simulink model "lagrange_model"  (R2022a)
settings: Solver=ode4  StartTime=0.0  StopTime=10.0  FixedStep=0.01  RelTol=1e-3
undefined symbols (not defined in the file or in its folder): DiscIntNeverNeededParam
(part 3 of 5)

== matlab function lagrange_model/MATLAB Function ==
  data: u1 input; th1dd output; u2 input double; u3 input; u4 input; u5 input; th1d input; th2d input; th3d input; th4d input; th5d input; th2dd output; th3dd output; th4dd output; th5dd output; th1 input; th2 input; th3 input; th4 input; th5 input; th1dd input; th2dd input; th3dd input; th4dd input; th5dd input
function [th1dd, th2dd, th3dd, th4dd, th5dd]= fcn(u1, u2, u3, u4, u5, th1d, th2d, th3d, th4d, th5d, th1, th2, th3, th4, th5, th1dd, th2dd, th3dd, th4dd, th5dd)

l1 = 0.135; 
l2 = 0.38;
l3 = 0.38;
l4 = 0.38;
l5 = 0.04;

m1 = 2.24036308689963;
m2 = 1.38058358126134;
m3 = 0.492773406896242;
m4 = 1.38058358126134;
m5 = 0.130378439395373;
delta = 0.0873;
l1_Izz = 0.0098329939500295;
l2_Izz = 0.0425687229272136;
l3_Izz = 0.00857639886635598;
l4_Izz = 0.0422407814003671;
l5_Izz = 0.0001866513337855;

g = 9.81;
beta1 = 0.3;
beta2 = 0.1;
beta3 = 0.1;
beta4 = 0.1;
beta5 = 0.1;

eq1 = l1_Izz*diff(th1(t), t, t) + l2_Izz*diff(th1(t), t, t) + l3_Izz*diff(th1(t), t, t) + l4_Izz*diff(th1(t), t, t) + l5_Izz*diff(th1(t), t, t) + beta1*diff(th1(t), t) + (l2^2*m2*cos(th1(t))^2*cos(th2(t))^2*diff(th1(t), t, t))/4 + l2^2*m3*cos(th1(t))^2*cos(th2(t))^2*diff(th1(t), t, t) + l2^2*m4*cos(th1(t))^2*cos(th2(t))^2*diff(th1(t), t, t) + l2^2*m5*cos(th1(t))^2*cos(th2(t))^2*diff(th1(t), t, t) + (l2^2*m2*cos(th2(t))^2*sin(th1(t))^2*diff(th1(t), t, t))/4 + l2^2*m3*cos(th2(t))^2*sin(th1(t))^2*diff(th1(t), t, t) + l2^2*m4*cos(th2(t))^2*sin(th1(t))^2*diff(th1(t), t, t) + l2^2*m5*cos(th2(t))^2*sin(th1(t))^2*diff(th1(t), t, t) + (l3^2*m3*cos(th1(t))^2*cos(th2(t))^2*sin(th3(t))^2*diff(th1(t), t, t))/4 + l3^2*m4*cos(th1(t))^2*cos(th2(t))^2*sin(th3(t))^2*diff(th1(t), t, t) + l3^2*m5*cos(th1(t))^2*cos(th2(t))^2*sin(th3(t))^2*diff(th1(t), t, t) + (l3^2*m3*cos(th2(t))^2*sin(th1(t))^2*sin(th3(t))^2*diff(th1(t), t, t))/4 + l3^2*m4*cos(th2(t))^2*sin(th1(t))^2*sin(th3(t))^2*diff(th1(t), t, t) + l3^2*m5*cos(th2(t))^2*sin(th1(t))^2*sin(th3(t))^2*diff(th1(t), t, t) - (l2^2*m2*cos(th1(t))^2*cos(th2(t))*sin(th2(t))*diff(th1(t), t)*diff(th2(t), t))/2 - 2*l2^2*m3*cos(th1(t))^2*cos(th2(t))*sin(th2(t))*diff(th1(t), t)*diff(th2(t), t) - 2*l2^2*m4*cos(th1(t))^2*cos(th2(t))*sin(th2(t))*diff(th1(t), t)*diff(th2(t), t) - 2*l2^2*m5*cos(th1(t))^2*cos(th2(t))*sin(th2(t))*diff(th1(t), t)*diff(th2(t), t) - (l2^2*m2*cos(th2(t))*sin(th1(t))^2*sin(th2(t))*diff(th1(t), t)*diff(th2(t), t))/2 - 2*l2^2*m3*cos(th2(t))*sin(th1(t))^2*sin(th2(t))*diff(th1(t), t)*diff(th2(t), t) - 2*l2^2*m4*cos(th2(t))*sin(th1(t))^2*sin(th2(t))*diff(th1(t), t)*diff(th2(t), t) - 2*l2^2*m5*cos(th2(t))*sin(th1(t))^2*sin(th2(t))*diff(th1(t), t)*diff(th2(t), t) + l2*l3*m3*cos(th1(t))^2*cos(th2(t))^2*sin(th3(t))*diff(th1(t), t, t) + 2*l2*l3*m4*cos(th1(t))^2*cos(th2(t))^2*sin(th3(t))*diff(th1(t), t, t) + 2*l2*l3*m5*cos(th1(t))^2*cos(th2(t))^2*sin(th3(t))*diff(th1(t), t, t) - (l4^2*m5*cos(th1(t))^2*cos(th2(t))^2*sin(th3(t))^2*cos(delta - th4(t))^2*diff(th1(t), t)^2)/4 - (l4^2*m5*cos(th1(t))^2*cos(th2(t))^2*sin(th3(t))^2*cos(delta - th4(t))^2*diff(th2(t), t)^2)/4 - (l4^2*m5*cos(th1(t))^2*cos(th2(t))^2*sin(th3(t))^2*cos(delta - th4(t))^2*diff(th3(t), t)^2)/4 - (l4^2*m5*cos(th1(t))^2*cos(th2(t))^2*sin(th3(t))^2*cos(delta - th4(t))^2*diff(th4(t), t)^2)/4 + l2*l3*m3*cos(th2(t))^2*sin(th1(t))^2*sin(th3(t))*diff(th1(t), t, t) + 2*l2*l3*m4*cos(th2(t))^2*sin(th1(t))^2*sin(th3(t))*diff(th1(t), t, t) + 2*l2*l3*m5*cos(th2(t))^2*sin(th1(t))^2*sin(th3(t))*diff(th1(t), t, t) + (l4^2*m5*cos(th2(t))^2*sin(th1(t))^2*sin(th3(t))^2*cos(delta - th4(t))^2*diff(th1(t), t)^2)/4 + (l4^2*m5*cos(th2(t))^2*sin(th1(t))^2*sin(th3(t))^2*cos(delta - th4(t))^2*diff(th2(t), t)^2)/4 + (l4^2*m5*cos(th2(t))^2*sin(th1(t))^2*sin(th3(t))^2*cos(delta - th4(t))^2*diff(th3(t), t)^2)/4 + (l4^2*m5*cos(th2(t))^2*sin(th1(t))^2*sin(th3(t))^2*cos(delta - th4(t))^2*diff(th4(t), t)^2)/4 + (l4^2*m5*cos(th1(t))^2*cos(th2(t))^2*sin(th3(t))^2*cos(delta - th4(t))^2*diff(th1(t), t, t))/4 + (l4^2*m4*cos(th2(t))^2*sin(th1(t))^2*sin(th3(t))^2*cos(delta - th4(t))^2*diff(th1(t), t, t))/2 + (5*l4^2*m5*cos(th2(t))^2*sin(th1(t))^2*sin(th3(t))^2*cos(delta - th4(t))^2*diff(th1(t), t, t))/4 - l2*l4*m4*cos(th2(t))^2*sin(th1(t))^2*sin(th3(t))*cos(delta - th4(t))*diff(th1(t), t, t) - 2*l2*l4*m5*cos(th2(t))^2*sin(th1(t))^2*sin(th3(t))*cos(delta - th4(t))*diff(th1(t), t, t) + (l2*l4*m4*cos(th1(t))^2*cos(th2(t))^2*sin(th3(t))*sin(delta - th4(t))*diff(th4(t), t, t))/2 + (l2*l4*m5*cos(th1(t))^2*cos(th2(t))^2*sin(th3(t))*sin(delta - th4(t))*diff(th4(t), t, t))/2 + (l3^2*m3*cos(th1(t))^2*cos(th2(t))^2*cos(th3(t))*sin(th3(t))*diff(th1(t), t)*diff(th3(t), t))/2 + 2*l3^2*m4*cos(th1(t))^2*cos(th2(t))^2*cos(th3(t))*sin(th3(t))*diff(th1(t), t)*diff(th3(t), t) + 2*l3^2*m5*cos(th1(t))^2*cos(th2(t))^2*cos(th3(t))*sin(th3(t))*diff(th1(t), t)*diff(th3(t), t) - (l3^2*m3*cos(th1(t))^2*cos(th2(t))*sin(th2(t))*sin(th3(t))^2*diff(th1(t), t)*diff(th2(t), t))/2 - 2*l3^2*m4*cos(th1(t))^2*cos(th2(t))*sin(th2(t))*sin(th3(t))^2*diff(th1(t), t)*diff(th2(t), t) + (l3^2*m3*cos(th2(t))^2*cos(th3(t))*sin(th1(t))^2*sin(th3(t))*diff(th1(t), t)*diff(th3(t), t))/2 - 2*l3^2*m5*cos(th1(t))^2*cos(th2(t))*sin(th2(t))*sin(th3(t))^2*diff(th1(t), t)*diff(th2(t), t) + 2*l3^2*m4*cos(th2(t))^2*cos(th3(t))*sin(th1(t))^2*sin(th3(t))*diff(th1(t), t)*diff(th3(t), t) + 2*l3^2*m5*cos(th2(t))^2*cos(th3(t))*sin(th1(t))^2*sin(th3(t))*diff(th1(t), t)*diff(th3(t), t) - (l3^2*m3*cos(th2(t))*sin(th1(t))^2*sin(th2(t))*sin(th3(t))^2*diff(th1(t), t)*diff(th2(t), t))/2 - 2*l3^2*m4*cos(th2(t))*sin(th1(t))^2*sin(th2(t))*sin(th3(t))^2*diff(th1(t), t)*diff(th2(t), t) - 2*l3^2*m5*cos(th2(t))*sin(th1(t))^2*sin(th2(t))*sin(th3(t))^2*diff(th1(t), t)*diff(th2(t), t) - (l3*l4*m4*cos(th1(t))^2*cos(th2(t))^2*sin(th3(t))^2*cos(delta - th4(t))*diff(th1(t), t)^2)/2 - (l3*l4*m4*cos(th1(t))^2*cos(th2(t))^2*sin(th3(t))^2*cos(delta - th4(t))*diff(th2(t), t)^2)/2 - (l3*l4*m5*cos(th1(t))^2*cos(th2(t))^2*sin(th3(t))^2*cos(delta - th4(t))*diff(th1(t), t)^2)/2 - (l3*l4*m4*cos(th1(t))^2*cos(th2(t))^2*sin(th3(t))^2*cos(delta - th4(t))*diff(th3(t), t)^2)/2 - (l3*l4*m5*cos(th1(t))^2*cos(th2(t))^2*sin(th3(t))^2*cos(delta - th4(t))*diff(th2(t), t)^2)/2 - (l3*l4*m4*cos(th1(t))^2*cos(th2(t))^2*sin(th3(t))^2*cos(delta - th4(t))*diff(th4(t), t)^2)/2 - (l3*l4*m5*cos(th1(t))^2*cos(th2(t))^2*sin(th3(t))^2*cos(delta - th4(t))*diff(th3(t), t)^2)/2 - (l3*l4*m5*cos(th1(t))^2*cos(th2(t))^2*sin(th3(t))^2*cos(delta - th4(t))*diff(th4(t), t)^2)/2 + (l3*l4*m4*cos(th2(t))^2*sin(th1(t))^2*sin(th3(t))^2*cos(delta - th4(t))*diff(th1(t), t)^2)/2 + (l3*l4*m4*cos(th2(t))^2*sin(th1(t))^2*sin(th3(t))^2*cos(delta - th4(t))*diff(th2(t), t)^2)/2 + (l3*l4*m5*cos(th2(t))^2*sin(th1(t))^2*sin(th3(t))^2*cos(delta - th4(t))*diff(th1(t), t)^2)/2 + (l3*l4*m4*cos(th2(t))^2*sin(th1(t))^2*sin(th3(t))^2*cos(delta - th4(t))*diff(th3(t), t)^2)/2 + (l3*l4*m5*cos(th2(t))^2*sin(th1(t))^2*sin(th3(t))^2*cos(delta - th4(t))*diff(th2(t), t)^2)/2 + (l3*l4*m5*cos(th2(t))^2*sin(th1(t))^2*sin(th3(t))^2*cos(delta - th4(t))*diff(th3(t), t)^2)/2 + (l5^2*m5*cos(th1(t))^2*cos(th2(t))^2*cos(th5(t))^2*sin(th3(t))^2*cos(delta - th4(t))^2*diff(th1(t), t, t))/4 + l3*l4*m5*cos(th1(t))^2*cos(th2(t))^2*sin(th3(t))^2*cos(delta - th4(t))*diff(th1(t), t, t) + (l5^2*m5*cos(th2(t))^2*cos(th5(t))^2*sin(th1(t))^2*sin(th3(t))^2*cos(delta - th4(t))^2*diff(th1(t), t, t))/4 - l3*l4*m4*cos(th2(t))^2*sin(th1(t))^2*sin(th3(t))^2*cos(delta - th4(t))*diff(th1(t), t, t) - 2*l3*l4*m5*cos(th2(t))^2*sin(th1(t))^2*sin(th3(t))^2*cos(delta - th4(t))*diff(th1(t), t, t) + (l3*l4*m4*cos(th1(t))^2*cos(th2(t))^2*sin(th3(t))^2*sin(delta - th4(t))*diff(th4(t), t, t))/2 + (l3*l4*m5*cos(th1(t))^2*cos(th2(t))^2*sin(th3(t))^2*sin(delta - th4(t))*diff(th4(t), t, t))/2 + (l4^2*m4*cos(th1(t))*cos(th2(t))^2*sin(th1(t))*sin(th3(t))^2*cos(delta - th4(t))^2*diff(th1(t), t)^2)/2 + (l4^2*m4*cos(th1(t))*cos(th2(t))^2*sin(th1(t))*sin(th3(t))^2*cos(delta - th4(t))^2*diff(th2(t), t)^2)/2 + l4^2*m5*cos(th1(t))*cos(th2(t))^2*sin(th1(t))*sin(th3(t))^2*cos(delta - th4(t))^2*diff(th1(t), t)^2 + (l4^2*m4*cos(th1(t))*cos(th2(t))^2*sin(th1(t))*sin(th3(t))^2*cos(delta - th4(t))^2*diff(th3(t), t)^2)/2 + l4^2*m5*cos(th1(t))*cos(th2(t))^2*sin(th1(t))*sin(th3(t))^2*cos(delta - th4(t))^2*diff(th2(t), t)^2 + (l4^2*m4*cos(th1(t))*cos(th2(t))^2*sin(th1(t))*sin(th3(t))^2*cos(delta - th4(t))^2*diff(th4(t), t)^2)/2 + l4^2*m5*cos(th1(t))*cos(th2(t))^2*sin(th1(t))*sin(th3(t))^2*cos(delta - th4(t))^2*diff(th3(t), t)^2 + l4^2*m5*cos(th1(t))*cos(th2(t))^2*sin(th1(t))*sin(th3(t))^2*cos(delta - th4(t))^2*diff(th4(t), t)^2 + (l4^2*m5*cos(th1(t))^2*cos(th2(t))^2*cos(th3(t))*sin(th3(t))*cos(delta - th4(t))^2*diff(th3(t), t, t))/4 - (l4^2*m5*cos(th1(t))*cos(th2(t))^2*sin(th1(t))*sin(th3(t))^2*cos(delta - th4(t))^2*diff(th1(t), t, t))/2 - (l4^2*m5*cos(th1(t))^2*cos(th2(t))*sin(th2(t))*sin(th3(t))^2*cos(delta - th4(t))^2*diff(th2(t), t, t))/4 - (l4^2*m5*cos(th2(t))^2*cos(th3(t))*sin(th1(t))^2*sin(th3(t))*cos(delta - th4(t))^2*diff(th3(t), t, t))/4 + (l4^2*m5*cos(th2(t))*sin(th1(t))^2*sin(th2(t))*sin(th3(t))^2*cos(delta - th4(t))^2*diff(th2(t), t, t))/4 + l2*l3*m3*cos(th1(t))^2*cos(th2(t))^2*cos(th3(t))*diff(th1(t), t)*diff(th3(t), t) + 2*l2*l3*m4*cos(th1(t))^2*cos(th2(t))^2*cos(th3(t))*diff(th1(t), t)*diff(th3(t), t) + 2*l2*l3*m5*cos(th1(t))^2*cos(th2(t))^2*cos(th3(t))*diff(th1(t), t)*diff(th3(t), t) + (l4^2*m5*cos(th1(t))^2*cos(th2(t))^2*sin(th3(t))^2*cos(delta - th4(t))*sin(delta - th4(t))*diff(th4(t), t, t))/4 + l2*l3*m3*cos(th2(t))^2*cos(th3(t))*sin(th1(t))^2*diff(th1(t), t)*diff(th3(t), t) + 2*l2*l3*m4*cos(th2(t))^2*cos(th3(t))*sin(th1(t))^2*diff(th1(t), t)*diff(th3(t), t) + 2*l2*l3*m5*cos(th2(t))^2*cos(th3(t))*sin(th1(t))^2*diff(th1(t), t)*diff(th3(t), t) - (l4^2*m5*cos(th2(t))^2*sin(th1(t))^2*sin(th3(t))^2*cos(delta - th4(t))*sin(delta - th4(t))*diff(th4(t), t, t))/4 - (l2*l4*m4*cos(th1(t))^2*cos(th2(t))^2*sin(th3(t))*cos(delta - th4(t))*diff(th1(t), t)^2)/2 - (l2*l4*m4*cos(th1(t))^2*cos(th2(t))^2*sin(th3(t))*cos(delta - th4(t))*diff(th2(t), t)^2)/2 - (l2*l4*m5*cos(th1(t))^2*cos(th2(t))^2*sin(th3(t))*cos(delta - th4(t))*diff(th1(t), t)^2)/2 - (l2*l4*m4*cos(th1(t))^2*cos(th2(t))^2*sin(th3(t))*cos(delta - th4(t))*diff(th3(t), t)^2)/2 - (l2*l4*m5*cos(th1(t))^2*cos(th2(t))^2*sin(th3(t))*cos(delta - th4(t))*diff(th2(t), t)^2)/2 - (l2*l4*m4*cos(th1(t))^2*cos(th2(t))^2*sin(th3(t))*cos(delta - th4(t))*diff(th4(t), t)^2)/2 - (l2*l4*m5*cos(th1(t))^2*cos(th2(t))^2*sin(th3(t))*cos(delta - th4(t))*diff(th3(t), t)^2)/2 - (l2*l4*m5*cos(th1(t))^2*cos(th2(t))^2*sin(th3(t))*cos(delta - th4(t))*diff(th4(t), t)^2)/2 + (l2*l4*m4*cos(th1(t))^2*cos(th2(t))^2*cos(th3(t))*cos(delta - th4(t))*diff(th3(t), t, t))/2 + (l2*l4*m5*cos(th1(t))^2*cos(th2(t))^2*cos(th3(t))*cos(delta - th4(t))*diff(th3(t), t, t))/2 + (l2*l4*m4*cos(th2(t))^2*sin(th1(t))^2*sin(th3(t))*cos(delta - th4(t))*diff(th1(t), t)^2)/2 + (l2*l4*m4*cos(th2(t))^2*sin(th1(t))^2*sin(th3(t))*cos(delta - th4(t))*diff(th2(t), t)^2)/2 + (l2*l4*m5*cos(th2(t))^2*sin(th1(t))^2*sin(th3(t))*cos(delta - th4(t))*diff(th1(t), t)^2)/2 + (l2*l4*m5*cos(th2(t))^2*sin(th1(t))^2*sin(th3(t))*cos(delta - th4(t))*diff(th2(t), t)^2)/2 + l2*l4*m5*cos(th1(t))^2*cos(th2(t))^2*sin(th3(t))*cos(delta - th4(t))*diff(th1(t), t, t) + (l4*l5*m5*cos(th2(t))^2*cos(th5(t))*sin(th1(t))^2*sin(th3(t))^2*cos(delta - th4(t))^2*diff(th1(t), t)^2)/4 + (l4*l5*m5*cos(th2(t))^2*cos(th5(t))*sin(th1(t))^2*sin(th3(t))^2*cos(delta - th4(t))^2*diff(th2(t), t)^2)/4 + (l4*l5*m5*cos(th2(t))^2*cos(th5(t))*sin(th1(t))^2*sin(th3(t))^2*cos(delta - th4(t))^2*diff(th3(t), t)^2)/4 + (l4*l5*m5*cos(th2(t))^2*cos(th5(t))*sin(th1(t))^2*sin(th3(t))^2*cos(delta - th4(t))^2*diff(th4(t), t)^2)/4 + (l4*l5*m5*cos(th2(t))^2*cos(th5(t))*sin(th1(t))^2*sin(th3(t))^2*cos(delta - th4(t))^2*diff(th5(t), t)^2)/4 + (l4*l5*m5*cos(th1(t))^2*cos(th2(t))^2*cos(th5(t))*sin(th3(t))^2*cos(delta - th4(t))^2*diff(th1(t), t, t))/2 - l4^2*m4*cos(th2(t))*sin(th1(t))^2*sin(th2(t))*sin(th3(t))^2*cos(delta - th4(t))^2*diff(th1(t), t)*diff(th2(t), t) - (5*l4^2*m5*cos(th2(t))*sin(th1(t))^2*sin(th2(t))*sin(th3(t))^2*cos(delta - th4(t))^2*diff(th1(t), t)*diff(th2(t), t))/2 + (l2*l4*m4*cos(th2(t))*sin(th1(t))^2*sin(th2(t))*sin(th3(t))*cos(delta - th4(t))*diff(th2(t), t, t))/2 + (l2*l4*m4*cos(th1(t))*cos(th2(t))^2*sin(th1(t))*sin(th3(t))*sin(delta - th4(t))*diff(th4(t), t, t))/2 + (l2*l4*m5*cos(th2(t))*sin(th1(t))^2*sin(th2(t))*sin(th3(t))*cos(delta - th4(t))*diff(th2(t), t, t))/2 + (3*l2*l4*m5*cos(th1(t))*cos(th2(t))^2*sin(th1(t))*sin(th3(t))*sin(delta - th4(t))*diff(th4(t), t, t))/2 + l4*l5*m5*cos(th2(t))^2*cos(th5(t))*sin(th1(t))^2*sin(th3(t))^2*cos(delta - th4(t))^2*diff(th1(t), t, t) + (l4^2*m5*cos(th1(t))^2*cos(th2(t))^2*sin(th3(t))^2*cos(delta - th4(t))*sin(delta - th4(t))*diff(th1(t), t)*diff(th4(t), t))/2 + (l4*l5*m5*cos(th2(t))^2*sin(th1(t))^2*sin(th3(t))^2*sin(th5(t))*cos(delta - th4(t))^2*diff(th5(t), t, t))/4 + l4^2*m4*cos(th2(t))^2*sin(th1(t))^2*sin(th3(t))^2*cos(delta - th4(t))*sin(delta - th4(t))*diff(th1(t), t)*diff(th4(t), t) + (5*l4^2*m5*cos(th2(t))^2*sin(th1(t))^2*sin(th3(t))^2*cos(delta - th4(t))*sin(delta - th4(t))*diff(th1(t), t)*diff(th4(t), t))/2 + l2*l4*m5*cos(th1(t))^2*cos(th2(t))^2*cos(th3(t))*cos(delta - th4(t))*diff(th1(t), t)*diff(th3(t), t) - l3*l4*m4*cos(th1(t))*cos(th2(t))^2*sin(th1(t))*sin(th3(t))^2*cos(delta - th4(t))*diff(th1(t), t)^2 - l3*l4*m4*cos(th1(t))*cos(th2(t))^2*sin(th1(t))*sin(th3(t))^2*cos(delta - th4(t))*diff(th2(t), t)^2 - 3*l3*l4*m5*cos(th1(t))*cos(th2(t))^2*sin(th1(t))*sin(th3(t))^2*cos(delta - th4(t))*diff(th1(t), t)^2 - l3*l4*m4*cos(th1(t))*cos(th2(t))^2*sin(th1(t))*sin(th3(t))^2*cos(delta - th4(t))*diff(th3(t), t)^2 - 3*l3*l4*m5*cos(th1(t))*cos(th2(t))^2*sin(th1(t))*sin(th3(t))^2*cos(delta - th4(t))*diff(th2(t), t)^2 - (l3*l4*m4*cos(th1(t))*cos(th2(t))^2*sin(th1(t))*sin(th3(t))^2*cos(delta - th4(t))*diff(th4(t), t)^2)/2 - 3*l3*l4*m5*cos(th1(t))*cos(th2(t))^2*sin(th1(t))*sin(th3(t))^2*cos(delta - th4(t))*diff(th3(t), t)^2 - (3*l3*l4*m5*cos(th1(t))*cos(th2(t))^2*sin(th1(t))*sin(th3(t))^2*cos(delta - th4(t))*diff(th4(t), t)^2)/2 + (l3*l4*m4*cos(th1(t))^2*cos(th2(t))^2*cos(th3(t))*sin(th3(t))*cos(delta - th4(t))*diff(th3(t), t, t))/2 + l2*l5*m5*cos(th1(t))^2*cos(th2(t))^2*cos(th5(t))*sin(th3(t))*cos(delta - th4(t))*diff(th1(t), t, t) + (l3*l4*m5*cos(th1(t))^2*cos(th2(t))^2*cos(th3(t))*sin(th3(t))*cos(delta - th4(t))*diff(th3(t), t, t))/2 - l2*l4*m4*cos(th2(t))^2*cos(th3(t))*sin(th1(t))^2*cos(delta - th4(t))*diff(th1(t), t)*diff(th3(t), t) - 2*l2*l4*m5*cos(th2(t))^2*cos(th3(t))*sin(th1(t))^2*cos(delta - th4(t))*diff(th1(t), t)*diff(th3(t), t) + l2*l4*m4*cos(th1(t))^2*cos(th2(t))^2*cos(th3(t))*sin(delta - th4(t))*diff(th3(t), t)*diff(th4(t), t) + l2*l4*m5*cos(th1(t))^2*cos(th2(t))^2*cos(th3(t))*sin(delta - th4(t))*diff(th3(t), t)*diff(th4(t), t) - l3*l4*m4*cos(th1(t))*cos(th2(t))^2*sin(th1(t))*sin(th3(t))^2*cos(delta - th4(t))*diff(th1(t), t, t) - l3*l4*m5*cos(th1(t))*cos(th2(t))^2*sin(th1(t))*sin(th3(t))^2*cos(delta - th4(t))*diff(th1(t), t, t) - (l3*l4*m4*cos(th1(t))^2*cos(th2(t))*sin(th2(t))*sin(th3(t))^2*cos(delta - th4(t))*diff(th2(t), t, t))/2 - (l3*l4*m5*cos(th1(t))^2*cos(th2(t))*sin(th2(t))*sin(th3(t))^2*cos(delta - th4(t))*diff(th2(t), t, t))/2 - (l3*l4*m4*cos(th2(t))^2*cos(th3(t))*sin(th1(t))^2*sin(th3(t))*cos(delta - th4(t))*diff(th3(t), t, t))/2 - l2*l5*m5*cos(th2(t))^2*cos(th5(t))*sin(th1(t))^2*sin(th3(t))*cos(delta - th4(t))*diff(th1(t), t, t) - (l3*l4*m5*cos(th2(t))^2*cos(th3(t))*sin(th1(t))^2*sin(th3(t))*cos(delta - th4(t))*diff(th3(t), t, t))/2 + l2*l4*m5*cos(th1(t))^2*cos(th2(t))^2*sin(th3(t))*sin(delta - th4(t))*diff(th1(t), t)*diff(th4(t), t) + (l3*l4*m4*cos(th2(t))*sin(th1(t))^2*sin(th2(t))*sin(th3(t))^2*cos(delta - th4(t))*diff(th2(t), t, t))/2 + (l3*l4*m4*cos(th1(t))*cos(th2(t))^2*sin(th1(t))*sin(th3(t))^2*sin(delta - th4(t))*diff(th4(t), t, t))/2 + (l3*l4*m5*cos(th2(t))*sin(th1(t))^2*sin(th2(t))*sin(th3(t))^2*cos(delta - th4(t))*diff(th2(t), t, t))/2 + (3*l3*l4*m5*cos(th1(t))*cos(th2(t))^2*sin(th1(t))*sin(th3(t))^2*sin(delta - th4(t))*diff(th4(t), t, t))/2 - l2*l4*m4*cos(th2(t))^2*sin(th1(t))^2*sin(th3(t))*sin(delta - th4(t))*diff(th1(t), t)*diff(th4(t), t) - 2*l2*l4*m5*cos(th2(t))^2*sin(th1(t))^2*sin(th3(t))*sin(delta - th4(t))*diff(th1(t), t)*diff(th4(t), t) - (l4^2*m4*cos(th1(t))*cos(th2(t))^2*cos(th3(t))*sin(th1(t))*sin(th3(t))*cos(delta - th4(t))^2*diff(th3(t), t, t))/2 - l4^2*m5*cos(th1(t))*cos(th2(t))^2*cos(th3(t))*sin(th1(t))*sin(th3(t))*cos(delta - th4(t))^2*diff(th3(t), t, t) + (l4^2*m4*cos(th1(t))*cos(th2(t))*sin(th1(t))*sin(th2(t))*sin(th3(t))^2*cos(delta - th4(t))^2*diff(th2(t), t, t))/2 + l4^2*m5*cos(th1(t))*cos(th2(t))*sin(th1(t))*sin(th2(t))*sin(th3(t))^2*cos(delta - th4(t))^2*diff(th2(t), t, t) + l3*l5*m5*cos(th1(t))^2*cos(th2(t))^2*cos(th5(t))*sin(th3(t))^2*cos(delta - th4(t))*diff(th1(t), t, t) - l3*l5*m5*cos(th2(t))^2*cos(th5(t))*sin(th1(t))^2*sin(th3(t))^2*cos(delta - th4(t))*diff(th1(t), t, t) + l3*l4*m5*cos(th1(t))^2*cos(th2(t))^2*sin(th3(t))^2*sin(delta - th4(t))*diff(th1(t), t)*diff(th4(t), t) - l3*l4*m4*cos(th2(t))^2*sin(th1(t))^2*sin(th3(t))^2*sin(delta - th4(t))*diff(th1(t), t)*diff(th4(t), t) - 2*l3*l4*m5*cos(th2(t))^2*sin(th1(t))^2*sin(th3(t))^2*sin(delta - th4(t))*diff(th1(t), t)*diff(th4(t), t) - (l4^2*m4*cos(th1(t))*cos(th2(t))^2*sin(th1(t))*sin(th3(t))^2*cos(delta - th4(t))*sin(delta - th4(t))*diff(th4(t), t, t))/2 - l4^2*m5*cos(th1(t))*cos(th2(t))^2*sin(th1(t))*sin(th3(t))^2*cos(delta - th4(t))*sin(delta - th4(t))*diff(th4(t), t, t) - 2*l2*l3*m3*cos(th1(t))^2*cos(th2(t))*sin(th2(t))*sin(th3(t))*diff(th1(t), t)*diff(th2(t), t) - 4*l2*l3*m4*cos(th1(t))^2*cos(th2(t))*sin(th2(t))*sin(th3(t))*diff(th1(t), t)*diff(th2(t), t) - 4*l2*l3*m5*cos(th1(t))^2*cos(th2(t))*sin(th2(t))*sin(th3(t))*diff(th1(t), t)*diff(th2(t), t) - l2*l4*m4*cos(th1(t))*cos(th2(t))^2*sin(th1(t))*sin(th3(t))*cos(delta - th4(t))*diff(th1(t), t)^2 - l2*l4*m4*cos(th1(t))*cos(th2(t))^2*sin(th1(t))*sin(th3(t))*cos(delta - th4(t))*diff(th2(t), t)^2 - 3*l2*l4*m5*cos(th1(t))*cos(th2(t))^2*sin(th1(t))*sin(th3(t))*cos(delta - th4(t))*diff(th1(t), t)^2 - (l2*l4*m4*cos(th1(t))*cos(th2(t))^2*sin(th1(t))*sin(th3(t))*cos(delta - th4(t))*diff(th3(t), t)^2)/2 - 3*l2*l4*m5*cos(th1(t))*cos(th2(t))^2*sin(th1(t))*sin(th3(t))*cos(delta - th4(t))*diff(th2(t), t)^2 - (l2*l4*m4*cos(th1(t))*cos(th2(t))^2*sin(th1(t))*sin(th3(t))*cos(delta - th4(t))*diff(th4(t), t)^2)/2 - (3*l2*l4*m5*cos(th1(t))*cos(th2(t))^2*sin(th1(t))*sin(th3(t))*cos(delta - th4(t))*diff(th3(t), t)^2)/2 - (3*l2*l4*m5*cos(th1(t))*cos(th2(t))^2*sin(th1(t))*sin(th3(t))*cos(delta - th4(t))*diff(th4(t), t)^2)/2 - 2*l2*l3*m3*cos(th2(t))*sin(th1(t))^2*sin(th2(t))*sin(th3(t))*diff(th1(t), t)*diff(th2(t), t) - 4*l2*l3*m4*cos(th2(t))*sin(th1(t))^2*sin(th2(t))*sin(th3(t))*diff(th1(t), t)*diff(th2(t), t) - 4*l2*l3*m5*cos(th2(t))*sin(th1(t))^2*sin(th2(t))*sin(th3(t))*diff(th1(t), t)*diff(th2(t), t) + (l4^2*m5*cos(th1(t))^2*cos(th2(t))^2*cos(th3(t))*sin(th3(t))*cos(delta - th4(t))^2*diff(th1(t), t)*diff(th3(t), t))/2 + (l2*l4*m4*cos(th1(t))*cos(th2(t))^2*cos(th3(t))*sin(th1(t))*cos(delta - th4(t))*diff(th3(t), t, t))/2 + (3*l2*l4*m5*cos(th1(t))*cos(th2(t))^2*cos(th3(t))*sin(th1(t))*cos(delta - th4(t))*diff(th3(t), t, t))/2 - (l4*l5*m5*cos(th1(t))^2*cos(th2(t))^2*cos(th5(t))*sin(th3(t))^2*cos(delta - th4(t))^2*diff(th1(t), t)^2)/4 - (l4*l5*m5*cos(th1(t))^2*cos(th2(t))^2*cos(th5(t))*sin(th3(t))^2*cos(delta - th4(t))^2*diff(th2(t), t)^2)/4 - (l4*l5*m5*cos(th1(t))^2*cos(th2(t))^2*cos(th5(t))*sin(th3(t))^2*cos(delta - th4(t))^2*diff(th3(t), t)^2)/4 - (l4*l5*m5*cos(th1(t))^2*cos(th2(t))^2*cos(th5(t))*sin(th3(t))^2*cos(delta - th4(t))^2*diff(th4(t), t)^2)/4 - (l4^2*m5*cos(th1(t))^2*cos(th2(t))*sin(th2(t))*sin(th3(t))^2*cos(delta - th4(t))^2*diff(th1(t), t)*diff(th2(t), t))/2 + l4^2*m4*cos(th2(t))^2*cos(th3(t))*sin(th1(t))^2*sin(th3(t))*cos(delta - th4(t))^2*diff(th1(t), t)*diff(th3(t), t) + (5*l4^2*m5*cos(th2(t))^2*cos(th3(t))*sin(th1(t))^2*sin(th3(t))*cos(delta - th4(t))^2*diff(th1(t), t)*diff(th3(t), t))/2 - l2*l4*m4*cos(th1(t))*cos(th2(t))^2*sin(th1(t))*sin(th3(t))*cos(delta - th4(t))*diff(th1(t), t, t) - l2*l4*m5*cos(th1(t))*cos(th2(t))^2*sin(th1(t))*sin(th3(t))*cos(delta - th4(t))*diff(th1(t), t, t) - (l2*l4*m4*cos(th1(t))^2*cos(th2(t))*sin(th2(t))*sin(th3(t))*cos(delta - th4(t))*diff(th2(t), t, t))/2 - (l2*l4*m5*cos(th1(t))^2*cos(th2(t))*sin(th2(t))*sin(th3(t))*cos(delta - th4(t))*diff(th2(t), t, t))/2 - (l4*l5*m5*cos(th1(t))*cos(th2(t))^2*cos(th5(t))*sin(th1(t))*sin(th3(t))^2*cos(delta - th4(t))^2*diff(th1(t), t, t))/2 - (l4*l5*m5*cos(th1(t))^2*cos(th2(t))*cos(th5(t))*sin(th2(t))*sin(th3(t))^2*cos(delta - th4(t))^2*diff(th2(t), t, t))/4 - (l4*l5*m5*cos(th2(t))^2*cos(th3(t))*cos(th5(t))*sin(th1(t))^2*sin(th3(t))*cos(delta - th4(t))^2*diff(th3(t), t, t))/4 + l3*l5*m5*cos(th1(t))^2*cos(th2(t))^2*cos(th5(t))*sin(th3(t))^2*sin(delta - th4(t))*diff(th1(t), t)*diff(th4(t), t) - l3*l5*m5*cos(th1(t))^2*cos(th2(t))^2*sin(th3(t))^2*sin(th5(t))*cos(delta - th4(t))*diff(th1(t), t)*diff(th5(t), t) + (l4^2*m5*cos(th1(t))^2*cos(th2(t))^2*cos(th3(t))*sin(th3(t))*cos(delta - th4(t))*sin(delta - th4(t))*diff(th3(t), t)*diff(th4(t), t))/2 + (l4*l5*m5*cos(th2(t))*cos(th5(t))*sin(th1(t))^2*sin(th2(t))*sin(th3(t))^2*cos(delta - th4(t))^2*diff(th2(t), t, t))/4 + (l4*l5*m5*cos(th1(t))*cos(th2(t))^2*sin(th1(t))*sin(th3(t))^2*sin(th5(t))*cos(delta - th4(t))^2*diff(th5(t), t, t))/4 - l3*l5*m5*cos(th2(t))^2*cos(th5(t))*sin(th1(t))^2*sin(th3(t))^2*sin(delta - th4(t))*diff(th1(t), t)*diff(th4(t), t) + l3*l5*m5*cos(th2(t))^2*sin(th1(t))^2*sin(th3(t))^2*sin(th5(t))*cos(delta - th4(t))*diff(th1(t), t)*diff(th5(t), t) - l4^2*m5*cos(th1(t))*cos(th2(t))^2*sin(th1(t))*sin(th3(t))^2*cos(delta - th4(t))*sin(delta - th4(t))*diff(th1(t), t)*diff(th4(t), t) - (l4^2*m5*cos(th1(t))^2*cos(th2(t))*sin(th2(t))*sin(th3(t))^2*cos(delta - th4(t))*sin(delta - th4(t))*diff(th2(t), t)*diff(th4(t), t))/2 - (l4^2*m5*cos(th2(t))^2*cos(th3(t))*sin(th1(t))^2*sin(th3(t))*cos(delta - th4(t))*sin(delta - th4(t))*diff(th3(t), t)*diff(th4(t), t))/2 + (l4*l5*m5*cos(th1(t))^2*cos(th2(t))^2*cos(th5(t))*sin(th3(t))^2*cos(delta - th4(t))*sin(delta - th4(t))*diff(th4(t), t, t))/4 + (l4^2*m5*cos(th2(t))*sin(th1(t))^2*sin(th2(t))*sin(th3(t))^2*cos(delta - th4(t))*sin(delta - th4(t))*diff(th2(t), t)*diff(th4(t), t))/2 - 2*l2*l5*m5*cos(th1(t))*cos(th2(t))^2*cos(th5(t))*sin(th1(t))*sin(th3(t))*cos(delta - th4(t))*diff(th1(t), t)^2 - 2*l2*l5*m5*cos(th1(t))*cos(th2(t))^2*cos(th5(t))*sin(th1(t))*sin(th3(t))*cos(delta - th4(t))*diff(th2(t), t)^2 - l2*l5*m5*cos(th1(t))*cos(th2(t))^2*cos(th5(t))*sin(th1(t))*sin(th3(t))*cos(delta - th4(t))*diff(th3(t), t)^2 - l2*l5*m5*cos(th1(t))*cos(th2(t))^2*cos(th5(t))*sin(th1(t))*sin(th3(t))*cos(delta - th4(t))*diff(th4(t), t)^2 - l2*l5*m5*cos(th1(t))*cos(th2(t))^2*cos(th5(t))*sin(th1(t))*sin(th3(t))*cos(delta - th4(t))*diff(th5(t), t)^2 + l2*l5*m5*cos(th1(t))*cos(th2(t))^2*cos(th3(t))*cos(th5(t))*sin(th1(t))*cos(delta - th4(t))*diff(th3(t), t, t) - l2*l4*m4*cos(th1(t))*cos(th2(t))^2*cos(th3(t))*sin(th1(t))*cos(delta - th4(t))*diff(th1(t), t)*diff(th3(t), t) - l2*l4*m5*cos(th1(t))*cos(th2(t))^2*cos(th3(t))*sin(th1(t))*cos(delta - th4(t))*diff(th1(t), t)*diff(th3(t), t) - l2*l4*m4*cos(th1(t))^2*cos(th2(t))*cos(th3(t))*sin(th2(t))*cos(delta - th4(t))*diff(th2(t), t)*diff(th3(t), t) - l2*l4*m5*cos(th1(t))^2*cos(th2(t))*cos(th3(t))*sin(th2(t))*cos(delta - th4(t))*diff(th2(t), t)*diff(th3(t), t) - (l4*l5*m5*cos(th2(t))^2*cos(th5(t))*sin(th1(t))^2*sin(th3(t))^2*cos(delta - th4(t))*sin(delta - th4(t))*diff(th4(t), t, t))/4 + l3*l4*m4*cos(th1(t))*cos(th2(t))^2*cos(th3(t))*sin(th1(t))*sin(th3(t))*cos(delta - th4(t))*diff(th3(t), t, t) + 3*l3*l4*m5*cos(th1(t))*cos(th2(t))^2*cos(th3(t))*sin(th1(t))*sin(th3(t))*cos(delta - th4(t))*diff(th3(t), t, t) - 2*l2*l4*m5*cos(th1(t))^2*cos(th2(t))*sin(th2(t))*sin(th3(t))*cos(delta - th4(t))*diff(th1(t), t)*diff(th2(t), t) + l2*l4*m4*cos(th1(t))*cos(th2(t))^2*cos(th3(t))*sin(th1(t))*sin(delta - th4(t))*diff(th3(t), t)*diff(th4(t), t) + 3*l2*l4*m5*cos(th1(t))*cos(th2(t))^2*cos(th3(t))*sin(th1(t))*sin(delta - th4(t))*diff(th3(t), t)*diff(th4(t), t) - l3*l4*m4*cos(th1(t))*cos(th2(t))*sin(th1(t))*sin(th2(t))*sin(th3(t))^2*cos(delta - th4(t))*diff(th2(t), t, t) - 3*l3*l4*m5*cos(th1(t))*cos(th2(t))*sin(th1(t))*sin(th2(t))*sin(th3(t))^2*cos(delta - th4(t))*diff(th2(t), t, t) + l2*l5*m5*cos(th1(t))*cos(th2(t))^2*cos(th5(t))*sin(th1(t))*sin(th3(t))*sin(delta - th4(t))*diff(th4(t), t, t) - l2*l5*m5*cos(th1(t))*cos(th2(t))^2*sin(th1(t))*sin(th3(t))*sin(th5(t))*cos(delta - th4(t))*diff(th5(t), t, t) + 2*l2*l4*m4*cos(th2(t))*sin(th1(t))^2*sin(th2(t))*sin(th3(t))*cos(delta - th4(t))*diff(th1(t), t)*diff(th2(t), t) - l2*l4*m4*cos(th1(t))*cos(th2(t))^2*sin(th1(t))*sin(th3(t))*sin(delta - th4(t))*diff(th1(t), t)*diff(th4(t), t) + 4*l2*l4*m5*cos(th2(t))*sin(th1(t))^2*sin(th2(t))*sin(th3(t))*cos(delta - th4(t))*diff(th1(t), t)*diff(th2(t), t) - l2*l4*m5*cos(th1(t))*cos(th2(t))^2*sin(th1(t))*sin(th3(t))*sin(delta - th4(t))*diff(th1(t), t)*diff(th4(t), t) - l2*l4*m4*cos(th1(t))^2*cos(th2(t))*sin(th2(t))*sin(th3(t))*sin(delta - th4(t))*diff(th2(t), t)*diff(th4(t), t) - l2*l4*m5*cos(th1(t))^2*cos(th2(t))*sin(th2(t))*sin(th3(t))*sin(delta - th4(t))*diff(th2(t), t)*diff(th4(t), t) - (l4*l5*m5*cos(th1(t))^2*cos(th2(t))^2*sin(th3(t))^2*sin(th5(t))*cos(delta - th4(t))^2*diff(th1(t), t)*diff(th5(t), t))/2 - l4*l5*m5*cos(th2(t))^2*sin(th1(t))^2*sin(th3(t))^2*sin(th5(t))*cos(delta - th4(t))^2*diff(th1(t), t)*diff(th5(t), t) + l2*l5*m5*cos(th1(t))^2*cos(th2(t))^2*cos(th3(t))*cos(th5(t))*cos(delta - th4(t))*diff(th1(t), t)*diff(th3(t), t) - 2*l3*l5*m5*cos(th1(t))*cos(th2(t))^2*cos(th5(t))*sin(th1(t))*sin(th3(t))^2*cos(delta - th4(t))*diff(th1(t), t)^2 - 2*l3*l5*m5*cos(th1(t))*cos(th2(t))^2*cos(th5(t))*sin(th1(t))*sin(th3(t))^2*cos(delta - th4(t))*diff(th2(t), t)^2 - 2*l3*l5*m5*cos(th1(t))*cos(th2(t))^2*cos(th5(t))*sin(th1(t))*sin(th3(t))^2*cos(delta - th4(t))*diff(th3(t), t)^2 - l3*l5*m5*cos(th1(t))*cos(th2(t))^2*cos(th5(t))*sin(th1(t))*sin(th3(t))^2*cos(delta - th4(t))*diff(th4(t), t)^2 - l3*l5*m5*cos(th1(t))*cos(th2(t))^2*cos(th5(t))*sin(th1(t))*sin(th3(t))^2*cos(delta - th4(t))*diff(th5(t), t)^2 + (l5^2*m5*cos(th1(t))^2*cos(th2(t))^2*cos(th3(t))*cos(th5(t))^2*sin(th3(t))*cos(delta - th4(t))^2*diff(th1(t), t)*diff(th3(t), t))/2 + 2*l3*l4*m5*cos(th1(t))^2*cos(th2(t))^2*cos(th3(t))*sin(th3(t))*cos(delta - th4(t))*diff(th1(t), t)*diff(th3(t), t) - l2*l5*m5*cos(th2(t))^2*cos(th3(t))*cos(th5(t))*sin(th1(t))^2*cos(delta - th4(t))*diff(th1(t), t)*diff(th3(t), t) - (l5^2*m5*cos(th1(t))^2*cos(th2(t))*cos(th5(t))^2*sin(th2(t))*sin(th3(t))^2*cos(delta - th4(t))^2*diff(th1(t), t)*diff(th2(t), t))/2 + (l5^2*m5*cos(th2(t))^2*cos(th3(t))*cos(th5(t))^2*sin(th1(t))^2*sin(th3(t))*cos(delta - th4(t))^2*diff(th1(t), t)*diff(th3(t), t))/2 - (l5^2*m5*cos(th1(t))^2*cos(th2(t))^2*cos(th5(t))*sin(th3(t))^2*sin(th5(t))*cos(delta - th4(t))^2*diff(th1(t), t)*diff(th5(t), t))/2 - 2*l3*l4*m5*cos(th1(t))^2*cos(th2(t))*sin(th2(t))*sin(th3(t))^2*cos(delta - th4(t))*diff(th1(t), t)*diff(th2(t), t) - 2*l3*l4*m4*cos(th2(t))^2*cos(th3(t))*sin(th1(t))^2*sin(th3(t))*cos(delta - th4(t))*diff(th1(t), t)*diff(th3(t), t) - 4*l3*l4*m5*cos(th2(t))^2*cos(th3(t))*sin(th1(t))^2*sin(th3(t))*cos(delta - th4(t))*diff(th1(t), t)*diff(th3(t), t) + l3*l4*m4*cos(th1(t))^2*cos(th2(t))^2*cos(th3(t))*sin(th3(t))*sin(delta - th4(t))*diff(th3(t), t)*diff(th4(t), t) + l2*l5*m5*cos(th1(t))^2*cos(th2(t))^2*cos(th5(t))*sin(th3(t))*sin(delta - th4(t))*diff(th1(t), t)*diff(th4(t), t) + l3*l4*m5*cos(th1(t))^2*cos(th2(t))^2*cos(th3(t))*sin(th3(t))*sin(delta - th4(t))*diff(th3(t), t)*diff(th4(t), t) - l2*l5*m5*cos(th1(t))^2*cos(th2(t))^2*sin(th3(t))*sin(th5(t))*cos(delta - th4(t))*diff(th1(t), t)*diff(th5(t), t) - (l5^2*m5*cos(th2(t))*cos(th5(t))^2*sin(th1(t))^2*sin(th2(t))*sin(th3(t))^2*cos(delta - th4(t))^2*diff(th1(t), t)*diff(th2(t), t))/2 - (l5^2*m5*cos(th2(t))^2*cos(th5(t))*sin(th1(t))^2*sin(th3(t))^2*sin(th5(t))*cos(delta - th4(t))^2*diff(th1(t), t)*diff(th5(t), t))/2 + l3*l5*m5*cos(th1(t))*cos(th2(t))^2*cos(th5(t))*sin(th1(t))*sin(th3(t))^2*sin(delta - th4(t))*diff(th4(t), t, t) - l3*l5*m5*cos(th1(t))*cos(th2(t))^2*sin(th1(t))*sin(th3(t))^2*sin(th5(t))*cos(delta - th4(t))*diff(th5(t), t, t) + 2*l3*l4*m4*cos(th2(t))*sin(th1(t))^2*sin(th2(t))*sin(th3(t))^2*cos(delta - th4(t))*diff(th1(t), t)*diff(th2(t), t) - l3*l4*m4*cos(th1(t))*cos(th2(t))^2*sin(th1(t))*sin(th3(t))^2*sin(delta - th4(t))*diff(th1(t), t)*diff(th4(t), t) + 4*l3*l4*m5*cos(th2(t))*sin(th1(t))^2*sin(th2(t))*sin(th3(t))^2*cos(delta - th4(t))*diff(th1(t), t)*diff(th2(t), t) - l3*l4*m5*cos(th1(t))*cos(th2(t))^2*sin(th1(t))*sin(th3(t))^2*sin(delta - th4(t))*diff(th1(t), t)*diff(th4(t), t) - l3*l4*m4*cos(th1(t))^2*cos(th2(t))*sin(th2(t))*sin(th3(t))^2*sin(delta - th4(t))*diff(th2(t), t)*diff(th4(t), t) - l3*l4*m5*cos(th1(t))^2*cos(th2(t))*sin(th2(t))*sin(th3(t))^2*sin(delta - th4(t))*diff(th2(t), t)*diff(th4(t), t) - l2*l5*m5*cos(th2(t))^2*cos(th5(t))*sin(th1(t))^2*sin(th3(t))*sin(delta - th4(t))*diff(th1(t), t)*diff(th4(t), t) + l2*l5*m5*cos(th2(t))^2*sin(th1(t))^2*sin(th3(t))*sin(th5(t))*cos(delta - th4(t))*diff(th1(t), t)*diff(th5(t), t) + (l5^2*m5*cos(th1(t))^2*cos(th2(t))^2*cos(th5(t))^2*sin(th3(t))^2*cos(delta - th4(t))*sin(delta - th4(t))*diff(th1(t), t)*diff(th4(t), t))/2 + (l5^2*m5*cos(th2(t))^2*cos(th5(t))^2*sin(th1(t))^2*sin(th3(t))^2*cos(delta - th4(t))*sin(delta - th4(t))*diff(th1(t), t)*diff(th4(t), t))/2 - l4^2*m5*cos(th1(t))*cos(th2(t))^2*cos(th3(t))*sin(th1(t))*sin(th3(t))*cos(delta - th4(t))^2*diff(th1(t), t)*diff(th3(t), t) - (l4^2*m5*cos(th1(t))^2*cos(th2(t))*cos(th3(t))*sin(th2(t))*sin(th3(t))*cos(delta - th4(t))^2*diff(th2(t), t)*diff(th3(t), t))/2 + (l4*l5*m5*cos(th1(t))*cos(th2(t))^2*cos(th5(t))*sin(th1(t))*sin(th3(t))^2*cos(delta - th4(t))^2*diff(th1(t), t)^2)/2 + (l4*l5*m5*cos(th1(t))*cos(th2(t))^2*cos(th5(t))*sin(th1(t))*sin(th3(t))^2*cos(delta - th4(t))^2*diff(th2(t), t)^2)/2 + (l4*l5*m5*cos(th1(t))*cos(th2(t))^2*cos(th5(t))*sin(th1(t))*sin(th3(t))^2*cos(delta - th4(t))^2*diff(th3(t), t)^2)/2 + (l4*l5*m5*cos(th1(t))*cos(th2(t))^2*cos(th5(t))*sin(th1(t))*sin(th3(t))^2*cos(delta - th4(t))^2*diff(th4(t), t)^2)/2 + (l4*l5*m5*cos(th1(t))*cos(th2(t))^2*cos(th5(t))*sin(th1(t))*sin(th3(t))^2*cos(delta - th4(t))^2*diff(th5(t), t)^2)/4 + (l4*l5*m5*cos(th1(t))^2*cos(th2(t))^2*cos(th3(t))*cos(th5(t))*sin(th3(t))*cos(delta - th4(t))^2*diff(th3(t), t, t))/4 + l4^2*m5*cos(th1(t))*cos(th2(t))*sin(th1(t))*sin(th2(t))*sin(th3(t))^2*cos(delta - th4(t))^2*diff(th1(t), t)*diff(th2(t), t) + (l4^2*m5*cos(th2(t))*cos(th3(t))*sin(th1(t))^2*sin(th2(t))*sin(th3(t))*cos(delta - th4(t))^2*diff(th2(t), t)*diff(th3(t), t))/2 - l2*l4*m4*cos(th1(t))*cos(th2(t))*sin(th1(t))*sin(th2(t))*sin(th3(t))*cos(delta - th4(t))*diff(th2(t), t, t) - 3*l2*l4*m5*cos(th1(t))*cos(th2(t))*sin(th1(t))*sin(th2(t))*sin(th3(t))*cos(delta - th4(t))*diff(th2(t), t, t) - l4^2*m4*cos(th1(t))*cos(th2(t))^2*cos(th3(t))*sin(th1(t))*sin(th3(t))*cos(delta - th4(t))*sin(delta - th4(t))*diff(th3(t), t)*diff(th4(t), t) - 2*l4^2*m5*cos(th1(t))*cos(th2(t))^2*cos(th3(t))*sin(th1(t))*sin(th3(t))*cos(delta - th4(t))*sin(delta - th4(t))*diff(th3(t), t)*diff(th4(t), t) - 2*l3*l5*m5*cos(th1(t))*cos(th2(t))^2*sin(th1(t))*sin(th3(t))^2*sin(th5(t))*sin(delta - th4(t))*diff(th4(t), t)*diff(th5(t), t) + l4^2*m4*cos(th1(t))*cos(th2(t))*sin(th1(t))*sin(th2(t))*sin(th3(t))^2*cos(delta - th4(t))*sin(delta - th4(t))*diff(th2(t), t)*diff(th4(t), t) + 2*l4^2*m5*cos(th1(t))*cos(th2(t))*sin(th1(t))*sin(th2(t))*sin(th3(t))^2*cos(delta - th4(t))*sin(delta - th4(t))*diff(th2(t), t)*diff(th4(t), t) - (l4*l5*m5*cos(th1(t))*cos(th2(t))^2*cos(th5(t))*sin(th1(t))*sin(th3(t))^2*cos(delta - th4(t))*sin(delta - th4(t))*diff(th4(t), t, t))/2 - l2*l4*m4*cos(th1(t))*cos(th2(t))*cos(th3(t))*sin(th1(t))*sin(th2(t))*cos(delta - th4(t))*diff(th2(t), t)*diff(th3(t), t) - 3*l2*l4*m5*cos(th1(t))*cos(th2(t))*cos(th3(t))*sin(th1(t))*sin(th2(t))*cos(delta - th4(t))*diff(th2(t), t)*diff(th3(t), t) + l4*l5*m5*cos(th1(t))^2*cos(th2(t))^2*cos(th3(t))*cos(th5(t))*sin(th3(t))*cos(delta - th4(t))^2*diff(th1(t), t)*diff(th3(t), t) - 2*l2*l5*m5*cos(th1(t))*cos(th2(t))*cos(th5(t))*sin(th1(t))*sin(th2(t))*sin(th3(t))*cos(delta - th4(t))*diff(th2(t), t, t) + 2*l2*l4*m4*cos(th1(t))*cos(th2(t))*sin(th1(t))*sin(th2(t))*sin(th3(t))*cos(delta - th4(t))*diff(th1(t), t)*diff(th2(t), t) + 2*l2*l4*m5*cos(th1(t))*cos(th2(t))*sin(th1(t))*sin(th2(t))*sin(th3(t))*cos(delta - th4(t))*diff(th1(t), t)*diff(th2(t), t) - l4*l5*m5*cos(th1(t))^2*cos(th2(t))*cos(th5(t))*sin(th2(t))*sin(th3(t))^2*cos(delta - th4(t))^2*diff(th1(t), t)*diff(th2(t), t) + 2*l4*l5*m5*cos(th2(t))^2*cos(th3(t))*cos(th5(t))*sin(th1(t))^2*sin(th3(t))*cos(delta - th4(t))^2*diff(th1(t), t)*diff(th3(t), t) - l2*l4*m4*cos(th1(t))*cos(th2(t))*sin(th1(t))*sin(th2(t))*sin(th3(t))*sin(delta - th4(t))*diff(th2(t), t)*diff(th4(t), t) - 3*l2*l4*m5*cos(th1(t))*cos(th2(t))*sin(th1(t))*sin(th2(t))*sin(th3(t))*sin(delta - th4(t))*diff(th2(t), t)*diff(th4(t), t) - 2*l4*l5*m5*cos(th2(t))*cos(th5(t))*sin(th1(t))^2*sin(th2(t))*sin(th3(t))^2*cos(delta - th4(t))^2*diff(th1(t), t)*diff(th2(t), t) + (l4*l5*m5*cos(th1(t))*cos(th2(t))^2*sin(th1(t))*sin(th3(t))^2*sin(th5(t))*cos(delta - th4(t))^2*diff(th1(t), t)*diff(th5(t), t))/2 + (l4*l5*m5*cos(th2(t))^2*cos(th3(t))*sin(th1(t))^2*sin(th3(t))*sin(th5(t))*cos(delta - th4(t))^2*diff(th3(t), t)*diff(th5(t), t))/2 - (l4*l5*m5*cos(th2(t))*sin(th1(t))^2*sin(th2(t))*sin(th3(t))^2*sin(th5(t))*cos(delta - th4(t))^2*diff(th2(t), t)*diff(th5(t), t))/2 + l4*l5*m5*cos(th1(t))^2*cos(th2(t))^2*cos(th5(t))*sin(th3(t))^2*cos(delta - th4(t))*sin(delta - th4(t))*diff(th1(t), t)*diff(th4(t), t) + 2*l4*l5*m5*cos(th2(t))^2*cos(th5(t))*sin(th1(t))^2*sin(th3(t))^2*cos(delta - th4(t))*sin(delta - th4(t))*diff(th1(t), t)*diff(th4(t), t) + 2*l3*l5*m5*cos(th1(t))*cos(th2(t))^2*cos(th3(t))*cos(th5(t))*sin(th1(t))*sin(th3(t))*cos(delta - th4(t))*diff(th3(t), t, t) - 2*l3*l4*m4*cos(th1(t))*cos(th2(t))^2*cos(th3(t))*sin(th1(t))*sin(th3(t))*cos(delta - th4(t))*diff(th1(t), t)*diff(th3(t), t) - 2*l3*l4*m5*cos(th1(t))*cos(th2(t))^2*cos(th3(t))*sin(th1(t))*sin(th3(t))*cos(delta - th4(t))*diff(th1(t), t)*diff(th3(t), t) - l3*l4*m4*cos(th1(t))^2*cos(th2(t))*cos(th3(t))*sin(th2(t))*sin(th3(t))*cos(delta - th4(t))*diff(th2(t), t)*diff(th3(t), t) - 2*l2*l5*m5*cos(th1(t))^2*cos(th2(t))*cos(th5(t))*sin(th2(t))*sin(th3(t))*cos(delta - th4(t))*diff(th1(t), t)*diff(th2(t), t) - l3*l4*m5*cos(th1(t))^2*cos(th2(t))*cos(th3(t))*sin(th2(t))*sin(th3(t))*cos(delta - th4(t))*diff(th2(t), t)*diff(th3(t), t) + 2*l2*l5*m5*cos(th1(t))*cos(th2(t))^2*cos(th3(t))*cos(th5(t))*sin(th1(t))*sin(delta - th4(t))*diff(th3(t), t)*diff(th4(t), t) - 2*l2*l5*m5*cos(th1(t))*cos(th2(t))^2*cos(th3(t))*sin(th1(t))*sin(th5(t))*cos(delta - th4(t))*diff(th3(t), t)*diff(th5(t), t) + (l4*l5*m5*cos(th2(t))^2*sin(th1(t))^2*sin(th3(t))^2*sin(th5(t))*cos(delta - th4(t))*sin(delta - th4(t))*diff(th4(t), t)*diff(th5(t), t))/2 - 2*l3*l5*m5*cos(th1(t))*cos(th2(t))*cos(th5(t))*sin(th1(t))*sin(th2(t))*sin(th3(t))^2*cos(delta - th4(t))*diff(th2(t), t, t) + 2*l3*l4*m4*cos(th1(t))*cos(th2(t))*sin(th1(t))*sin(th2(t))*sin(th3(t))^2*cos(delta - th4(t))*diff(th1(t), t)*diff(th2(t), t) + 2*l3*l4*m5*cos(th1(t))*cos(th2(t))*sin(th1(t))*sin(th2(t))*sin(th3(t))^2*cos(delta - th4(t))*diff(th1(t), t)*diff(th2(t), t) + l3*l4*m4*cos(th2(t))*cos(th3(t))*sin(th1(t))^2*sin(th2(t))*sin(th3(t))*cos(delta - th4(t))*diff(th2(t), t)*diff(th3(t), t) + 2*l2*l5*m5*cos(th2(t))*cos(th5(t))*sin(th1(t))^2*sin(th2(t))*sin(th3(t))*cos(delta - th4(t))*diff(th1(t), t)*diff(th2(t), t) + l3*l4*m4*cos(th1(t))*cos(th2(t))^2*cos(th3(t))*sin(th1(t))*sin(th3(t))*sin(delta - th4(t))*diff(th3(t), t)*diff(th4(t), t) + l3*l4*m5*cos(th2(t))*cos(th3(t))*sin(th1(t))^2*sin(th2(t))*sin(th3(t))*cos(delta - th4(t))*diff(th2(t), t)*diff(th3(t), t) + 3*l3*l4*m5*cos(th1(t))*cos(th2(t))^2*cos(th3(t))*sin(th1(t))*sin(th3(t))*sin(delta - th4(t))*diff(th3(t), t)*diff(th4(t), t) - l3*l4*m4*cos(th1(t))*cos(th2(t))*sin(th1(t))*sin(th2(t))*sin(th3(t))^2*sin(delta - th4(t))*diff(th2(t), t)*diff(th4(t), t) - 3*l3*l4*m5*cos(th1(t))*cos(th2(t))*sin(th1(t))*sin(th2(t))*sin(th3(t))^2*sin(delta - th4(t))*diff(th2(t), t)*diff(th4(t), t) - 2*l2*l5*m5*cos(th1(t))*cos(th2(t))^2*sin(th1(t))*sin(th3(t))*sin(th5(t))*sin(delta - th4(t))*diff(th4(t), t)*diff(th5(t), t) + l4^2*m4*cos(th1(t))*cos(th2(t))*cos(th3(t))*sin(th1(t))*sin(th2(t))*sin(th3(t))*cos(delta - th4(t))^2*diff(th2(t), t)*diff(th3(t), t) + 2*l4^2*m5*cos(th1(t))*cos(th2(t))*cos(th3(t))*sin(th1(t))*sin(th2(t))*sin(th3(t))*cos(delta - th4(t))^2*diff(th2(t), t)*diff(th3(t), t) + 2*l3*l5*m5*cos(th1(t))^2*cos(th2(t))^2*cos(th3(t))*cos(th5(t))*sin(th3(t))*cos(delta - th4(t))*diff(th1(t), t)*diff(th3(t), t) - (l4*l5*m5*cos(th1(t))*cos(th2(t))^2*cos(th3(t))*cos(th5(t))*sin(th1(t))*sin(th3(t))*cos(delta - th4(t))^2*diff(th3(t), t, t))/2 - 2*l3*l5*m5*cos(th1(t))^2*cos(th2(t))*cos(th5(t))*sin(th2(t))*sin(th3(t))^2*cos(delta - th4(t))*diff(th1(t), t)*diff(th2(t), t) - 2*l3*l5*m5*cos(th2(t))^2*cos(th3(t))*cos(th5(t))*sin(th1(t))^2*sin(th3(t))*cos(delta - th4(t))*diff(th1(t), t)*diff(th3(t), t) + (l4*l5*m5*cos(th1(t))*cos(th2(t))*cos(th5(t))*sin(th1(t))*sin(th2(t))*sin(th3(t))^2*cos(delta - th4(t))^2*diff(th2(t), t, t))/2 + 2*l3*l5*m5*cos(th2(t))*cos(th5(t))*sin(th1(t))^2*sin(th2(t))*sin(th3(t))^2*cos(delta - th4(t))*diff(th1(t), t)*diff(th2(t), t) - l4*l5*m5*cos(th1(t))*cos(th2(t))^2*cos(th3(t))*cos(th5(t))*sin(th1(t))*sin(th3(t))*cos(delta - th4(t))^2*diff(th1(t), t)*diff(th3(t), t) - (l4*l5*m5*cos(th1(t))^2*cos(th2(t))*cos(th3(t))*cos(th5(t))*sin(th2(t))*sin(th3(t))*cos(delta - th4(t))^2*diff(th2(t), t)*diff(th3(t), t))/2 + l4*l5*m5*cos(th1(t))*cos(th2(t))*cos(th5(t))*sin(th1(t))*sin(th2(t))*sin(th3(t))^2*cos(delta - th4(t))^2*diff(th1(t), t)*diff(th2(t), t) + (l4*l5*m5*cos(th2(t))*cos(th3(t))*cos(th5(t))*sin(th1(t))^2*sin(th2(t))*sin(th3(t))*cos(delta - th4(t))^2*diff(th2(t), t)*diff(th3(t), t))/2 + (l4*l5*m5*cos(th1(t))*cos(th2(t))^2*cos(th3(t))*sin(th1(t))*sin(th3(t))*sin(th5(t))*cos(delta - th4(t))^2*diff(th3(t), t)*diff(th5(t), t))/2 - (l4*l5*m5*cos(th1(t))*cos(th2(t))*sin(th1(t))*sin(th2(t))*sin(th3(t))^2*sin(th5(t))*cos(delta - th4(t))^2*diff(th2(t), t)*diff(th5(t), t))/2 + (l4*l5*m5*cos(th1(t))^2*cos(th2(t))^2*cos(th3(t))*cos(th5(t))*sin(th3(t))*cos(delta - th4(t))*sin(delta - th4(t))*diff(th3(t), t)*diff(th4(t), t))/2 - l4*l5*m5*cos(th1(t))*cos(th2(t))^2*cos(th5(t))*sin(th1(t))*sin(th3(t))^2*cos(delta - th4(t))*sin(delta - th4(t))*diff(th1(t), t)*diff(th4(t), t) - (l4*l5*m5*cos(th1(t))^2*cos(th2(t))*cos(th5(t))*sin(th2(t))*sin(th3(t))^2*cos(delta - th4(t))*sin(delta - th4(t))*diff(th2(t), t)*diff(th4(t), t))/2 - (l4*l5*m5*cos(th2(t))^2*cos(th3(t))*cos(th5(t))*sin(th1(t))^2*sin(th3(t))*cos(delta - th4(t))*sin(delta - th4(t))*diff(th3(t), t)*diff(th4(t), t))/2 - 2*l2*l5*m5*cos(th1(t))*cos(th2(t))*cos(th3(t))*cos(th5(t))*sin(th1(t))*sin(th2(t))*cos(delta - th4(t))*diff(th2(t), t)*diff(th3(t), t) + (l4*l5*m5*cos(th2(t))*cos(th5(t))*sin(th1(t))^2*sin(th2(t))*sin(th3(t))^2*cos(delta - th4(t))*sin(delta - th4(t))*diff(th2(t), t)*diff(th4(t), t))/2 + (l4*l5*m5*cos(th1(t))*cos(th2(t))^2*sin(th1(t))*sin(th3(t))^2*sin(th5(t))*cos(delta - th4(t))*sin(delta - th4(t))*diff(th4(t), t)*diff(th5(t), t))/2 - 2*l3*l4*m4*cos(th1(t))*cos(th2(t))*cos(th3(t))*sin(th1(t))*sin(th2(t))*sin(th3(t))*cos(delta - th4(t))*diff(th2(t), t)*diff(th3(t), t) - 6*l3*l4*m5*cos(th1(t))*cos(th2(t))*cos(th3(t))*sin(th1(t))*sin(th2(t))*sin(th3(t))*cos(delta - th4(t))*diff(th2(t), t)*diff(th3(t), t) - 2*l2*l5*m5*cos(th1(t))*cos(th2(t))*cos(th5(t))*sin(th1(t))*sin(th2(t))*sin(th3(t))*sin(delta - th4(t))*diff(th2(t), t)*diff(th4(t), t) + 2*l2*l5*m5*cos(th1(t))*cos(th2(t))*sin(th1(t))*sin(th2(t))*sin(th3(t))*sin(th5(t))*cos(delta - th4(t))*diff(th2(t), t)*diff(th5(t), t) + 2*l3*l5*m5*cos(th1(t))*cos(th2(t))^2*cos(th3(t))*cos(th5(t))*sin(th1(t))*sin(th3(t))*sin(delta - th4(t))*diff(th3(t), t)*diff(th4(t), t) - 2*l3*l5*m5*cos(th1(t))*cos(th2(t))^2*cos(th3(t))*sin(th1(t))*sin(th3(t))*sin(th5(t))*cos(delta - th4(t))*diff(th3(t), t)*diff(th5(t), t) - 2*l3*l5*m5*cos(th1(t))*cos(th2(t))*cos(th5(t))*sin(th1(t))*sin(th2(t))*sin(th3(t))^2*sin(delta - th4(t))*diff(th2(t), t)*diff(th4(t), t) + 2*l3*l5*m5*cos(th1(t))*cos(th2(t))*sin(th1(t))*sin(th2(t))*sin(th3(t))^2*sin(th5(t))*cos(delta - th4(t))*diff(th2(t), t)*diff(th5(t), t) + l4*l5*m5*cos(th1(t))*cos(th2(t))*cos(th3(t))*cos(th5(t))*sin(th1(t))*sin(th2(t))*sin(th3(t))*cos(delta - th4(t))^2*diff(th2(t), t)*diff(th3(t), t) - l4*l5*m5*cos(th1(t))*cos(th2(t))^2*cos(th3(t))*cos(th5(t))*sin(th1(t))*sin(th3(t))*cos(delta - th4(t))*sin(delta - th4(t))*diff(th3(t), t)*diff(th4(t), t) + l4*l5*m5*cos(th1(t))*cos(th2(t))*cos(th5(t))*sin(th1(t))*sin(th2(t))*sin(th3(t))^2*cos(delta - th4(t))*sin(delta - th4(t))*diff(th2(t), t)*diff(th4(t), t) - 4*l3*l5*m5*cos(th1(t))*cos(th2(t))*cos(th3(t))*cos(th5(t))*sin(th1(t))*sin(th2(t))*sin(th3(t))*cos(delta - th4(t))*diff(th2(t), t)*diff(th3(t), t);
 

C1 = [ ];

th1dd = (u1 - (m4*(2*(l2*cos(th1)*cos(th2)*th1d - l2*sin(th1)*sin(th2)*th2d + l3*cos(th1)*cos(th2)*sin(th3)*th1d + l3*cos(th2)*cos(th3)*sin(th1)*th3d - l3*sin(th1)*sin(th2)*sin(th3)*th2d + (l4*cos(th1)*cos(th2)*cos(th3)*cos(delta - th4)*th3d)/2 - (l4*cos(th2)*sin(th1)*sin(th3)*cos(delta - th4)*th1d)/2 - (l4*cos(th1)*sin(th2)*sin(th3)*cos(delta - th4)*th2d)/2 + (l4*cos(th1)*cos(th2)*sin(th3)*sin(delta - th4)*th4d)/2)*(l2*cos(th2)*sin(th1)*th1d + l2*cos(th1)*sin(th2)*th2d - l3*cos(th1)*cos(th2)*cos(th3)*th3d + l3*cos(th2)*sin(th1)*sin(th3)*th1d + l3*cos(th1)*sin(th2)*sin(th3)*th2d - (l4*sin(th1)*sin(th2)*sin(th3)*cos(delta - th4)*th2d)/2 + (l4*cos(th2)*sin(th1)*sin(th3)*sin(delta - th4)*th4d)/2 + (l4*cos(th1)*cos(th2)*sin(th3)*cos(delta - th4)*th1d)/2 + (l4*cos(th2)*cos(th3)*sin(th1)*cos(delta - th4)*th3d)/2) + 2*(l2*cos(th2)*sin(th1)*th1d + l2*cos(th1)*sin(th2)*th2d - l3*cos(th1)*cos(th2)*cos(th3)*th3d + l3*cos(th2)*sin(th1)*sin(th3)*th1d + l3*cos(th1)*sin(th2)*sin(th3)*th2d + (l4*cos(th1)*cos(th2)*cos(th3)*cos(delta - th4)*th3d)/2 - (l4*cos(th2)*sin(th1)*sin(th3)*cos(delta - th4)*th1d)/2 - (l4*cos(th1)*sin(th2)*sin(th3)*cos(delta - th4)*th2d)/2 + (l4*cos(th1)*cos(th2)*sin(th3)*sin(delta - th4)*th4d)/2)*(- l2*cos(th1)*cos(th2)*th1d + l2*sin(th1)*sin(th2)*th2d - l3*cos(th1)*cos(th2)*sin(th3)*th1d - l3*cos(th2)*cos(th3)*sin(th1)*th3d + l3*sin(th1)*sin(th2)*sin(th3)*th2d - (l4*sin(th1)*sin(th2)*sin(th3)*cos(delta - th4)*th2d)/2 + (l4*cos(th2)*sin(th1)*sin(th3)*sin(delta - th4)*th4d)/2 + (l4*cos(th1)*cos(th2)*sin(th3)*cos(delta - th4)*th1d)/2 + (l4*cos(th2)*cos(th3)*sin(th1)*cos(delta - th4)*th3d)/2)))/2 + (m2*(l2*cos(th1)*cos(th2)*((l2*cos(th2)*sin(th1)*th1d^2)/2 + (l2*cos(th2)*sin(th1)*th2d^2)/2 + (l2*sin(th1)*sin(th2)*th2dd)/2 + l2*cos(th1)*sin(th2)*th2d*th1d) - l2*cos(th2)*sin(th1)*((l2*cos(th1)*cos(th2)*th1d^2)/2 + (l2*cos(th1)*cos(th2)*th2d^2)/2 + (l2*cos(th1)*sin(th2)*th2dd)/2 - l2*sin(th1)*sin(th2)*th2d*th1d) + l2*sin(th1)*sin(th2)*((l2*cos(th2)*sin(th1)*th1d)/2 + (l2*cos(th1)*sin(th2)*th2d)/2)*th2d - l2*cos(th1)*cos(th2)*((l2*cos(th2)*sin(th1)*th1d)/2 + (l2*cos(th1)*sin(th2)*th2d)/2)*th1d + l2*cos(th2)*sin(th1)*((l2*cos(th1)*cos(th2)*th1d)/2 - (l2*sin(th1)*sin(th2)*th2d)/2)*th1d + l2*cos(th1)*sin(th2)*((l2*cos(th1)*cos(th2)*th1d)/2 - (l2*sin(th1)*sin(th2)*th2d)/2)*th2d))/2 + (m5*(2*(l2*cos(th1)*cos(th2) + l3*cos(th1)*cos(th2)*sin(th3) + (l4*cos(th1)*cos(th2)*sin(th3)*cos(delta - th4))/2 - (l4*cos(th2)*sin(th1)*sin(th3)*cos(delta - th4))/2 + (l5*cos(th1)*cos(th2)*cos(th5)*sin(th3)*cos(delta - th4))/2)*(l2*cos(th2)*sin(th1)*th1d^2 + l2*cos(th2)*sin(th1)*th2d^2 + l2*sin(th1)*sin(th2)*th2dd + l3*sin(th1)*sin(th2)*sin(th3)*th2dd + l3*cos(th2)*sin(th1)*sin(th3)*th1d^2 + l3*cos(th2)*sin(th1)*sin(th3)*th2d^2 + l3*cos(th2)*sin(th1)*sin(th3)*th3d^2 - l3*cos(th2)*cos(th3)*sin(th1)*th3dd + 2*l2*cos(th1)*sin(th2)*th2d*th1d - 2*l3*cos(th1)*cos(th2)*cos(th3)*th3d*th1d + (l4*cos(th1)*cos(th2)*sin(th3)*cos(delta - th4)*th1d^2)/2 + (l4*cos(th1)*cos(th2)*sin(th3)*cos(delta - th4)*th2d^2)/2 + (l4*cos(th1)*cos(th2)*sin(th3)*cos(delta - th4)*th3d^2)/2 + (l4*cos(th1)*cos(th2)*sin(th3)*cos(delta - th4)*th4d^2)/2 + 2*l3*cos(th1)*sin(th2)*sin(th3)*th2d*th1d + 2*l3*cos(th3)*sin(th1)*sin(th2)*th3d*th2d - (l4*cos(th1)*cos(th2)*cos(th3)*cos(delta - th4)*th3dd)/2 + (l4*cos(th2)*sin(th1)*sin(th3)*cos(delta - th4)*th1d^2)/2 + (l4*cos(th2)*sin(th1)*sin(th3)*cos(delta - th4)*th2d^2)/2 + (l4*cos(th2)*sin(th1)*sin(th3)*cos(delta - th4)*th3d^2)/2 + (l4*cos(th2)*sin(th1)*sin(th3)*cos(delta - th4)*th4d^2)/2 - (l4*cos(th2)*cos(th3)*sin(th1)*cos(delta - th4)*th3dd)/2 + (l4*cos(th1)*sin(th2)*sin(th3)*cos(delta - th4)*th2dd)/2 - (l4*cos(th1)*cos(th2)*sin(th3)*sin(delta - th4)*th4dd)/2 + (l4*sin(th1)*sin(th2)*sin(th3)*cos(delta - th4)*th2dd)/2 - (l4*cos(th2)*sin(th1)*sin(th3)*sin(delta - th4)*th4dd)/2 - l4*cos(th1)*cos(th2)*cos(th3)*cos(delta - th4)*th3d*th1d + (l5*cos(th2)*cos(th5)*sin(th1)*sin(th3)*cos(delta - th4)*th1d^2)/2 + (l5*cos(th2)*cos(th5)*sin(th1)*sin(th3)*cos(delta - th4)*th2d^2)/2 + (l5*cos(th2)*cos(th5)*sin(th1)*sin(th3)*cos(delta - th4)*th3d^2)/2 + (l5*cos(th2)*cos(th5)*sin(th1)*sin(th3)*cos(delta - th4)*th4d^2)/2 + (l5*cos(th2)*cos(th5)*sin(th1)*sin(th3)*cos(delta - th4)*th5d^2)/2 - (l5*cos(th2)*cos(th3)*cos(th5)*sin(th1)*cos(delta - th4)*th3dd)/2 + l4*cos(th2)*cos(th3)*sin(th1)*cos(delta - th4)*th3d*th1d + l4*cos(th1)*cos(th3)*sin(th2)*cos(delta - th4)*th3d*th2d - l4*cos(th1)*cos(th2)*cos(th3)*sin(delta - th4)*th4d*th3d + l4*cos(th1)*sin(th2)*sin(th3)*cos(delta - th4)*th2d*th1d - l4*cos(th1)*cos(th2)*sin(th3)*sin(delta - th4)*th4d*th1d + l4*cos(th3)*sin(th1)*sin(th2)*cos(delta - th4)*th3d*th2d - l4*cos(th2)*cos(th3)*sin(th1)*sin(delta - th4)*th4d*th3d + (l5*cos(th5)*sin(th1)*sin(th2)*sin(th3)*cos(delta - th4)*th2dd)/2 - (l5*cos(th2)*cos(th5)*sin(th1)*sin(th3)*sin(delta - th4)*th4dd)/2 + (l5*cos(th2)*sin(th1)*sin(th3)*sin(th5)*cos(delta - th4)*th5dd)/2 - l4*sin(th1)*sin(th2)*sin(th3)*cos(delta - th4)*th2d*th1d + l4*cos(th2)*sin(th1)*sin(th3)*sin(delta - th4)*th4d*th1d + l4*cos(th1)*sin(th2)*sin(th3)*sin(delta - th4)*th4d*th2d + l4*sin(th1)*sin(th2)*sin(th3)*sin(delta - th4)*th4d*th2d + l5*cos(th1)*cos(th5)*sin(th2)*sin(th3)*cos(delta - th4)*th2d*th1d - l5*cos(th1)*cos(th2)*cos(th5)*sin(th3)*sin(delta - th4)*th4d*th1d + l5*cos(th3)*cos(th5)*sin(th1)*sin(th2)*cos(delta - th4)*th3d*th2d + l5*cos(th1)*cos(th2)*sin(th3)*sin(th5)*cos(delta - th4)*th5d*th1d - l5*cos(th2)*cos(th3)*cos(th5)*sin(th1)*sin(delta - th4)*th4d*th3d + l5*cos(th2)*cos(th3)*sin(th1)*sin(th5)*cos(delta - th4)*th5d*th3d + l5*cos(th5)*sin(th1)*sin(th2)*sin(th3)*sin(delta - th4)*th4d*th2d - l5*sin(th1)*sin(th2)*sin(th3)*sin(th5)*cos(delta - th4)*th5d*th2d + l5*cos(th2)*sin(th1)*sin(th3)*sin(th5)*sin(delta - th4)*th5d*th4d - l5*cos(th1)*cos(th2)*cos(th3)*cos(th5)*cos(delta - th4)*th3d*th1d) + 2*(l2*cos(th2)*sin(th1) + l3*cos(th2)*sin(th1)*sin(th3) - l4*cos(th2)*sin(th1)*sin(th3)*cos(delta - th4) - (l5*cos(th2)*cos(th5)*sin(th1)*sin(th3)*cos(delta - th4))/2)*(2*l2*sin(th1)*sin(th2)*th2d*th1d - l2*cos(th1)*cos(th2)*th2d^2 - l2*cos(th1)*sin(th2)*th2dd - l3*cos(th1)*sin(th2)*sin(th3)*th2dd - l2*cos(th1)*cos(th2)*th1d^2 - l3*cos(th1)*cos(th2)*sin(th3)*th1d^2 - l3*cos(th1)*cos(th2)*sin(th3)*th2d^2 - l3*cos(th1)*cos(th2)*sin(th3)*th3d^2 + l3*cos(th1)*cos(th2)*cos(th3)*th3dd - 2*l3*cos(th2)*cos(th3)*sin(th1)*th3d*th1d - 2*l3*cos(th1)*cos(th3)*sin(th2)*th3d*th2d + l4*cos(th1)*cos(th2)*sin(th3)*cos(delta - th4)*th1d^2 + l4*cos(th1)*cos(th2)*sin(th3)*cos(delta - th4)*th2d^2 + l4*cos(th1)*cos(th2)*sin(th3)*cos(delta - th4)*th3d^2 + l4*cos(th1)*cos(th2)*sin(th3)*cos(delta - th4)*th4d^2 - l4*cos(th1)*cos(th2)*cos(th3)*cos(delta - th4)*th3dd + 2*l3*sin(th1)*sin(th2)*sin(th3)*th2d*th1d + l4*cos(th1)*sin(th2)*sin(th3)*cos(delta - th4)*th2dd - l4*cos(th1)*cos(th2)*sin(th3)*sin(delta - th4)*th4dd + (l5*cos(th1)*cos(th2)*cos(th5)*sin(th3)*cos(delta - th4)*th1d^2)/2 + (l5*cos(th1)*cos(th2)*cos(th5)*sin(th3)*cos(delta - th4)*th2d^2)/2 + (l5*cos(th1)*cos(th2)*cos(th5)*sin(th3)*cos(delta - th4)*th3d^2)/2 + (l5*cos(th1)*cos(th2)*cos(th5)*sin(th3)*cos(delta - th4)*th4d^2)/2 + (l5*cos(th1)*cos(th2)*cos(th5)*sin(th3)*cos(delta - th4)*th5d^2)/2 - (l5*cos(th1)*cos(th2)*cos(th3)*cos(th5)*cos(delta - th4)*th3dd)/2 + 2*l4*cos(th2)*cos(th3)*sin(th1)*cos(delta - th4)*th3d*th1d + 2*l4*cos(th1)*cos(th3)*sin(th2)*cos(delta - th4)*th3d*th2d - 2*l4*cos(th1)*cos(th2)*cos(th3)*sin(delta - th4)*th4d*th3d + (l5*cos(th1)*cos(th5)*sin(th2)*sin(th3)*cos(delta - th4)*th2dd)/2 - (l5*cos(th1)*cos(th2)*cos(th5)*sin(th3)*sin(delta - th4)*th4dd)/2 + (l5*cos(th1)*cos(th2)*sin(th3)*sin(th5)*cos(delta - th4)*th5dd)/2 - 2*l4*sin(th1)*sin(th2)*sin(th3)*cos(delta - th4)*th2d*th1d + 2*l4*cos(th2)*sin(th1)*sin(th3)*sin(delta - th4)*th4d*th1d + 2*l4*cos(th1)*sin(th2)*sin(th3)*sin(delta - th4)*th4d*th2d - l5*cos(th5)*sin(th1)*sin(th2)*sin(th3)*cos(delta - th4)*th2d*th1d + l5*cos(th2)*cos(th5)*sin(th1)*sin(th3)*sin(delta - th4)*th4d*th1d + l5*cos(th1)*cos(th5)*sin(th2)*sin(th3)*sin(delta - th4)*th4d*th2d - l5*cos(th2)*sin(th1)*sin(th3)*sin(th5)*cos(delta - th4)*th5d*th1d - l5*cos(th1)*sin(th2)*sin(th3)*sin(th5)*cos(delta - th4)*th5d*th2d + l5*cos(th1)*cos(th2)*sin(th3)*sin(th5)*sin(delta - th4)*th5d*th4d + l5*cos(th2)*cos(th3)*cos(th5)*sin(th1)*cos(delta - th4)*th3d*th1d + l5*cos(th1)*cos(th3)*cos(th5)*sin(th2)*cos(delta - th4)*th3d*th2d - l5*cos(th1)*cos(th2)*cos(th3)*cos(th5)*sin(delta - th4)*th4d*th3d + l5*cos(th1)*cos(th2)*cos(th3)*sin(th5)*cos(delta - th4)*th5d*th3d) + 2*(l2*cos(th2)*sin(th1)*th1d + l2*cos(th1)*sin(th2)*th2d - l3*cos(th1)*cos(th2)*cos(th3)*th3d + l3*cos(th2)*sin(th1)*sin(th3)*th1d + l3*cos(th1)*sin(th2)*sin(th3)*th2d - (l4*sin(th1)*sin(th2)*sin(th3)*cos(delta - th4)*th2d)/2 + (l4*cos(th2)*sin(th1)*sin(th3)*sin(delta - th4)*th4d)/2 - (l4*cos(th1)*cos(th2)*cos(th3)*cos(delta - th4)*th3d)/2 + (l4*cos(th1)*cos(th2)*sin(th3)*cos(delta - th4)*th1d)/2 + (l4*cos(th2)*cos(th3)*sin(th1)*cos(delta - th4)*th3d)/2 + (l4*cos(th2)*sin(th1)*sin(th3)*cos(delta - th4)*th1d)/2 + (l4*cos(th1)*sin(th2)*sin(th3)*cos(delta - th4)*th2d)/2 - (l4*cos(th1)*cos(th2)*sin(th3)*sin(delta - th4)*th4d)/2 - (l5*cos(th1)*cos(th2)*cos(th3)*cos(th5)*cos(delta - th4)*th3d)/2 + (l5*cos(th2)*cos(th5)*sin(th1)*sin(th3)*cos(delta - th4)*th1d)/2 + (l5*cos(th1)*cos(th5)*sin(th2)*sin(th3)*cos(delta - th4)*th2d)/2 - (l5*cos(th1)*cos(th2)*cos(th5)*sin(th3)*sin(delta - th4)*th4d)/2 + (l5*cos(th1)*cos(th2)*sin(th3)*sin(th5)*cos(delta - th4)*th5d)/2)*(l2*cos(th1)*cos(th2)*th1d - l2*sin(th1)*sin(th2)*th2d + l3*cos(th1)*cos(th2)*sin(th3)*th1d + l3*cos(th2)*cos(th3)*sin(th1)*th3d - l3*sin(th1)*sin(th2)*sin(th3)*th2d - (l4*sin(th1)*sin(th2)*sin(th3)*cos(delta - th4)*th2d)/2 + (l4*cos(th2)*sin(th1)*sin(th3)*sin(delta - th4)*th4d)/2 + (l4*cos(th1)*cos(th2)*cos(th3)*cos(delta - th4)*th3d)/2 + (l4*cos(th1)*cos(th2)*sin(th3)*cos(delta - th4)*th1d)/2 + (l4*cos(th2)*cos(th3)*sin(th1)*cos(delta - th4)*th3d)/2 - (l4*cos(th2)*sin(th1)*sin(th3)*cos(delta - th4)*th1d)/2 - (l4*cos(th1)*sin(th2)*sin(th3)*cos(delta - th4)*th2d)/2 + (l4*cos(th1)*cos(th2)*sin(th3)*sin(delta - th4)*th4d)/2 + (l5*cos(th1)*cos(th2)*cos(th5)*sin(th3)*cos(delta - th4)*th1d)/2 + (l5*cos(th2)*cos(th3)*cos(th5)*sin(th1)*cos(delta - th4)*th3d)/2 - (l5*cos(th5)*sin(th1)*sin(th2)*sin(th3)*cos(delta - th4)*th2d)/2 + (l5*cos(th2)*cos(th5)*sin(th1)*sin(th3)*sin(delta - th4)*th4d)/2 - (l5*cos(th2)*sin(th1)*sin(th3)*sin(th5)*cos(delta - th4)*th5d)/2) + 2*(l2*cos(th2)*sin(th1)*th1d + l2*cos(th1)*sin(th2)*th2d - l3*cos(th1)*cos(th2)*cos(th3)*th3d + l3*cos(th2)*sin(th1)*sin(th3)*th1d + l3*cos(th1)*sin(th2)*sin(th3)*th2d + l4*cos(th1)*cos(th2)*cos(th3)*cos(delta - th4)*th3d - l4*cos(th2)*sin(th1)*sin(th3)*cos(delta - th4)*th1d - l4*cos(th1)*sin(th2)*sin(th3)*cos(delta - th4)*th2d + l4*cos(th1)*cos(th2)*sin(th3)*sin(delta - th4)*th4d + (l5*cos(th1)*cos(th2)*cos(th3)*cos(th5)*cos(delta - th4)*th3d)/2 - (l5*cos(th2)*cos(th5)*sin(th1)*sin(th3)*cos(delta - th4)*th1d)/2 - (l5*cos(th1)*cos(th5)*sin(th2)*sin(th3)*cos(delta - th4)*th2d)/2 + (l5*cos(th1)*cos(th2)*cos(th5)*sin(th3)*sin(delta - th4)*th4d)/2 - (l5*cos(th1)*cos(th2)*sin(th3)*sin(th5)*cos(delta - th4)*th5d)/2)*(l2*sin(th1)*sin(th2)*th2d - l2*cos(th1)*cos(th2)*th1d - l3*cos(th1)*cos(th2)*sin(th3)*th1d - l3*cos(th2)*cos(th3)*sin(th1)*th3d + l3*sin(th1)*sin(th2)*sin(th3)*th2d - l4*sin(th1)*sin(th2)*sin(th3)*cos(delta - th4)*th2d + l4*cos(th2)*sin(th1)*sin(th3)*sin(delta - th4)*th4d + l4*cos(th1)*cos(th2)*sin(th3)*cos(delta - th4)*th1d + l4*cos(th2)*cos(th3)*sin(th1)*cos(delta - th4)*th3d + (l5*cos(th1)*cos(th2)*cos(th5)*sin(th3)*cos(delta - th4)*th1d)/2 + (l5*cos(th2)*cos(th3)*cos(th5)*sin(th1)*cos(delta - th4)*th3d)/2 - (l5*cos(th5)*sin(th1)*sin(th2)*sin(th3)*cos(delta - th4)*th2d)/2 + (l5*cos(th2)*cos(th5)*sin(th1)*sin(th3)*sin(delta - th4)*th4d)/2 - (l5*cos(th2)*sin(th1)*sin(th3)*sin(th5)*cos(delta - th4)*th5d)/2)))/2 - (m3*(2*(l2*cos(th2)*sin(th1) + (l3*cos(th2)*sin(th1)*sin(th3))/2)*(l2*cos(th1)*cos(th2)*th1d^2 + l2*cos(th1)*cos(th2)*th2d^2 + l2*cos(th1)*sin(th2)*th2dd + (l3*cos(th1)*sin(th2)*sin(th3)*th2dd)/2 - 2*l2*sin(th1)*sin(th2)*th2d*th1d + (l3*cos(th1)*cos(th2)*sin(th3)*th1d^2)/2 + (l3*cos(th1)*cos(th2)*sin(th3)*th2d^2)/2 + (l3*cos(th1)*cos(th2)*sin(th3)*th3d^2)/2 - (l3*cos(th1)*cos(th2)*cos(th3)*th3dd)/2 + l3*cos(th2)*cos(th3)*sin(th1)*th3d*th1d + l3*cos(th1)*cos(th3)*sin(th2)*th3d*th2d - l3*sin(th1)*sin(th2)*sin(th3)*th2d*th1d) - 2*(l2*cos(th1)*cos(th2) + (l3*cos(th1)*cos(th2)*sin(th3))/2)*(l2*cos(th2)*sin(th1)*th1d^2 + l2*cos(th2)*sin(th1)*th2d^2 + l2*sin(th1)*sin(th2)*th2dd + (l3*sin(th1)*sin(th2)*sin(th3)*th2dd)/2 + (l3*cos(th2)*sin(th1)*sin(th3)*th1d^2)/2 + (l3*cos(th2)*sin(th1)*sin(th3)*th2d^2)/2 + (l3*cos(th2)*sin(th1)*sin(th3)*th3d^2)/2 - (l3*cos(th2)*cos(th3)*sin(th1)*th3dd)/2 + 2*l2*cos(th1)*sin(th2)*th2d*th1d - l3*cos(th1)*cos(th2)*cos(th3)*th3d*th1d + l3*cos(th1)*sin(th2)*sin(th3)*th2d*th1d + l3*cos(th3)*sin(th1)*sin(th2)*th3d*th2d)))/2 - beta1*th1d - (m5*(2*(l2*cos(th2)*sin(th1)*th1d + l2*cos(th1)*sin(th2)*th2d - l3*cos(th1)*cos(th2)*cos(th3)*th3d + l3*cos(th2)*sin(th1)*sin(th3)*th1d + l3*cos(th1)*sin(th2)*sin(th3)*th2d - (l4*sin(th1)*sin(th2)*sin(th3)*cos(delta - th4)*th2d)/2 + (l4*cos(th2)*sin(th1)*sin(th3)*sin(delta - th4)*th4d)/2 - (l4*cos(th1)*cos(th2)*cos(th3)*cos(delta - th4)*th3d)/2 + (l4*cos(th1)*cos(th2)*sin(th3)*cos(delta - th4)*th1d)/2 + (l4*cos(th2)*cos(th3)*sin(th1)*cos(delta - th4)*th3d)/2 + (l4*cos(th2)*sin(th1)*sin(th3)*cos(delta - th4)*th1d)/2 + (l4*cos(th1)*sin(th2)*sin(th3)*cos(delta - th4)*th2d)/2 - (l4*cos(th1)*cos(th2)*sin(th3)*sin(delta - th4)*th4d)/2 - (l5*cos(th1)*cos(th2)*cos(th3)*cos(th5)*cos(delta - th4)*th3d)/2 + (l5*cos(th2)*cos(th5)*sin(th1)*sin(th3)*cos(delta - th4)*th1d)/2 + (l5*cos(th1)*cos(th5)*sin(th2)*sin(th3)*cos(delta - th4)*th2d)/2 - (l5*cos(th1)*cos(th2)*cos(th5)*sin(th3)*sin(delta - th4)*th4d)/2 + (l5*cos(th1)*cos(th2)*sin(th3)*sin(th5)*cos(delta - th4)*th5d)/2)*(l2*cos(th1)*cos(th2)*th1d - l2*sin(th1)*sin(th2)*th2d + l3*cos(th1)*cos(th2)*sin(th3)*th1d + l3*cos(th2)*cos(th3)*sin(th1)*th3d - l3*sin(th1)*sin(th2)*sin(th3)*th2d - (l4*sin(th1)*sin(th2)*sin(th3)*cos(delta - th4)*th2d)/2 + (l4*cos(th2)*sin(th1)*sin(th3)*sin(delta - th4)*th4d)/2 + (l4*cos(th1)*cos(th2)*cos(th3)*cos(delta - th4)*th3d)/2 + (l4*cos(th1)*cos(th2)*sin(th3)*cos(delta - th4)*th1d)/2 + (l4*cos(th2)*cos(th3)*sin(th1)*cos(delta - th4)*th3d)/2 - (l4*cos(th2)*sin(th1)*sin(th3)*cos(delta - th4)*th1d)/2 - (l4*cos(th1)*sin(th2)*sin(th3)*cos(delta - th4)*th2d)/2 + (l4*cos(th1)*cos(th2)*sin(th3)*sin(delta - th4)*th4d)/2 + (l5*cos(th1)*cos(th2)*cos(th5)*sin(th3)*cos(delta - th4)*th1d)/2 + (l5*cos(th2)*cos(th3)*cos(th5)*sin(th1)*cos(delta - th4)*th3d)/2 - (l5*cos(th5)*sin(th1)*sin(th2)*sin(th3)*cos(delta - th4)*th2d)/2 + (l5*cos(th2)*cos(th5)*sin(th1)*sin(th3)*sin(delta - th4)*th4d)/2 - (l5*cos(th2)*sin(th1)*sin(th3)*sin(th5)*cos(delta - th4)*th5d)/2) + 2*(l2*cos(th2)*sin(th1)*th1d + l2*cos(th1)*sin(th2)*th2d - l3*cos(th1)*cos(th2)*cos(th3)*th3d + l3*cos(th2)*sin(th1)*sin(th3)*th1d + l3*cos(th1)*sin(th2)*sin(th3)*th2d + l4*cos(th1)*cos(th2)*cos(th3)*cos(delta - th4)*th3d - l4*cos(th2)*sin(th1)*sin(th3)*cos(delta - th4)*th1d - l4*cos(th1)*sin(th2)*sin(th3)*cos(delta - th4)*th2d + l4*cos(th1)*cos(th2)*sin(th3)*sin(delta - th4)*th4d + (l5*cos(th1)*cos(th2)*cos(th3)*cos(th5)*cos(delta - th4)*th3d)/2 - (l5*cos(th2)*cos(th5)*sin(th1)*sin(th3)*cos(delta - th4)*th1d)/2 - (l5*cos(th1)*cos(th5)*sin(th2)*sin(th3)*cos(delta - th4)*th2d)/2 + (l5*cos(th1)*cos(th2)*cos(th5)*sin(th3)*sin(delta - th4)*th4d)/2 - (l5*cos(th1)*cos(th2)*sin(th3)*sin(th5)*cos(delta - th4)*th5d)/2)*(- l2*cos(th1)*cos(th2)*th1d + l2*sin(th1)*sin(th2)*th2d - l3*cos(th1)*cos(th2)*sin(th3)*th1d - l3*cos(th2)*cos(th3)*sin(th1)*th3d + l3*sin(th1)*sin(th2)*sin(th3)*th2d - l4*sin(th1)*sin(th2)*sin(th3)*cos(delta - th4)*th2d + l4*cos(th2)*sin(th1)*sin(th3)*sin(delta - th4)*th4d + l4*cos(th1)*cos(th2)*sin(th3)*cos(delta - th4)*th1d + l4*cos(th2)*cos(th3)*sin(th1)*cos(delta - th4)*th3d + (l5*cos(th1)*cos(th2)*cos(th5)*sin(th3)*cos(delta - th4)*th1d)/2 + (l5*cos(th2)*cos(th3)*cos(th5)*sin(th1)*cos(delta - th4)*th3d)/2 - (l5*cos(th5)*sin(th1)*sin(th2)*sin(th3)*cos(delta - th4)*th2d)/2 + (l5*cos(th2)*cos(th5)*sin(th1)*sin(th3)*sin(delta - th4)*th4d)/2 - (l5*cos(th2)*sin(th1)*sin(th3)*sin(th5)*cos(delta - th4)*th5d)/2)))/2 + (m4*(2*(l2*cos(th1)*cos(th2) + l3*cos(th1)*cos(th2)*sin(th3) - (l4*cos(th2)*sin(th1)*sin(th3)*cos(delta - th4))/2)*(l2*cos(th2)*sin(th1)*th1d^2 + l2*cos(th2)*sin(th1)*th2d^2 + l2*sin(th1)*sin(th2)*th2dd + l3*sin(th1)*sin(th2)*sin(th3)*th2dd + l3*cos(th2)*sin(th1)*sin(th3)*th1d^2 + l3*cos(th2)*sin(th1)*sin(th3)*th2d^2 + l3*cos(th2)*sin(th1)*sin(th3)*th3d^2 - l3*cos(th2)*cos(th3)*sin(th1)*th3dd + 2*l2*cos(th1)*sin(th2)*th2d*th1d - 2*l3*cos(th1)*cos(th2)*cos(th3)*th3d*th1d + (l4*cos(th1)*cos(th2)*sin(th3)*cos(delta - th4)*th1d^2)/2 + (l4*cos(th1)*cos(th2)*sin(th3)*cos(delta - th4)*th2d^2)/2 + (l4*cos(th1)*cos(th2)*sin(th3)*cos(delta - th4)*th3d^2)/2 + (l4*cos(th1)*cos(th2)*sin(th3)*cos(delta - th4)*th4d^2)/2 + 2*l3*cos(th1)*sin(th2)*sin(th3)*th2d*th1d + 2*l3*cos(th3)*sin(th1)*sin(th2)*th3d*th2d - (l4*cos(th1)*cos(th2)*cos(th3)*cos(delta - th4)*th3dd)/2 + (l4*cos(th1)*sin(th2)*sin(th3)*cos(delta - th4)*th2dd)/2 - (l4*cos(th1)*cos(th2)*sin(th3)*sin(delta - th4)*th4dd)/2 + l4*cos(th2)*cos(th3)*sin(th1)*cos(delta - th4)*th3d*th1d + l4*cos(th1)*cos(th3)*sin(th2)*cos(delta - th4)*th3d*th2d - l4*cos(th1)*cos(th2)*cos(th3)*sin(delta - th4)*th4d*th3d - l4*sin(th1)*sin(th2)*sin(th3)*cos(delta - th4)*th2d*th1d + l4*cos(th2)*sin(th1)*sin(th3)*sin(delta - th4)*th4d*th1d + l4*cos(th1)*sin(th2)*sin(th3)*sin(delta - th4)*th4d*th2d) - 2*(l2*cos(th2)*sin(th1) + l3*cos(th2)*sin(th1)*sin(th3) - (l4*cos(th2)*sin(th1)*sin(th3)*cos(delta - th4))/2)*(l2*cos(th1)*cos(th2)*th1d^2 + l2*cos(th1)*cos(th2)*th2d^2 + l2*cos(th1)*sin(th2)*th2dd + l3*cos(th1)*sin(th2)*sin(th3)*th2dd - 2*l2*sin(th1)*sin(th2)*th2d*th1d + l3*cos(th1)*cos(th2)*sin(th3)*th1d^2 + l3*cos(th1)*cos(th2)*sin(th3)*th2d^2 + l3*cos(th1)*cos(th2)*sin(th3)*th3d^2 - l3*cos(th1)*cos(th2)*cos(th3)*th3dd + 2*l3*cos(th2)*cos(th3)*sin(th1)*th3d*th1d + 2*l3*cos(th1)*cos(th3)*sin(th2)*th3d*th2d - (l4*cos(th1)*cos(th2)*sin(th3)*cos(delta - th4)*th1d^2)/2 - (l4*cos(th1)*cos(th2)*sin(th3)*cos(delta - th4)*th2d^2)/2 - (l4*cos(th1)*cos(th2)*sin(th3)*cos(delta - th4)*th3d^2)/2 - (l4*cos(th1)*cos(th2)*sin(th3)*cos(delta - th4)*th4d^2)/2 + (l4*cos(th1)*cos(th2)*cos(th3)*cos(delta - th4)*th3dd)/2 - 2*l3*sin(th1)*sin(th2)*sin(th3)*th2d*th1d - (l4*cos(th1)*sin(th2)*sin(th3)*cos(delta - th4)*th2dd)/2 + (l4*cos(th1)*cos(th2)*sin(th3)*sin(delta - th4)*th4dd)/2 - l4*cos(th2)*cos(th3)*sin(th1)*cos(delta - th4)*th3d*th1d - l4*cos(th1)*cos(th3)*sin(th2)*cos(delta - th4)*th3d*th2d + l4*cos(th1)*cos(th2)*cos(th3)*sin(delta - th4)*th4d*th3d + l4*sin(th1)*sin(th2)*sin(th3)*cos(delta - th4)*th2d*th1d - l4*cos(th2)*sin(th1)*sin(th3)*sin(delta - th4)*th4d*th1d - l4*cos(th1)*sin(th2)*sin(th3)*sin(delta - th4)*th4d*th2d) + 2*(l2*cos(th1)*cos(th2)*th1d - l2*sin(th1)*sin(th2)*th2d + l3*cos(th1)*cos(th2)*sin(th3)*th1d + l3*cos(th2)*cos(th3)*sin(th1)*th3d - l3*sin(th1)*sin(th2)*sin(th3)*th2d + (l4*cos(th1)*cos(th2)*cos(th3)*cos(delta - th4)*th3d)/2 - (l4*cos(th2)*sin(th1)*sin(th3)*cos(delta - th4)*th1d)/2 - (l4*cos(th1)*sin(th2)*sin(th3)*cos(delta - th4)*th2d)/2 + (l4*cos(th1)*cos(th2)*sin(th3)*sin(delta - th4)*th4d)/2)*(l2*cos(th2)*sin(th1)*th1d + l2*cos(th1)*sin(th2)*th2d - l3*cos(th1)*cos(th2)*cos(th3)*th3d + l3*cos(th2)*sin(th1)*sin(th3)*th1d + l3*cos(th1)*sin(th2)*sin(th3)*th2d - (l4*sin(th1)*sin(th2)*sin(th3)*cos(delta - th4)*th2d)/2 + (l4*cos(th2)*sin(th1)*sin(th3)*sin(delta - th4)*th4d)/2 + (l4*cos(th1)*cos(th2)*sin(th3)*cos(delta - th4)*th1d)/2 + (l4*cos(th2)*cos(th3)*sin(th1)*cos(delta - th4)*th3d)/2) + 2*(l2*cos(th2)*sin(th1)*th1d + l2*cos(th1)*sin(th2)*th2d - l3*cos(th1)*cos(th2)*cos(th3)*th3d + l3*cos(th2)*sin(th1)*sin(th3)*th1d + l3*cos(th1)*sin(th2)*sin(th3)*th2d + (l4*cos(th1)*cos(th2)*cos(th3)*cos(delta - th4)*th3d)/2 - (l4*cos(th2)*sin(th1)*sin(th3)*cos(delta - th4)*th1d)/2 - (l4*cos(th1)*sin(th2)*sin(th3)*cos(delta - th4)*th2d)/2 + (l4*cos(th1)*cos(th2)*sin(th3)*sin(delta - th4)*th4d)/2)*(- l2*cos(th1)*cos(th2)*th1d + l2*sin(th1)*sin(th2)*th2d - l3*cos(th1)*cos(th2)*sin(th3)*th1d - l3*cos(th2)*cos(th3)*sin(th1)*th3d + l3*sin(th1)*sin(th2)*sin(th3)*th2d - (l4*sin(th1)*sin(th2)*sin(th3)*cos(delta - th4)*th2d)/2 + (l4*cos(th2)*sin(th1)*sin(th3)*sin(delta - th4)*th4d)/2 + (l4*cos(th1)*cos(th2)*sin(th3)*cos(delta - th4)*th1d)/2 + (l4*cos(th2)*cos(th3)*sin(th1)*cos(delta - th4)*th3d)/2)))/2)/(l1_Izz + l2_Izz + l3_Izz + l4_Izz + l5_Izz + (m2*((l2^2*cos(th1)^2*cos(th2)^2)/2 + (l2^2*cos(th2)^2*sin(th1)^2)/2))/2 + (m4*(2*(l2*cos(th1)*cos(th2) + l3*cos(th1)*cos(th2)*sin(th3) - (l4*cos(th2)*sin(th1)*sin(th3)*cos(delta - th4))/2)^2 + 2*(l2*cos(th2)*sin(th1) + l3*cos(th2)*sin(th1)*sin(th3) - (l4*cos(th2)*sin(th1)*sin(th3)*cos(delta - th4))/2)^2))/2 + (m5*(2*(l2*cos(th1)*cos(th2) + l3*cos(th1)*cos(th2)*sin(th3) + (l4*cos(th1)*cos(th2)*sin(th3)*cos(delta - th4))/2 - (l4*cos(th2)*sin(th1)*sin(th3)*cos(delta - th4))/2 + (l5*cos(th1)*cos(th2)*cos(th5)*sin(th3)*cos(delta - th4))/2)^2 + 2*(l2*cos(th2)*sin(th1) + l3*cos(th2)*sin(th1)*sin(th3) - l4*cos(th2)*sin(th1)*sin(th3)*cos(delta - th4) - (l5*cos(th2)*cos(th5)*sin(th1)*sin(th3)*cos(delta - th4))/2)^2))/2 + (m3*(2*(l2*cos(th2)*sin(th1) + (l3*cos(th2)*sin(th1)*sin(th3))/2)^2 + 2*(l2*cos(th1)*cos(th2) + (l3*cos(th1)*cos(th2)*sin(th3))/2)^2))/2);
 
th2dd = -(- u2 - (m2*(l2^2*cos(th2)*sin(th2)*th2d^2 - l2*sin(th1)*sin(th2)*((l2*cos(th2)*sin(th1)*th1d^2)/2 + (l2*cos(th2)*sin(th1)*th2d^2)/2 - (l2*cos(th1)*cos(th2)*th1dd)/2 + l2*cos(th1)*sin(th2)*th2d*th1d) - l2*cos(th1)*sin(th2)*((l2*cos(th1)*cos(th2)*th1d^2)/2 + (l2*cos(th1)*cos(th2)*th2d^2)/2 + (l2*cos(th2)*sin(th1)*th1dd)/2 - l2*sin(th1)*sin(th2)*th2d*th1d) + l2*sin(th1)*sin(th2)*((l2*cos(th2)*sin(th1)*th1d)/2 + (l2*cos(th1)*sin(th2)*th2d)/2)*th1d - l2*cos(th1)*cos(th2)*((l2*cos(th2)*sin(th1)*th1d)/2 + (l2*cos(th1)*sin(th2)*th2d)/2)*th2d + l2*cos(th1)*sin(th2)*((l2*cos(th1)*cos(th2)*th1d)/2 - (l2*sin(th1)*sin(th2)*th2d)/2)*th1d + l2*cos(th2)*sin(th1)*((l2*cos(th1)*cos(th2)*th1d)/2 - (l2*sin(th1)*sin(th2)*th2d)/2)*th2d))/2 - (m5*(2*(2*l2*cos(th2) + (l3*sin(th2 + th3))/2 + (l3*cos(th3)*sin(th2))/2 - (l4*sin(delta - th4)*sin(th2 + th3))/2 - (l4*cos(th3)*sin(th2)*sin(delta - th4))/2 - (l5*cos(th3)*sin(th2)*sin(th5)*sin(delta - th4))/2)*(2*l2*sin(th2)*th2d^2 - (l3*cos(th2 + th3)*(th2d + th3d)^2)/2 - (l3*sin(th2 + th3)*th3dd)/2 + (l4*cos(delta - th4)*cos(th2 + th3)*th4dd)/2 + (l4*sin(delta - th4)*cos(th2 + th3)*(th2d + th3d)^2)/2 + (l4*sin(delta - th4)*sin(th2 + th3)*th3dd)/2 - (l3*cos(th2)*cos(th3)*th2d^2)/2 - (l3*cos(th2)*cos(th3)*th3d^2)/2 - (l3*cos(th2)*sin(th3)*th3dd)/2 + (l4*sin(delta - th4)*cos(th2 + th3)*th4d^2)/2 + (l4*cos(th2)*cos(th3)*sin(delta - th4)*th2d^2)/2 + (l4*cos(th2)*cos(th3)*sin(delta - th4)*th3d^2)/2 + (l4*cos(th2)*cos(th3)*sin(delta - th4)*th4d^2)/2 + l3*sin(th2)*sin(th3)*th3d*th2d + (l4*cos(th2)*cos(th3)*cos(delta - th4)*th4dd)/2 + (l4*cos(th2)*sin(th3)*sin(delta - th4)*th3dd)/2 - l4*cos(delta - th4)*sin(th2 + th3)*(th2d + th3d)*th4d + (l5*cos(th2)*cos(th3)*sin(th5)*sin(delta - th4)*th2d^2)/2 + (l5*cos(th2)*cos(th3)*sin(th5)*sin(delta - th4)*th3d^2)/2 + (l5*cos(th2)*cos(th3)*sin(th5)*sin(delta - th4)*th4d^2)/2 + (l5*cos(th2)*cos(th3)*sin(th5)*sin(delta - th4)*th5d^2)/2 + (l5*cos(th2)*cos(th3)*sin(th5)*cos(delta - th4)*th4dd)/2 - (l5*cos(th2)*cos(th3)*cos(th5)*sin(delta - th4)*th5dd)/2 - l4*cos(th3)*sin(th2)*cos(delta - th4)*th4d*th2d - l4*cos(th2)*sin(th3)*cos(delta - th4)*th4d*th3d + (l5*cos(th2)*sin(th3)*sin(th5)*sin(delta - th4)*th3dd)/2 - l4*sin(th2)*sin(th3)*sin(delta - th4)*th3d*th2d + l5*cos(th2)*cos(th3)*cos(th5)*cos(delta - th4)*th5d*th4d - l5*cos(th3)*sin(th2)*sin(th5)*cos(delta - th4)*th4d*th2d - l5*cos(th2)*sin(th3)*sin(th5)*cos(delta - th4)*th4d*th3d + l5*cos(th3)*cos(th5)*sin(th2)*sin(delta - th4)*th5d*th2d + l5*cos(th2)*cos(th5)*sin(th3)*sin(delta - th4)*th5d*th3d - l5*sin(th2)*sin(th3)*sin(th5)*sin(delta - th4)*th3d*th2d) - 2*(l2*sin(th1)*sin(th2) + l3*sin(th1)*sin(th2)*sin(th3) + (l4*cos(th1)*sin(th2)*sin(th3)*cos(delta - th4))/2 + (l4*sin(th1)*sin(th2)*sin(th3)*cos(delta - th4))/2 + (l5*cos(th5)*sin(th1)*sin(th2)*sin(th3)*cos(delta - th4))/2)*(l2*cos(th2)*sin(th1)*th1d^2 + l2*cos(th2)*sin(th1)*th2d^2 - l2*cos(th1)*cos(th2)*th1dd + l3*cos(th2)*sin(th1)*sin(th3)*th1d^2 + l3*cos(th2)*sin(th1)*sin(th3)*th2d^2 + l3*cos(th2)*sin(th1)*sin(th3)*th3d^2 - l3*cos(th1)*cos(th2)*sin(th3)*th1dd - l3*cos(th2)*cos(th3)*sin(th1)*th3dd + 2*l2*cos(th1)*sin(th2)*th2d*th1d - 2*l3*cos(th1)*cos(th2)*cos(th3)*th3d*th1d + (l4*cos(th1)*cos(th2)*sin(th3)*cos(delta - th4)*th1d^2)/2 + (l4*cos(th1)*cos(th2)*sin(th3)*cos(delta - th4)*th2d^2)/2 + (l4*cos(th1)*cos(th2)*sin(th3)*cos(delta - th4)*th3d^2)/2 + (l4*cos(th1)*cos(th2)*sin(th3)*cos(delta - th4)*th4d^2)/2 + 2*l3*cos(th1)*sin(th2)*sin(th3)*th2d*th1d + 2*l3*cos(th3)*sin(th1)*sin(th2)*th3d*th2d - (l4*cos(th1)*cos(th2)*cos(th3)*cos(delta - th4)*th3dd)/2 + (l4*cos(th2)*sin(th1)*sin(th3)*cos(delta - th4)*th1d^2)/2 + (l4*cos(th2)*sin(th1)*sin(th3)*cos(delta - th4)*th2d^2)/2 + (l4*cos(th2)*sin(th1)*sin(th3)*cos(delta - th4)*th3d^2)/2 + (l4*cos(th2)*sin(th1)*sin(th3)*cos(delta - th4)*th4d^2)/2 - (l4*cos(th1)*cos(th2)*sin(th3)*cos(delta - th4)*th1dd)/2 - (l4*cos(th2)*cos(th3)*sin(th1)*cos(delta - th4)*th3dd)/2 + (l4*cos(th2)*sin(th1)*sin(th3)*cos(delta - th4)*th1dd)/2 - (l4*cos(th1)*cos(th2)*sin(th3)*sin(delta - th4)*th4dd)/2 - (l4*cos(th2)*sin(th1)*sin(th3)*sin(delta - th4)*th4dd)/2 - l4*cos(th1)*cos(th2)*cos(th3)*cos(delta - th4)*th3d*th1d + (l5*cos(th2)*cos(th5)*sin(th1)*sin(th3)*cos(delta - th4)*th1d^2)/2 + (l5*cos(th2)*cos(th5)*sin(th1)*sin(th3)*cos(delta - th4)*th2d^2)/2 + (l5*cos(th2)*cos(th5)*sin(th1)*sin(th3)*cos(delta - th4)*th3d^2)/2 + (l5*cos(th2)*cos(th5)*sin(th1)*sin(th3)*cos(delta - th4)*th4d^2)/2 + (l5*cos(th2)*cos(th5)*sin(th1)*sin(th3)*cos(delta - th4)*th5d^2)/2 - (l5*cos(th1)*cos(th2)*cos(th5)*sin(th3)*cos(delta - th4)*th1dd)/2 - (l5*cos(th2)*cos(th3)*cos(th5)*sin(th1)*cos(delta - th4)*th3dd)/2 + l4*cos(th2)*cos(th3)*sin(th1)*cos(delta - th4)*th3d*th1d + l4*cos(th1)*cos(th3)*sin(th2)*cos(delta - th4)*th3d*th2d - l4*cos(th1)*cos(th2)*cos(th3)*sin(delta - th4)*th4d*th3d + l4*cos(th1)*sin(th2)*sin(th3)*cos(delta - th4)*th2d*th1d - l4*cos(th1)*cos(th2)*sin(th3)*sin(delta - th4)*th4d*th1d + l4*cos(th3)*sin(th1)*sin(th2)*cos(delta - th4)*th3d*th2d - l4*cos(th2)*cos(th3)*sin(th1)*sin(delta - th4)*th4d*th3d - (l5*cos(th2)*cos(th5)*sin(th1)*sin(th3)*sin(delta - th4)*th4dd)/2 + (l5*cos(th2)*sin(th1)*sin(th3)*sin(th5)*cos(delta - th4)*th5dd)/2 - l4*sin(th1)*sin(th2)*sin(th3)*cos(delta - th4)*th2d*th1d + l4*cos(th2)*sin(th1)*sin(th3)*sin(delta - th4)*th4d*th1d + l4*cos(th1)*sin(th2)*sin(th3)*sin(delta - th4)*th4d*th2d + l4*sin(th1)*sin(th2)*sin(th3)*sin(delta - th4)*th4d*th2d + l5*cos(th1)*cos(th5)*sin(th2)*sin(th3)*cos(delta - th4)*th2d*th1d - l5*cos(th1)*cos(th2)*cos(th5)*sin(th3)*sin(delta - th4)*th4d*th1d + l5*cos(th3)*cos(th5)*sin(th1)*sin(th2)*cos(delta - th4)*th3d*th2d + l5*cos(th1)*cos(th2)*sin(th3)*sin(th5)*cos(delta - th4)*th5d*th1d - l5*cos(th2)*cos(th3)*cos(th5)*sin(th1)*sin(delta - th4)*th4d*th3d + l5*cos(th2)*cos(th3)*sin(th1)*sin(th5)*cos(delta - th4)*th5d*th3d + l5*cos(th5)*sin(th1)*sin(th2)*sin(th3)*sin(delta - th4)*th4d*th2d - l5*sin(th1)*sin(th2)*sin(th3)*sin(th5)*cos(delta - th4)*th5d*th2d + l5*cos(th2)*sin(th1)*sin(th3)*sin(th5)*sin(delta - th4)*th5d*th4d - l5*cos(th1)*cos(th2)*cos(th3)*cos(th5)*cos(delta - th4)*th3d*th1d) + 2*((l4*cos(delta - th4)*cos(th2 + th3)*th4d)/2 - 2*l2*cos(th2)*th2d - (l3*cos(th3)*sin(th2)*th2d)/2 - (l3*cos(th2)*sin(th3)*th3d)/2 - (l3*sin(th2 + th3)*(th2d + th3d))/2 + (l4*sin(delta - th4)*sin(th2 + th3)*(th2d + th3d))/2 + (l4*cos(th2)*cos(th3)*cos(delta - th4)*th4d)/2 + (l4*cos(th3)*sin(th2)*sin(delta - th4)*th2d)/2 + (l4*cos(th2)*sin(th3)*sin(delta - th4)*th3d)/2 + (l5*cos(th3)*sin(th2)*sin(th5)*sin(delta - th4)*th2d)/2 + (l5*cos(th2)*sin(th3)*sin(th5)*sin(delta - th4)*th3d)/2 + (l5*cos(th2)*cos(th3)*sin(th5)*cos(delta - th4)*th4d)/2 - (l5*cos(th2)*cos(th3)*cos(th5)*sin(delta - th4)*th5d)/2)*((l3*cos(th2 + th3)*(th2d + th3d))/2 - 2*l2*sin(th2)*th2d + (l3*cos(th2)*cos(th3)*th2d)/2 - (l3*sin(th2)*sin(th3)*th3d)/2 + (l4*cos(delta - th4)*sin(th2 + th3)*th4d)/2 - (l4*sin(delta - th4)*cos(th2 + th3)*(th2d + th3d))/2 - (l4*cos(th2)*cos(th3)*sin(delta - th4)*th2d)/2 + (l4*cos(th3)*sin(th2)*cos(delta - th4)*th4d)/2 + (l4*sin(th2)*sin(th3)*sin(delta - th4)*th3d)/2 + (l5*sin(th2)*sin(th3)*sin(th5)*sin(delta - th4)*th3d)/2 - (l5*cos(th2)*cos(th3)*sin(th5)*sin(delta - th4)*th2d)/2 + (l5*cos(th3)*sin(th2)*sin(th5)*cos(delta - th4)*th4d)/2 - (l5*cos(th3)*cos(th5)*sin(th2)*sin(delta - th4)*th5d)/2) + 2*(l2*cos(th1)*sin(th2)*th1d + l2*cos(th2)*sin(th1)*th2d + l3*cos(th1)*sin(th2)*sin(th3)*th1d + l3*cos(th2)*sin(th1)*sin(th3)*th2d + l3*cos(th3)*sin(th1)*sin(th2)*th3d - (l4*sin(th1)*sin(th2)*sin(th3)*cos(delta - th4)*th1d)/2 + (l4*cos(th1)*sin(th2)*sin(th3)*sin(delta - th4)*th4d)/2 + (l4*sin(th1)*sin(th2)*sin(th3)*sin(delta - th4)*th4d)/2 + (l4*cos(th1)*cos(th2)*sin(th3)*cos(delta - th4)*th2d)/2 + (l4*cos(th1)*cos(th3)*sin(th2)*cos(delta - th4)*th3d)/2 + (l4*cos(th1)*sin(th2)*sin(th3)*cos(delta - th4)*th1d)/2 + (l4*cos(th2)*sin(th1)*sin(th3)*cos(delta - th4)*th2d)/2 + (l4*cos(th3)*sin(th1)*sin(th2)*cos(delta - th4)*th3d)/2 + (l5*cos(th1)*cos(th5)*sin(th2)*sin(th3)*cos(delta - th4)*th1d)/2 + (l5*cos(th2)*cos(th5)*sin(th1)*sin(th3)*cos(delta - th4)*th2d)/2 + (l5*cos(th3)*cos(th5)*sin(th1)*sin(th2)*cos(delta - th4)*th3d)/2 + (l5*cos(th5)*sin(th1)*sin(th2)*sin(th3)*sin(delta - th4)*th4d)/2 - (l5*sin(th1)*sin(th2)*sin(th3)*sin(th5)*cos(delta - th4)*th5d)/2)*(l2*cos(th1)*cos(th2)*th1d - l2*sin(th1)*sin(th2)*th2d + l3*cos(th1)*cos(th2)*sin(th3)*th1d + l3*cos(th2)*cos(th3)*sin(th1)*th3d - l3*sin(th1)*sin(th2)*sin(th3)*th2d - (l4*sin(th1)*sin(th2)*sin(th3)*cos(delta - th4)*th2d)/2 + (l4*cos(th2)*sin(th1)*sin(th3)*sin(delta - th4)*th4d)/2 + (l4*cos(th1)*cos(th2)*cos(th3)*cos(delta - th4)*th3d)/2 + (l4*cos(th1)*cos(th2)*sin(th3)*cos(delta - th4)*th1d)/2 + (l4*cos(th2)*cos(th3)*sin(th1)*cos(delta - th4)*th3d)/2 - (l4*cos(th2)*sin(th1)*sin(th3)*cos(delta - th4)*th1d)/2 - (l4*cos(th1)*sin(th2)*sin(th3)*cos(delta - th4)*th2d)/2 + (l4*cos(th1)*cos(th2)*sin(th3)*sin(delta - th4)*th4d)/2 + (l5*cos(th1)*cos(th2)*cos(th5)*sin(th3)*cos(delta - th4)*th1d)/2 + (l5*cos(th2)*cos(th3)*cos(th5)*sin(th1)*cos(delta - th4)*th3d)/2 - (l5*cos(th5)*sin(th1)*sin(th2)*sin(th3)*cos(delta - th4)*th2d)/2 + (l5*cos(th2)*cos(th5)*sin(th1)*sin(th3)*sin(delta - th4)*th4d)/2 - (l5*cos(th2)*sin(th1)*sin(th3)*sin(th5)*cos(delta - th4)*th5d)/2) + 2*(l2*cos(th1)*sin(th2) + l3*cos(th1)*sin(th2)*sin(th3) - l4*cos(th1)*sin(th2)*sin(th3)*cos(delta - th4) - (l5*cos(th1)*cos(th5)*sin(th2)*sin(th3)*cos(delta - th4))/2)*(2*l2*sin(th1)*sin(th2)*th2d*th1d - l2*cos(th1)*cos(th2)*th2d^2 - l2*cos(th2)*sin(th1)*th1dd - l3*cos(th2)*sin(th1)*sin(th3)*th1dd - l2*cos(th1)*cos(th2)*th1d^2 - l3*cos(th1)*cos(th2)*sin(th3)*th1d^2 - l3*cos(th1)*cos(th2)*sin(th3)*th2d^2 - l3*cos(th1)*cos(th2)*sin(th3)*th3d^2 + l3*cos(th1)*cos(th2)*cos(th3)*th3dd - 2*l3*cos(th2)*cos(th3)*sin(th1)*th3d*th1d - 2*l3*cos(th1)*cos(th3)*sin(th2)*th3d*th2d + l4*cos(th1)*cos(th2)*sin(th3)*cos(delta - th4)*th1d^2 + l4*cos(th1)*cos(th2)*sin(th3)*cos(delta - th4)*th2d^2 + l4*cos(th1)*cos(th2)*sin(th3)*cos(delta - th4)*th3d^2 + l4*cos(th1)*cos(th2)*sin(th3)*cos(delta - th4)*th4d^2 - l4*cos(th1)*cos(th2)*cos(th3)*cos(delta - th4)*th3dd + 2*l3*sin(th1)*sin(th2)*sin(th3)*th2d*th1d + l4*cos(th2)*sin(th1)*sin(th3)*cos(delta - th4)*th1dd - l4*cos(th1)*cos(th2)*sin(th3)*sin(delta - th4)*th4dd + (l5*cos(th1)*cos(th2)*cos(th5)*sin(th3)*cos(delta - th4)*th1d^2)/2 + (l5*cos(th1)*cos(th2)*cos(th5)*sin(th3)*cos(delta - th4)*th2d^2)/2 + (l5*cos(th1)*cos(th2)*cos(th5)*sin(th3)*cos(delta - th4)*th3d^2)/2 + (l5*cos(th1)*cos(th2)*cos(th5)*sin(th3)*cos(delta - th4)*th4d^2)/2 + (l5*cos(th1)*cos(th2)*cos(th5)*sin(th3)*cos(delta - th4)*th5d^2)/2 - (l5*cos(th1)*cos(th2)*cos(th3)*cos(th5)*cos(delta - th4)*th3dd)/2 + 2*l4*cos(th2)*cos(th3)*sin(th1)*cos(delta - th4)*th3d*th1d + 2*l4*cos(th1)*cos(th3)*sin(th2)*cos(delta - th4)*th3d*th2d - 2*l4*cos(th1)*cos(th2)*cos(th3)*sin(delta - th4)*th4d*th3d + (l5*cos(th2)*cos(th5)*sin(th1)*sin(th3)*cos(delta - th4)*th1dd)/2 - (l5*cos(th1)*cos(th2)*cos(th5)*sin(th3)*sin(delta - th4)*th4dd)/2 + (l5*cos(th1)*cos(th2)*sin(th3)*sin(th5)*cos(delta - th4)*th5dd)/2 - 2*l4*sin(th1)*sin(th2)*sin(th3)*cos(delta - th4)*th2d*th1d + 2*l4*cos(th2)*sin(th1)*sin(th3)*sin(delta - th4)*th4d*th1d + 2*l4*cos(th1)*sin(th2)*sin(th3)*sin(delta - th4)*th4d*th2d - l5*cos(th5)*sin(th1)*sin(th2)*sin(th3)*cos(delta - th4)*th2d*th1d + l5*cos(th2)*cos(th5)*sin(th1)*sin(th3)*sin(delta - th4)*th4d*th1d + l5*cos(th1)*cos(th5)*sin(th2)*sin(th3)*sin(delta - th4)*th4d*th2d - l5*cos(th2)*sin(th1)*sin(th3)*sin(th5)*cos(delta - th4)*th5d*th1d - l5*cos(th1)*sin(th2)*sin(th3)*sin(th5)*cos(delta - th4)*th5d*th2d + l5*cos(th1)*cos(th2)*sin(th3)*sin(th5)*sin(delta - th4)*th5d*th4d + l5*cos(th2)*cos(th3)*cos(th5)*sin(th1)*cos(delta - th4)*th3d*th1d + l5*cos(th1)*cos(th3)*cos(th5)*sin(th2)*cos(delta - th4)*th3d*th2d - l5*cos(th1)*cos(th2)*cos(th3)*cos(th5)*sin(delta - th4)*th4d*th3d + l5*cos(th1)*cos(th2)*cos(th3)*sin(th5)*cos(delta - th4)*th5d*th3d) + 2*(l2*cos(th2)*sin(th1)*th1d + l2*cos(th1)*sin(th2)*th2d - l3*cos(th1)*cos(th2)*cos(th3)*th3d + l3*cos(th2)*sin(th1)*sin(th3)*th1d + l3*cos(th1)*sin(th2)*sin(th3)*th2d + l4*cos(th1)*cos(th2)*cos(th3)*cos(delta - th4)*th3d - l4*cos(th2)*sin(th1)*sin(th3)*cos(delta - th4)*th1d - l4*cos(th1)*sin(th2)*sin(th3)*cos(delta - th4)*th2d + l4*cos(th1)*cos(th2)*sin(th3)*sin(delta - th4)*th4d + (l5*cos(th1)*cos(th2)*cos(th3)*cos(th5)*cos(delta - th4)*th3d)/2 - (l5*cos(th2)*cos(th5)*sin(th1)*sin(th3)*cos(delta - th4)*th1d)/2 - (l5*cos(th1)*cos(th5)*sin(th2)*sin(th3)*cos(delta - th4)*th2d)/2 + (l5*cos(th1)*cos(th2)*cos(th5)*sin(th3)*sin(delta - th4)*th4d)/2 - (l5*cos(th1)*cos(th2)*sin(th3)*sin(th5)*cos(delta - th4)*th5d)/2)*(l2*sin(th1)*sin(th2)*th1d - l2*cos(th1)*cos(th2)*th2d - l3*cos(th1)*cos(th2)*sin(th3)*th2d - l3*cos(th1)*cos(th3)*sin(th2)*th3d + l3*sin(th1)*sin(th2)*sin(th3)*th1d - l4*sin(th1)*sin(th2)*sin(th3)*cos(delta - th4)*th1d + l4*cos(th1)*sin(th2)*sin(th3)*sin(delta - th4)*th4d + l4*cos(th1)*cos(th2)*sin(th3)*cos(delta - th4)*th2d + l4*cos(th1)*cos(th3)*sin(th2)*cos(delta - th4)*th3d + (l5*cos(th1)*cos(th2)*cos(th5)*sin(th3)*cos(delta - th4)*th2d)/2 + (l5*cos(th1)*cos(th3)*cos(th5)*sin(th2)*cos(delta - th4)*th3d)/2 - (l5*cos(th5)*sin(th1)*sin(th2)*sin(th3)*cos(delta - th4)*th1d)/2 + (l5*cos(th1)*cos(th5)*sin(th2)*sin(th3)*sin(delta - th4)*th4d)/2 - (l5*cos(th1)*sin(th2)*sin(th3)*sin(th5)*cos(delta - th4)*th5d)/2)))/2 + (m4*(2*(l2*cos(th1)*cos(th2)*th1d - l2*sin(th1)*sin(th2)*th2d + l3*cos(th1)*cos(th2)*sin(th3)*th1d + l3*cos(th2)*cos(th3)*sin(th1)*th3d - l3*sin(th1)*sin(th2)*sin(th3)*th2d + (l4*cos(th1)*cos(th2)*cos(th3)*cos(delta - th4)*th3d)/2 - (l4*cos(th2)*sin(th1)*sin(th3)*cos(delta - th4)*th1d)/2 - (l4*cos(th1)*sin(th2)*sin(th3)*cos(delta - th4)*th2d)/2 + (l4*cos(th1)*cos(th2)*sin(th3)*sin(delta - th4)*th4d)/2)*(l2*cos(th1)*sin(th2)*th1d + l2*cos(th2)*sin(th1)*th2d + l3*cos(th1)*sin(th2)*sin(th3)*th1d + l3*cos(th2)*sin(th1)*sin(th3)*th2d + l3*cos(th3)*sin(th1)*sin(th2)*th3d - (l4*sin(th1)*sin(th2)*sin(th3)*cos(delta - th4)*th1d)/2 + (l4*cos(th1)*sin(th2)*sin(th3)*sin(delta - th4)*th4d)/2 + (l4*cos(th1)*cos(th2)*sin(th3)*cos(delta - th4)*th2d)/2 + (l4*cos(th1)*cos(th3)*sin(th2)*cos(delta - th4)*th3d)/2) + 2*(l2*cos(th2)*sin(th1)*th1d + l2*cos(th1)*sin(th2)*th2d - l3*cos(th1)*cos(th2)*cos(th3)*th3d + l3*cos(th2)*sin(th1)*sin(th3)*th1d + l3*cos(th1)*sin(th2)*sin(th3)*th2d + (l4*cos(th1)*cos(th2)*cos(th3)*cos(delta - th4)*th3d)/2 - (l4*cos(th2)*sin(th1)*sin(th3)*cos(delta - th4)*th1d)/2 - (l4*cos(th1)*sin(th2)*sin(th3)*cos(delta - th4)*th2d)/2 + (l4*cos(th1)*cos(th2)*sin(th3)*sin(delta - th4)*th4d)/2)*(- l2*cos(th1)*cos(th2)*th2d + l2*sin(th1)*sin(th2)*th1d - l3*cos(th1)*cos(th2)*sin(th3)*th2d - l3*cos(th1)*cos(th3)*sin(th2)*th3d + l3*sin(th1)*sin(th2)*sin(th3)*th1d - (l4*sin(th1)*sin(th2)*sin(th3)*cos(delta - th4)*th1d)/2 + (l4*cos(th1)*sin(th2)*sin(th3)*sin(delta - th4)*th4d)/2 + (l4*cos(th1)*cos(th2)*sin(th3)*cos(delta - th4)*th2d)/2 + (l4*cos(th1)*cos(th3)*sin(th2)*cos(delta - th4)*th3d)/2) - 2*((l3*cos(th2 + th3)*(th2d + th3d))/2 - 2*l2*sin(th2)*th2d + (l3*cos(th2)*cos(th3)*th2d)/2 - (l3*sin(th2)*sin(th3)*th3d)/2 + (l4*cos(delta - th4)*sin(th2 + th3)*th4d)/2 - (l4*sin(delta - th4)*cos(th2 + th3)*(th2d + th3d))/2)*((l3*sin(th2 + th3)*(th2d + th3d))/2 + 2*l2*cos(th2)*th2d + (l3*cos(th3)*sin(th2)*th2d)/2 + (l3*cos(th2)*sin(th3)*th3d)/2 - (l4*cos(delta - th4)*cos(th2 + th3)*th4d)/2 - (l4*sin(delta - th4)*sin(th2 + th3)*(th2d + th3d))/2)))/2 + (m3*(2*(l2*cos(th2)*sin(th1)*th1d + l2*cos(th1)*sin(th2)*th2d - (l3*cos(th1)*cos(th2)*cos(th3)*th3d)/2 + (l3*cos(th2)*sin(th1)*sin(th3)*th1d)/2 + (l3*cos(th1)*sin(th2)*sin(th3)*th2d)/2)*(l2*cos(th1)*cos(th2)*th2d - l2*sin(th1)*sin(th2)*th1d + (l3*cos(th1)*cos(th2)*sin(th3)*th2d)/2 + (l3*cos(th1)*cos(th3)*sin(th2)*th3d)/2 - (l3*sin(th1)*sin(th2)*sin(th3)*th1d)/2) + 2*(2*l2*cos(th2) + (l3*sin(th2 + th3))/2)*(- 2*l2*sin(th2)*th2d^2 + (l3*cos(th2 + th3)*(th2d + th3d)^2)/2 + (l3*sin(th2 + th3)*th3dd)/2) - 2*(l2*cos(th1)*cos(th2)*th1d - l2*sin(th1)*sin(th2)*th2d + (l3*cos(th1)*cos(th2)*sin(th3)*th1d)/2 + (l3*cos(th2)*cos(th3)*sin(th1)*th3d)/2 - (l3*sin(th1)*sin(th2)*sin(th3)*th2d)/2)*(l2*cos(th1)*sin(th2)*th1d + l2*cos(th2)*sin(th1)*th2d + (l3*cos(th1)*sin(th2)*sin(th3)*th1d)/2 + (l3*cos(th2)*sin(th1)*sin(th3)*th2d)/2 + (l3*cos(th3)*sin(th1)*sin(th2)*th3d)/2) + 2*((l3*cos(th2 + th3)*(th2d + th3d))/2 - 2*l2*sin(th2)*th2d)*((l3*sin(th2 + th3)*(th2d + th3d))/2 + 2*l2*cos(th2)*th2d) + 2*(l2*cos(th1)*sin(th2) + (l3*cos(th1)*sin(th2)*sin(th3))/2)*(l2*cos(th1)*cos(th2)*th1d^2 + l2*cos(th1)*cos(th2)*th2d^2 + l2*cos(th2)*sin(th1)*th1dd + (l3*cos(th2)*sin(th1)*sin(th3)*th1dd)/2 - 2*l2*sin(th1)*sin(th2)*th2d*th1d + (l3*cos(th1)*cos(th2)*sin(th3)*th1d^2)/2 + (l3*cos(th1)*cos(th2)*sin(th3)*th2d^2)/2 + (l3*cos(th1)*cos(th2)*sin(th3)*th3d^2)/2 - (l3*cos(th1)*cos(th2)*cos(th3)*th3dd)/2 + l3*cos(th2)*cos(th3)*sin(th1)*th3d*th1d + l3*cos(th1)*cos(th3)*sin(th2)*th3d*th2d - l3*sin(th1)*sin(th2)*sin(th3)*th2d*th1d) + 2*(l2*sin(th1)*sin(th2) + (l3*sin(th1)*sin(th2)*sin(th3))/2)*(l2*cos(th2)*sin(th1)*th1d^2 + l2*cos(th2)*sin(th1)*th2d^2 - l2*cos(th1)*cos(th2)*th1dd + (l3*cos(th2)*sin(th1)*sin(th3)*th1d^2)/2 + (l3*cos(th2)*sin(th1)*sin(th3)*th2d^2)/2 + (l3*cos(th2)*sin(th1)*sin(th3)*th3d^2)/2 - (l3*cos(th1)*cos(th2)*sin(th3)*th1dd)/2 - (l3*cos(th2)*cos(th3)*sin(th1)*th3dd)/2 + 2*l2*cos(th1)*sin(th2)*th2d*th1d - l3*cos(th1)*cos(th2)*cos(th3)*th3d*th1d + l3*cos(th1)*sin(th2)*sin(th3)*th2d*th1d + l3*cos(th3)*sin(th1)*sin(th2)*th3d*th2d)))/2 + (m5*(2*(- (l3*sin(th2 + th3)*(th2d + th3d))/2 - 2*l2*cos(th2)*th2d - (l3*cos(th3)*sin(th2)*th2d)/2 - (l3*cos(th2)*sin(th3)*th3d)/2 + (l4*cos(delta - th4)*cos(th2 + th3)*th4d)/2 + (l4*sin(delta - th4)*sin(th2 + th3)*(th2d + th3d))/2 + (l4*cos(th2)*cos(th3)*cos(delta - th4)*th4d)/2 + (l4*cos(th3)*sin(th2)*sin(delta - th4)*th2d)/2 + (l4*cos(th2)*sin(th3)*sin(delta - th4)*th3d)/2 + (l5*cos(th3)*sin(th2)*sin(th5)*sin(delta - th4)*th2d)/2 + (l5*cos(th2)*sin(th3)*sin(th5)*sin(delta - th4)*th3d)/2 + (l5*cos(th2)*cos(th3)*sin(th5)*cos(delta - th4)*th4d)/2 - (l5*cos(th2)*cos(th3)*cos(th5)*sin(delta - th4)*th5d)/2)*((l3*cos(th2 + th3)*(th2d + th3d))/2 - 2*l2*sin(th2)*th2d + (l3*cos(th2)*cos(th3)*th2d)/2 - (l3*sin(th2)*sin(th3)*th3d)/2 + (l4*cos(delta - th4)*sin(th2 + th3)*th4d)/2 - (l4*sin(delta - th4)*cos(th2 + th3)*(th2d + th3d))/2 - (l4*cos(th2)*cos(th3)*sin(delta - th4)*th2d)/2 + (l4*cos(th3)*sin(th2)*cos(delta - th4)*th4d)/2 + (l4*sin(th2)*sin(th3)*sin(delta - th4)*th3d)/2 + (l5*sin(th2)*sin(th3)*sin(th5)*sin(delta - th4)*th3d)/2 - (l5*cos(th2)*cos(th3)*sin(th5)*sin(delta - th4)*th2d)/2 + (l5*cos(th3)*sin(th2)*sin(th5)*cos(delta - th4)*th4d)/2 - (l5*cos(th3)*cos(th5)*sin(th2)*sin(delta - th4)*th5d)/2) + 2*(l2*cos(th1)*sin(th2)*th1d + l2*cos(th2)*sin(th1)*th2d + l3*cos(th1)*sin(th2)*sin(th3)*th1d + l3*cos(th2)*sin(th1)*sin(th3)*th2d + l3*cos(th3)*sin(th1)*sin(th2)*th3d - (l4*sin(th1)*sin(th2)*sin(th3)*cos(delta - th4)*th1d)/2 + (l4*cos(th1)*sin(th2)*sin(th3)*sin(delta - th4)*th4d)/2 + (l4*sin(th1)*sin(th2)*sin(th3)*sin(delta - th4)*th4d)/2 + (l4*cos(th1)*cos(th2)*sin(th3)*cos(delta - th4)*th2d)/2 + (l4*cos(th1)*cos(th3)*sin(th2)*cos(delta - th4)*th3d)/2 + (l4*cos(th1)*sin(th2)*sin(th3)*cos(delta - th4)*th1d)/2 + (l4*cos(th2)*sin(th1)*sin(th3)*cos(delta - th4)*th2d)/2 + (l4*cos(th3)*sin(th1)*sin(th2)*cos(delta - th4)*th3d)/2 + (l5*cos(th1)*cos(th5)*sin(th2)*sin(th3)*cos(delta - th4)*th1d)/2 + (l5*cos(th2)*cos(th5)*sin(th1)*sin(th3)*cos(delta - th4)*th2d)/2 + (l5*cos(th3)*cos(th5)*sin(th1)*sin(th2)*cos(delta - th4)*th3d)/2 + (l5*cos(th5)*sin(th1)*sin(th2)*sin(th3)*sin(delta - th4)*th4d)/2 - (l5*sin(th1)*sin(th2)*sin(th3)*sin(th5)*cos(delta - th4)*th5d)/2)*(l2*cos(th1)*cos(th2)*th1d - l2*sin(th1)*sin(th2)*th2d + l3*cos(th1)*cos(th2)*sin(th3)*th1d + l3*cos(th2)*cos(th3)*sin(th1)*th3d - l3*sin(th1)*sin(th2)*sin(th3)*th2d - (l4*sin(th1)*sin(th2)*sin(th3)*cos(delta - th4)*th2d)/2 + (l4*cos(th2)*sin(th1)*sin(th3)*sin(delta - th4)*th4d)/2 + (l4*cos(th1)*cos(th2)*cos(th3)*cos(delta - th4)*th3d)/2 + (l4*cos(th1)*cos(th2)*sin(th3)*cos(delta - th4)*th1d)/2 + (l4*cos(th2)*cos(th3)*sin(th1)*cos(delta - th4)*th3d)/2 - (l4*cos(th2)*sin(th1)*sin(th3)*cos(delta - th4)*th1d)/2 - (l4*cos(th1)*sin(th2)*sin(th3)*cos(delta - th4)*th2d)/2 + (l4*cos(th1)*cos(th2)*sin(th3)*sin(delta - th4)*th4d)/2 + (l5*cos(th1)*cos(th2)*cos(th5)*sin(th3)*cos(delta - th4)*th1d)/2 + (l5*cos(th2)*cos(th3)*cos(th5)*sin(th1)*cos(delta - th4)*th3d)/2 - (l5*cos(th5)*sin(th1)*sin(th2)*sin(th3)*cos(delta - th4)*th2d)/2 + (l5*cos(th2)*cos(th5)*sin(th1)*sin(th3)*sin(delta - th4)*th4d)/2 - (l5*cos(th2)*sin(th1)*sin(th3)*sin(th5)*cos(delta - th4)*th5d)/2) + 2*(l2*cos(th2)*sin(th1)*th1d + l2*cos(th1)*sin(th2)*th2d - l3*cos(th1)*cos(th2)*cos(th3)*th3d + l3*cos(th2)*sin(th1)*sin(th3)*th1d + l3*cos(th1)*sin(th2)*sin(th3)*th2d + l4*cos(th1)*cos(th2)*cos(th3)*cos(delta - th4)*th3d - l4*cos(th2)*sin(th1)*sin(th3)*cos(delta - th4)*th1d - l4*cos(th1)*sin(th2)*sin(th3)*cos(delta - th4)*th2d + l4*cos(th1)*cos(th2)*sin(th3)*sin(delta - th4)*th4d + (l5*cos(th1)*cos(th2)*cos(th3)*cos(th5)*cos(delta - th4)*th3d)/2 - (l5*cos(th2)*cos(th5)*sin(th1)*sin(th3)*cos(delta - th4)*th1d)/2 - (l5*cos(th1)*cos(th5)*sin(th2)*sin(th3)*cos(delta - th4)*th2d)/2 + (l5*cos(th1)*cos(th2)*cos(th5)*sin(th3)*sin(delta - th4)*th4d)/2 - (l5*cos(th1)*cos(th2)*sin(th3)*sin(th5)*cos(delta - th4)*th5d)/2)*(- l2*cos(th1)*cos(th2)*th2d + l2*sin(th1)*sin(th2)*th1d - l3*cos(th1)*cos(th2)*sin(th3)*th2d - l3*cos(th1)*cos(th3)*sin(th2)*th3d + l3*sin(th1)*sin(th2)*sin(th3)*th1d - l4*sin(th1)*sin(th2)*sin(th3)*cos(delta - th4)*th1d + l4*cos(th1)*sin(th2)*sin(th3)*sin(delta - th4)*th4d + l4*cos(th1)*cos(th2)*sin(th3)*cos(delta - th4)*th2d + l4*cos(th1)*cos(th3)*sin(th2)*cos(delta - th4)*th3d + (l5*cos(th1)*cos(th2)*cos(th5)*sin(th3)*cos(delta - th4)*th2d)/2 + (l5*cos(th1)*cos(th3)*cos(th5)*sin(th2)*cos(delta - th4)*th3d)/2 - (l5*cos(th5)*sin(th1)*sin(th2)*sin(th3)*cos(delta - th4)*th1d)/2 + (l5*cos(th1)*cos(th5)*sin(th2)*sin(th3)*sin(delta - th4)*th4d)/2 - (l5*cos(th1)*sin(th2)*sin(th3)*sin(th5)*cos(delta - th4)*th5d)/2)))/2 + beta2*th2d - (m4*(2*(2*l2*cos(th2) + (l3*sin(th2 + th3))/2 + (l3*cos(th3)*sin(th2))/2 - (l4*sin(delta - th4)*sin(th2 + th3))/2)*(2*l2*sin(th2)*th2d^2 - (l3*cos(th2 + th3)*(th2d + th3d)^2)/2 - (l3*sin(th2 + th3)*th3dd)/2 + (l4*cos(delta - th4)*cos(th2 + th3)*th4dd)/2 + (l4*sin(delta - th4)*cos(th2 + th3)*(th2d + th3d)^2)/2 + (l4*sin(delta - th4)*sin(th2 + th3)*th3dd)/2 - (l3*cos(th2)*cos(th3)*th2d^2)/2 - (l3*cos(th2)*cos(th3)*th3d^2)/2 - (l3*cos(th2)*sin(th3)*th3dd)/2 + (l4*sin(delta - th4)*cos(th2 + th3)*th4d^2)/2 + l3*sin(th2)*sin(th3)*th3d*th2d - l4*cos(delta - th4)*sin(th2 + th3)*(th2d + th3d)*th4d) + 2*(l2*cos(th1)*cos(th2)*th1d - l2*sin(th1)*sin(th2)*th2d + l3*cos(th1)*cos(th2)*sin(th3)*th1d + l3*cos(th2)*cos(th3)*sin(th1)*th3d - l3*sin(th1)*sin(th2)*sin(th3)*th2d + (l4*cos(th1)*cos(th2)*cos(th3)*cos(delta - th4)*th3d)/2 - (l4*cos(th2)*sin(th1)*sin(th3)*cos(delta - th4)*th1d)/2 - (l4*cos(th1)*sin(th2)*sin(th3)*cos(delta - th4)*th2d)/2 + (l4*cos(th1)*cos(th2)*sin(th3)*sin(delta - th4)*th4d)/2)*(l2*cos(th1)*sin(th2)*th1d + l2*cos(th2)*sin(th1)*th2d + l3*cos(th1)*sin(th2)*sin(th3)*th1d + l3*cos(th2)*sin(th1)*sin(th3)*th2d + l3*cos(th3)*sin(th1)*sin(th2)*th3d - (l4*sin(th1)*sin(th2)*sin(th3)*cos(delta - th4)*th1d)/2 + (l4*cos(th1)*sin(th2)*sin(th3)*sin(delta - th4)*th4d)/2 + (l4*cos(th1)*cos(th2)*sin(th3)*cos(delta - th4)*th2d)/2 + (l4*cos(th1)*cos(th3)*sin(th2)*cos(delta - th4)*th3d)/2) - 2*(l2*cos(th1)*sin(th2) + l3*cos(th1)*sin(th2)*sin(th3) - (l4*cos(th1)*sin(th2)*sin(th3)*cos(delta - th4))/2)*(l2*cos(th1)*cos(th2)*th1d^2 + l2*cos(th1)*cos(th2)*th2d^2 + l2*cos(th2)*sin(th1)*th1dd + l3*cos(th2)*sin(th1)*sin(th3)*th1dd - 2*l2*sin(th1)*sin(th2)*th2d*th1d + l3*cos(th1)*cos(th2)*sin(th3)*th1d^2 + l3*cos(th1)*cos(th2)*sin(th3)*th2d^2 + l3*cos(th1)*cos(th2)*sin(th3)*th3d^2 - l3*cos(th1)*cos(th2)*cos(th3)*th3dd + 2*l3*cos(th2)*cos(th3)*sin(th1)*th3d*th1d + 2*l3*cos(th1)*cos(th3)*sin(th2)*th3d*th2d - (l4*cos(th1)*cos(th2)*sin(th3)*cos(delta - th4)*th1d^2)/2 - (l4*cos(th1)*cos(th2)*sin(th3)*cos(delta - th4)*th2d^2)/2 - (l4*cos(th1)*cos(th2)*sin(th3)*cos(delta - th4)*th3d^2)/2 - (l4*cos(th1)*cos(th2)*sin(th3)*cos(delta - th4)*th4d^2)/2 + (l4*cos(th1)*cos(th2)*cos(th3)*cos(delta - th4)*th3dd)/2 - 2*l3*sin(th1)*sin(th2)*sin(th3)*th2d*th1d - (l4*cos(th2)*sin(th1)*sin(th3)*cos(delta - th4)*th1dd)/2 + (l4*cos(th1)*cos(th2)*sin(th3)*sin(delta - th4)*th4dd)/2 - l4*cos(th2)*cos(th3)*sin(th1)*cos(delta - th4)*th3d*th1d - l4*cos(th1)*cos(th3)*sin(th2)*cos(delta - th4)*th3d*th2d + l4*cos(th1)*cos(th2)*cos(th3)*sin(delta - th4)*th4d*th3d + l4*sin(th1)*sin(th2)*sin(th3)*cos(delta - th4)*th2d*th1d - l4*cos(th2)*sin(th1)*sin(th3)*sin(delta - th4)*th4d*th1d - l4*cos(th1)*sin(th2)*sin(th3)*sin(delta - th4)*th4d*th2d) - 2*(l2*sin(th1)*sin(th2) + l3*sin(th1)*sin(th2)*sin(th3) + (l4*cos(th1)*sin(th2)*sin(th3)*cos(delta - th4))/2)*(l2*cos(th2)*sin(th1)*th1d^2 + l2*cos(th2)*sin(th1)*th2d^2 - l2*cos(th1)*cos(th2)*th1dd + l3*cos(th2)*sin(th1)*sin(th3)*th1d^2 + l3*cos(th2)*sin(th1)*sin(th3)*th2d^2 + l3*cos(th2)*sin(th1)*sin(th3)*th3d^2 - l3*cos(th1)*cos(th2)*sin(th3)*th1dd - l3*cos(th2)*cos(th3)*sin(th1)*th3dd + 2*l2*cos(th1)*sin(th2)*th2d*th1d - 2*l3*cos(th1)*cos(th2)*cos(th3)*th3d*th1d + (l4*cos(th1)*cos(th2)*sin(th3)*cos(delta - th4)*th1d^2)/2 + (l4*cos(th1)*cos(th2)*sin(th3)*cos(delta - th4)*th2d^2)/2 + (l4*cos(th1)*cos(th2)*sin(th3)*cos(delta - th4)*th3d^2)/2 + (l4*cos(th1)*cos(th2)*sin(th3)*cos(delta - th4)*th4d^2)/2 + 2*l3*cos(th1)*sin(th2)*sin(th3)*th2d*th1d + 2*l3*cos(th3)*sin(th1)*sin(th2)*th3d*th2d - (l4*cos(th1)*cos(th2)*cos(th3)*cos(delta - th4)*th3dd)/2 + (l4*cos(th2)*sin(th1)*sin(th3)*cos(delta - th4)*th1dd)/2 - (l4*cos(th1)*cos(th2)*sin(th3)*sin(delta - th4)*th4dd)/2 + l4*cos(th2)*cos(th3)*sin(th1)*cos(delta - th4)*th3d*th1d + l4*cos(th1)*cos(th3)*sin(th2)*cos(delta - th4)*th3d*th2d - l4*cos(th1)*cos(th2)*cos(th3)*sin(delta - th4)*th4d*th3d - l4*sin(th1)*sin(th2)*sin(th3)*cos(delta - th4)*th2d*th1d + l4*cos(th2)*sin(th1)*sin(th3)*sin(delta - th4)*th4d*th1d + l4*cos(th1)*sin(th2)*sin(th3)*sin(delta - th4)*th4d*th2d) + 2*(l2*cos(th2)*sin(th1)*th1d + l2*cos(th1)*sin(th2)*th2d - l3*cos(th1)*cos(th2)*cos(th3)*th3d + l3*cos(th2)*sin(th1)*sin(th3)*th1d + l3*cos(th1)*sin(th2)*sin(th3)*th2d + (l4*cos(th1)*cos(th2)*cos(th3)*cos(delta - th4)*th3d)/2 - (l4*cos(th2)*sin(th1)*sin(th3)*cos(delta - th4)*th1d)/2 - (l4*cos(th1)*sin(th2)*sin(th3)*cos(delta - th4)*th2d)/2 + (l4*cos(th1)*cos(th2)*sin(th3)*sin(delta - th4)*th4d)/2)*(l2*sin(th1)*sin(th2)*th1d - l2*cos(th1)*cos(th2)*th2d - l3*cos(th1)*cos(th2)*sin(th3)*th2d - l3*cos(th1)*cos(th3)*sin(th2)*th3d + l3*sin(th1)*sin(th2)*sin(th3)*th1d - (l4*sin(th1)*sin(th2)*sin(th3)*cos(delta - th4)*th1d)/2 + (l4*cos(th1)*sin(th2)*sin(th3)*sin(delta - th4)*th4d)/2 + (l4*cos(th1)*cos(th2)*sin(th3)*cos(delta - th4)*th2d)/2 + (l4*cos(th1)*cos(th3)*sin(th2)*cos(delta - th4)*th3d)/2) - 2*((l3*cos(th2 + th3)*(th2d + th3d))/2 - 2*l2*sin(th2)*th2d + (l3*cos(th2)*cos(th3)*th2d)/2 - (l3*sin(th2)*sin(th3)*th3d)/2 + (l4*cos(delta - th4)*sin(th2 + th3)*th4d)/2 - (l4*sin(delta - th4)*cos(th2 + th3)*(th2d + th3d))/2)*((l3*sin(th2 + th3)*(th2d + th3d))/2 + 2*l2*cos(th2)*th2d + (l3*cos(th3)*sin(th2)*th2d)/2 + (l3*cos(th2)*sin(th3)*th3d)/2 - (l4*cos(delta - th4)*cos(th2 + th3)*th4d)/2 - (l4*sin(delta - th4)*sin(th2 + th3)*(th2d + th3d))/2)))/2 - (m3*(2*(l2*cos(th2)*sin(th1)*th1d + l2*cos(th1)*sin(th2)*th2d - (l3*cos(th1)*cos(th2)*cos(th3)*th3d)/2 + (l3*cos(th2)*sin(th1)*sin(th3)*th1d)/2 + (l3*cos(th1)*sin(th2)*sin(th3)*th2d)/2)*(l2*cos(th1)*cos(th2)*th2d - l2*sin(th1)*sin(th2)*th1d + (l3*cos(th1)*cos(th2)*sin(th3)*th2d)/2 + (l3*cos(th1)*cos(th3)*sin(th2)*th3d)/2 - (l3*sin(th1)*sin(th2)*sin(th3)*th1d)/2) - 2*(l2*cos(th1)*cos(th2)*th1d - l2*sin(th1)*sin(th2)*th2d + (l3*cos(th1)*cos(th2)*sin(th3)*th1d)/2 + (l3*cos(th2)*cos(th3)*sin(th1)*th3d)/2 - (l3*sin(th1)*sin(th2)*sin(th3)*th2d)/2)*(l2*cos(th1)*sin(th2)*th1d + l2*cos(th2)*sin(th1)*th2d + (l3*cos(th1)*sin(th2)*sin(th3)*th1d)/2 + (l3*cos(th2)*sin(th1)*sin(th3)*th2d)/2 + (l3*cos(th3)*sin(th1)*sin(th2)*th3d)/2) + 2*((l3*cos(th2 + th3)*(th2d + th3d))/2 - 2*l2*sin(th2)*th2d)*((l3*sin(th2 + th3)*(th2d + th3d))/2 + 2*l2*cos(th2)*th2d)))/2 + (m2*(2*((l2*cos(th1)*cos(th2)*th1d)/2 - (l2*sin(th1)*sin(th2)*th2d)/2)*((l2*cos(th1)*sin(th2)*th1d)/2 + (l2*cos(th2)*sin(th1)*th2d)/2) - 2*((l2*cos(th1)*cos(th2)*th2d)/2 - (l2*sin(th1)*sin(th2)*th1d)/2)*((l2*cos(th2)*sin(th1)*th1d)/2 + (l2*cos(th1)*sin(th2)*th2d)/2) + (l2^2*cos(th2)*sin(th2)*th2d^2)/2))/2 + g*m5*(l2*cos(th2) - l3*cos(th3)*sin(th2) + l4*cos(th3)*sin(th2)*sin(delta - th4) + (l5*cos(th3)*sin(th2)*sin(delta - th4))/2) + g*m4*(l2*cos(th2) - l3*cos(th3)*sin(th2) + (l4*cos(th3)*sin(th2)*sin(delta - th4))/2) + g*m3*(l2*cos(th2) - (l3*cos(th3)*sin(th2))/2) + (g*l2*m2*cos(th2))/2)/(l2_Izz + l3_Izz + l4_Izz + l5_Izz + (m2*((l2^2*cos(th1)^2*sin(th2)^2)/2 + (l2^2*cos(th2)^2)/2 + (l2^2*sin(th1)^2*sin(th2)^2)/2))/2 + (m5*(2*(l2*sin(th1)*sin(th2) + l3*sin(th1)*sin(th2)*sin(th3) + (l4*cos(th1)*sin(th2)*sin(th3)*cos(delta - th4))/2 + (l4*sin(th1)*sin(th2)*sin(th3)*cos(delta - th4))/2 + (l5*cos(th5)*sin(th1)*sin(th2)*sin(th3)*cos(delta - th4))/2)^2 + 2*(l2*cos(th1)*sin(th2) + l3*cos(th1)*sin(th2)*sin(th3) - l4*cos(th1)*sin(th2)*sin(th3)*cos(delta - th4) - (l5*cos(th1)*cos(th5)*sin(th2)*sin(th3)*cos(delta - th4))/2)^2 + 2*(2*l2*cos(th2) + (l3*sin(th2 + th3))/2 + (l3*cos(th3)*sin(th2))/2 - (l4*sin(delta - th4)*sin(th2 + th3))/2 - (l4*cos(th3)*sin(th2)*sin(delta - th4))/2 - (l5*cos(th3)*sin(th2)*sin(th5)*sin(delta - th4))/2)^2))/2 + (m4*(2*(l2*cos(th1)*sin(th2) + l3*cos(th1)*sin(th2)*sin(th3) - (l4*cos(th1)*sin(th2)*sin(th3)*cos(delta - th4))/2)^2 + 2*(l2*sin(th1)*sin(th2) + l3*sin(th1)*sin(th2)*sin(th3) + (l4*cos(th1)*sin(th2)*sin(th3)*cos(delta - th4))/2)^2 + 2*(2*l2*cos(th2) + (l3*sin(th2 + th3))/2 + (l3*cos(th3)*sin(th2))/2 - (l4*sin(delta - th4)*sin(th2 + th3))/2)^2))/2 + (m3*(2*(l2*cos(th1)*sin(th2) + (l3*cos(th1)*sin(th2)*sin(th3))/2)^2 + 2*(l2*sin(th1)*sin(th2) + (l3*sin(th1)*sin(th2)*sin(th3))/2)^2 + 2*(2*l2*cos(th2) + (l3*sin(th2 + th3))/2)^2))/2);

th3dd = (u3 + (m3*(2*((l3*cos(th2)*cos(th3)*sin(th1)*th1d)/2 + (l3*cos(th1)*cos(th3)*sin(th2)*th2d)/2 + (l3*cos(th1)*cos(th2)*sin(th3)*th3d)/2)*(l2*cos(th2)*sin(th1)*th1d + l2*cos(th1)*sin(th2)*th2d - (l3*cos(th1)*cos(th2)*cos(th3)*th3d)/2 + (l3*cos(th2)*sin(th1)*sin(th3)*th1d)/2 + (l3*cos(th1)*sin(th2)*sin(th3)*th2d)/2) - 2*(- (l3*cos(th1)*cos(th2)*cos(th3)*th1d)/2 + (l3*cos(th3)*sin(th1)*sin(th2)*th2d)/2 + (l3*cos(th2)*sin(th1)*sin(th3)*th3d)/2)*(l2*cos(th1)*cos(th2)*th1d - l2*sin(th1)*sin(th2)*th2d + (l3*cos(th1)*cos(th2)*sin(th3)*th1d)/2 + (l3*cos(th2)*cos(th3)*sin(th1)*th3d)/2 - (l3*sin(th1)*sin(th2)*sin(th3)*th2d)/2) + l3*cos(th2 + th3)*((l3*sin(th2 + th3)*(th2d + th3d))/2 + 2*l2*cos(th2)*th2d)*(th2d + th3d)))/2 + (m5*(2*((l3*cos(th2 + th3)*(th2d + th3d))/2 + (l3*cos(th2)*cos(th3)*th3d)/2 - (l3*sin(th2)*sin(th3)*th2d)/2 + (l4*cos(delta - th4)*sin(th2 + th3)*th4d)/2 - (l4*sin(delta - th4)*cos(th2 + th3)*(th2d + th3d))/2 - (l4*cos(th2)*cos(th3)*sin(delta - th4)*th3d)/2 + (l4*cos(th2)*sin(th3)*cos(delta - th4)*th4d)/2 + (l4*sin(th2)*sin(th3)*sin(delta - th4)*th2d)/2 + (l5*sin(th2)*sin(th3)*sin(th5)*sin(delta - th4)*th2d)/2 - (l5*cos(th2)*cos(th3)*sin(th5)*sin(delta - th4)*th3d)/2 + (l5*cos(th2)*sin(th3)*sin(th5)*cos(delta - th4)*th4d)/2 - (l5*cos(th2)*cos(th5)*sin(th3)*sin(delta - th4)*th5d)/2)*((l4*cos(delta - th4)*cos(th2 + th3)*th4d)/2 - 2*l2*cos(th2)*th2d - (l3*cos(th3)*sin(th2)*th2d)/2 - (l3*cos(th2)*sin(th3)*th3d)/2 - (l3*sin(th2 + th3)*(th2d + th3d))/2 + (l4*sin(delta - th4)*sin(th2 + th3)*(th2d + th3d))/2 + (l4*cos(th2)*cos(th3)*cos(delta - th4)*th4d)/2 + (l4*cos(th3)*sin(th2)*sin(delta - th4)*th2d)/2 + (l4*cos(th2)*sin(th3)*sin(delta - th4)*th3d)/2 + (l5*cos(th3)*sin(th2)*sin(th5)*sin(delta - th4)*th2d)/2 + (l5*cos(th2)*sin(th3)*sin(th5)*sin(delta - th4)*th3d)/2 + (l5*cos(th2)*cos(th3)*sin(th5)*cos(delta - th4)*th4d)/2 - (l5*cos(th2)*cos(th3)*cos(th5)*sin(delta - th4)*th5d)/2) - 2*((l4*sin(delta - th4)*sin(th2 + th3))/2 - (l3*cos(th2)*sin(th3))/2 - (l3*sin(th2 + th3))/2 + (l4*cos(th2)*sin(th3)*sin(delta - th4))/2 + (l5*cos(th2)*sin(th3)*sin(th5)*sin(delta - th4))/2)*(2*l2*sin(th2)*th2d^2 - 2*l2*cos(th2)*th2dd - (l3*cos(th2 + th3)*(th2d + th3d)^2)/2 - (l3*sin(th2 + th3)*th2dd)/2 + (l4*cos(delta - th4)*cos(th2 + th3)*th4dd)/2 + (l4*sin(delta - th4)*cos(th2 + th3)*(th2d + th3d)^2)/2 + (l4*sin(delta - th4)*sin(th2 + th3)*th2dd)/2 - (l3*cos(th2)*cos(th3)*th2d^2)/2 - (l3*cos(th2)*cos(th3)*th3d^2)/2 - (l3*cos(th3)*sin(th2)*th2dd)/2 + (l4*sin(delta - th4)*cos(th2 + th3)*th4d^2)/2 + (l4*cos(th2)*cos(th3)*sin(delta - th4)*th2d^2)/2 + (l4*cos(th2)*cos(th3)*sin(delta - th4)*th3d^2)/2 + (l4*cos(th2)*cos(th3)*sin(delta - th4)*th4d^2)/2 + l3*sin(th2)*sin(th3)*th3d*th2d + (l4*cos(th2)*cos(th3)*cos(delta - th4)*th4dd)/2 + (l4*cos(th3)*sin(th2)*sin(delta - th4)*th2dd)/2 - l4*cos(delta - th4)*sin(th2 + th3)*(th2d + th3d)*th4d + (l5*cos(th2)*cos(th3)*sin(th5)*sin(delta - th4)*th2d^2)/2 + (l5*cos(th2)*cos(th3)*sin(th5)*sin(delta - th4)*th3d^2)/2 + (l5*cos(th2)*cos(th3)*sin(th5)*sin(delta - th4)*th4d^2)/2 + (l5*cos(th2)*cos(th3)*sin(th5)*sin(delta - th4)*th5d^2)/2 + (l5*cos(th2)*cos(th3)*sin(th5)*cos(delta - th4)*th4dd)/2 - (l5*cos(th2)*cos(th3)*cos(th5)*sin(delta - th4)*th5dd)/2 - l4*cos(th3)*sin(th2)*cos(delta - th4)*th4d*th2d - l4*cos(th2)*sin(th3)*cos(delta - th4)*th4d*th3d + (l5*cos(th3)*sin(th2)*sin(th5)*sin(delta - th4)*th2dd)/2 - l4*sin(th2)*sin(th3)*sin(delta - th4)*th3d*th2d + l5*cos(th2)*cos(th3)*cos(th5)*cos(delta - th4)*th5d*th4d - l5*cos(th3)*sin(th2)*sin(th5)*cos(delta - th4)*th4d*th2d - l5*cos(th2)*sin(th3)*sin(th5)*cos(delta - th4)*th4d*th3d + l5*cos(th3)*cos(th5)*sin(th2)*sin(delta - th4)*th5d*th2d + l5*cos(th2)*cos(th5)*sin(th3)*sin(delta - th4)*th5d*th3d - l5*sin(th2)*sin(th3)*sin(th5)*sin(delta - th4)*th3d*th2d) + 2*(l3*cos(th2)*cos(th3)*sin(th1) + (l4*cos(th1)*cos(th2)*cos(th3)*cos(delta - th4))/2 + (l4*cos(th2)*cos(th3)*sin(th1)*cos(delta - th4))/2 + (l5*cos(th2)*cos(th3)*cos(th5)*sin(th1)*cos(delta - th4))/2)*(l2*cos(th2)*sin(th1)*th1d^2 + l2*cos(th2)*sin(th1)*th2d^2 - l2*cos(th1)*cos(th2)*th1dd + l2*sin(th1)*sin(th2)*th2dd + l3*sin(th1)*sin(th2)*sin(th3)*th2dd + l3*cos(th2)*sin(th1)*sin(th3)*th1d^2 + l3*cos(th2)*sin(th1)*sin(th3)*th2d^2 + l3*cos(th2)*sin(th1)*sin(th3)*th3d^2 - l3*cos(th1)*cos(th2)*sin(th3)*th1dd + 2*l2*cos(th1)*sin(th2)*th2d*th1d - 2*l3*cos(th1)*cos(th2)*cos(th3)*th3d*th1d + (l4*cos(th1)*cos(th2)*sin(th3)*cos(delta - th4)*th1d^2)/2 + (l4*cos(th1)*cos(th2)*sin(th3)*cos(delta - th4)*th2d^2)/2 + (l4*cos(th1)*cos(th2)*sin(th3)*cos(delta - th4)*th3d^2)/2 + (l4*cos(th1)*cos(th2)*sin(th3)*cos(delta - th4)*th4d^2)/2 + 2*l3*cos(th1)*sin(th2)*sin(th3)*th2d*th1d + 2*l3*cos(th3)*sin(th1)*sin(th2)*th3d*th2d + (l4*cos(th2)*sin(th1)*sin(th3)*cos(delta - th4)*th1d^2)/2 + (l4*cos(th2)*sin(th1)*sin(th3)*cos(delta - th4)*th2d^2)/2 + (l4*cos(th2)*sin(th1)*sin(th3)*cos(delta - th4)*th3d^2)/2 + (l4*cos(th2)*sin(th1)*sin(th3)*cos(delta - th4)*th4d^2)/2 - (l4*cos(th1)*cos(th2)*sin(th3)*cos(delta - th4)*th1dd)/2 + (l4*cos(th2)*sin(th1)*sin(th3)*cos(delta - th4)*th1dd)/2 + (l4*cos(th1)*sin(th2)*sin(th3)*cos(delta - th4)*th2dd)/2 - (l4*cos(th1)*cos(th2)*sin(th3)*sin(delta - th4)*th4dd)/2 + (l4*sin(th1)*sin(th2)*sin(th3)*cos(delta - th4)*th2dd)/2 - (l4*cos(th2)*sin(th1)*sin(th3)*sin(delta - th4)*th4dd)/2 - l4*cos(th1)*cos(th2)*cos(th3)*cos(delta - th4)*th3d*th1d + (l5*cos(th2)*cos(th5)*sin(th1)*sin(th3)*cos(delta - th4)*th1d^2)/2 + (l5*cos(th2)*cos(th5)*sin(th1)*sin(th3)*cos(delta - th4)*th2d^2)/2 + (l5*cos(th2)*cos(th5)*sin(th1)*sin(th3)*cos(delta - th4)*th3d^2)/2 + (l5*cos(th2)*cos(th5)*sin(th1)*sin(th3)*cos(delta - th4)*th4d^2)/2 + (l5*cos(th2)*cos(th5)*sin(th1)*sin(th3)*cos(delta - th4)*th5d^2)/2 - (l5*cos(th1)*cos(th2)*cos(th5)*sin(th3)*cos(delta - th4)*th1dd)/2 + l4*cos(th2)*cos(th3)*sin(th1)*cos(delta - th4)*th3d*th1d + l4*cos(th1)*cos(th3)*sin(th2)*cos(delta - th4)*th3d*th2d - l4*cos(th1)*cos(th2)*cos(th3)*sin(delta - th4)*th4d*th3d + l4*cos(th1)*sin(th2)*sin(th3)*cos(delta - th4)*th2d*th1d - l4*cos(th1)*cos(th2)*sin(th3)*sin(delta - th4)*th4d*th1d + l4*cos(th3)*sin(th1)*sin(th2)*cos(delta - th4)*th3d*th2d - l4*cos(th2)*cos(th3)*sin(th1)*sin(delta - th4)*th4d*th3d + (l5*cos(th5)*sin(th1)*sin(th2)*sin(th3)*cos(delta - th4)*th2dd)/2 - (l5*cos(th2)*cos(th5)*sin(th1)*sin(th3)*sin(delta - th4)*th4dd)/2 + (l5*cos(th2)*sin(th1)*sin(th3)*sin(th5)*cos(delta - th4)*th5dd)/2 - l4*sin(th1)*sin(th2)*sin(th3)*cos(delta - th4)*th2d*th1d + l4*cos(th2)*sin(th1)*sin(th3)*sin(delta - th4)*th4d*th1d + l4*cos(th1)*sin(th2)*sin(th3)*sin(delta - th4)*th4d*th2d + l4*sin(th1)*sin(th2)*sin(th3)*sin(delta - th4)*th4d*th2d + l5*cos(th1)*cos(th5)*sin(th2)*sin(th3)*cos(delta - th4)*th2d*th1d - l5*cos(th1)*cos(th2)*cos(th5)*sin(th3)*sin(delta - th4)*th4d*th1d + l5*cos(th3)*cos(th5)*sin(th1)*sin(th2)*cos(delta - th4)*th3d*th2d + l5*cos(th1)*cos(th2)*sin(th3)*sin(th5)*cos(delta - th4)*th5d*th1d - l5*cos(th2)*cos(th3)*cos(th5)*sin(th1)*sin(delta - th4)*th4d*th3d + l5*cos(th2)*cos(th3)*sin(th1)*sin(th5)*cos(delta - th4)*th5d*th3d + l5*cos(th5)*sin(th1)*sin(th2)*sin(th3)*sin(delta - th4)*th4d*th2d - l5*sin(th1)*sin(th2)*sin(th3)*sin(th5)*cos(delta - th4)*th5d*th2d + l5*cos(th2)*sin(th1)*sin(th3)*sin(th5)*sin(delta - th4)*th5d*th4d - l5*cos(th1)*cos(th2)*cos(th3)*cos(th5)*cos(delta - th4)*th3d*th1d) + 2*(l4*cos(th2)*cos(th3)*sin(th1)*cos(delta - th4)*th1d - l3*cos(th1)*cos(th3)*sin(th2)*th2d - l3*cos(th1)*cos(th2)*sin(th3)*th3d - l3*cos(th2)*cos(th3)*sin(th1)*th1d + l4*cos(th1)*cos(th3)*sin(th2)*cos(delta - th4)*th2d + l4*cos(th1)*cos(th2)*sin(th3)*cos(delta - th4)*th3d - l4*cos(th1)*cos(th2)*cos(th3)*sin(delta - th4)*th4d + (l5*cos(th2)*cos(th3)*cos(th5)*sin(th1)*cos(delta - th4)*th1d)/2 + (l5*cos(th1)*cos(th3)*cos(th5)*sin(th2)*cos(delta - th4)*th2d)/2 + (l5*cos(th1)*cos(th2)*cos(th5)*sin(th3)*cos(delta - th4)*th3d)/2 - (l5*cos(th1)*cos(th2)*cos(th3)*cos(th5)*sin(delta - th4)*th4d)/2 + (l5*cos(th1)*cos(th2)*cos(th3)*sin(th5)*cos(delta - th4)*th5d)/2)*(l2*cos(th2)*sin(th1)*th1d + l2*cos(th1)*sin(th2)*th2d - l3*cos(th1)*cos(th2)*cos(th3)*th3d + l3*cos(th2)*sin(th1)*sin(th3)*th1d + l3*cos(th1)*sin(th2)*sin(th3)*th2d + l4*cos(th1)*cos(th2)*cos(th3)*cos(delta - th4)*th3d - l4*cos(th2)*sin(th1)*sin(th3)*cos(delta - th4)*th1d - l4*cos(th1)*sin(th2)*sin(th3)*cos(delta - th4)*th2d + l4*cos(th1)*cos(th2)*sin(th3)*sin(delta - th4)*th4d + (l5*cos(th1)*cos(th2)*cos(th3)*cos(th5)*cos(delta - th4)*th3d)/2 - (l5*cos(th2)*cos(th5)*sin(th1)*sin(th3)*cos(delta - th4)*th1d)/2 - (l5*cos(th1)*cos(th5)*sin(th2)*sin(th3)*cos(delta - th4)*th2d)/2 + (l5*cos(th1)*cos(th2)*cos(th5)*sin(th3)*sin(delta - th4)*th4d)/2 - (l5*cos(th1)*cos(th2)*sin(th3)*sin(th5)*cos(delta - th4)*th5d)/2) + 2*(l4*cos(th1)*cos(th2)*cos(th3)*cos(delta - th4) - l3*cos(th1)*cos(th2)*cos(th3) + (l5*cos(th1)*cos(th2)*cos(th3)*cos(th5)*cos(delta - th4))/2)*(2*l2*sin(th1)*sin(th2)*th2d*th1d - l2*cos(th1)*cos(th2)*th2d^2 - l2*cos(th2)*sin(th1)*th1dd - l2*cos(th1)*sin(th2)*th2dd - l3*cos(th2)*sin(th1)*sin(th3)*th1dd - l3*cos(th1)*sin(th2)*sin(th3)*th2dd - l2*cos(th1)*cos(th2)*th1d^2 - l3*cos(th1)*cos(th2)*sin(th3)*th1d^2 - l3*cos(th1)*cos(th2)*sin(th3)*th2d^2 - l3*cos(th1)*cos(th2)*sin(th3)*th3d^2 - 2*l3*cos(th2)*cos(th3)*sin(th1)*th3d*th1d - 2*l3*cos(th1)*cos(th3)*sin(th2)*th3d*th2d + l4*cos(th1)*cos(th2)*sin(th3)*cos(delta - th4)*th1d^2 + l4*cos(th1)*cos(th2)*sin(th3)*cos(delta - th4)*th2d^2 + l4*cos(th1)*cos(th2)*sin(th3)*cos(delta - th4)*th3d^2 + l4*cos(th1)*cos(th2)*sin(th3)*cos(delta - th4)*th4d^2 + 2*l3*sin(th1)*sin(th2)*sin(th3)*th2d*th1d + l4*cos(th2)*sin(th1)*sin(th3)*cos(delta - th4)*th1dd + l4*cos(th1)*sin(th2)*sin(th3)*cos(delta - th4)*th2dd - l4*cos(th1)*cos(th2)*sin(th3)*sin(delta - th4)*th4dd + (l5*cos(th1)*cos(th2)*cos(th5)*sin(th3)*cos(delta - th4)*th1d^2)/2 + (l5*cos(th1)*cos(th2)*cos(th5)*sin(th3)*cos(delta - th4)*th2d^2)/2 + (l5*cos(th1)*cos(th2)*cos(th5)*sin(th3)*cos(delta - th4)*th3d^2)/2 + (l5*cos(th1)*cos(th2)*cos(th5)*sin(th3)*cos(delta - th4)*th4d^2)/2 + (l5*cos(th1)*cos(th2)*cos(th5)*sin(th3)*cos(delta - th4)*th5d^2)/2 + 2*l4*cos(th2)*cos(th3)*sin(th1)*cos(delta - th4)*th3d*th1d + 2*l4*cos(th1)*cos(th3)*sin(th2)*cos(delta - th4)*th3d*th2d - 2*l4*cos(th1)*cos(th2)*cos(th3)*sin(delta - th4)*th4d*th3d + (l5*cos(th2)*cos(th5)*sin(th1)*sin(th3)*cos(delta - th4)*th1dd)/2 + (l5*cos(th1)*cos(th5)*sin(th2)*sin(th3)*cos(delta - th4)*th2dd)/2 - (l5*cos(th1)*cos(th2)*cos(th5)*sin(th3)*sin(delta - th4)*th4dd)/2 + (l5*cos(th1)*cos(th2)*sin(th3)*sin(th5)*cos(delta - th4)*th5dd)/2 - 2*l4*sin(th1)*sin(th2)*sin(th3)*cos(delta - th4)*th2d*th1d + 2*l4*cos(th2)*sin(th1)*sin(th3)*sin(delta - th4)*th4d*th1d + 2*l4*cos(th1)*sin(th2)*sin(th3)*sin(delta - th4)*th4d*th2d - l5*cos(th5)*sin(th1)*sin(th2)*sin(th3)*cos(delta - th4)*th2d*th1d + l5*cos(th2)*cos(th5)*sin(th1)*sin(th3)*sin(delta - th4)*th4d*th1d + l5*cos(th1)*cos(th5)*sin(th2)*sin(th3)*sin(delta - th4)*th4d*th2d - l5*cos(th2)*sin(th1)*sin(th3)*sin(th5)*cos(delta - th4)*th5d*th1d - l5*cos(th1)*sin(th2)*sin(th3)*sin(th5)*cos(delta - th4)*th5d*th2d + l5*cos(th1)*cos(th2)*sin(th3)*sin(th5)*sin(delta - th4)*th5d*th4d + l5*cos(th2)*cos(th3)*cos(th5)*sin(th1)*cos(delta - th4)*th3d*th1d + l5*cos(th1)*cos(th3)*cos(th5)*sin(th2)*cos(delta - th4)*th3d*th2d - l5*cos(th1)*cos(th2)*cos(th3)*cos(th5)*sin(delta - th4)*th4d*th3d + l5*cos(th1)*cos(th2)*cos(th3)*sin(th5)*cos(delta - th4)*th5d*th3d) + 2*(l3*cos(th3)*sin(th1)*sin(th2)*th2d - l3*cos(th1)*cos(th2)*cos(th3)*th1d + l3*cos(th2)*sin(th1)*sin(th3)*th3d - (l4*cos(th1)*cos(th2)*cos(th3)*cos(delta - th4)*th1d)/2 + (l4*cos(th2)*cos(th3)*sin(th1)*cos(delta - th4)*th1d)/2 + (l4*cos(th1)*cos(th3)*sin(th2)*cos(delta - th4)*th2d)/2 + (l4*cos(th1)*cos(th2)*sin(th3)*cos(delta - th4)*th3d)/2 - (l4*cos(th1)*cos(th2)*cos(th3)*sin(delta - th4)*th4d)/2 + (l4*cos(th3)*sin(th1)*sin(th2)*cos(delta - th4)*th2d)/2 + (l4*cos(th2)*sin(th1)*sin(th3)*cos(delta - th4)*th3d)/2 - (l4*cos(th2)*cos(th3)*sin(th1)*sin(delta - th4)*th4d)/2 - (l5*cos(th1)*cos(th2)*cos(th3)*cos(th5)*cos(delta - th4)*th1d)/2 + (l5*cos(th3)*cos(th5)*sin(th1)*sin(th2)*cos(delta - th4)*th2d)/2 + (l5*cos(th2)*cos(th5)*sin(th1)*sin(th3)*cos(delta - th4)*th3d)/2 - (l5*cos(th2)*cos(th3)*cos(th5)*sin(th1)*sin(delta - th4)*th4d)/2 + (l5*cos(th2)*cos(th3)*sin(th1)*sin(th5)*cos(delta - th4)*th5d)/2)*(l2*cos(th1)*cos(th2)*th1d - l2*sin(th1)*sin(th2)*th2d + l3*cos(th1)*cos(th2)*sin(th3)*th1d + l3*cos(th2)*cos(th3)*sin(th1)*th3d - l3*sin(th1)*sin(th2)*sin(th3)*th2d - (l4*sin(th1)*sin(th2)*sin(th3)*cos(delta - th4)*th2d)/2 + (l4*cos(th2)*sin(th1)*sin(th3)*sin(delta - th4)*th4d)/2 + (l4*cos(th1)*cos(th2)*cos(th3)*cos(delta - th4)*th3d)/2 + (l4*cos(th1)*cos(th2)*sin(th3)*cos(delta - th4)*th1d)/2 + (l4*cos(th2)*cos(th3)*sin(th1)*cos(delta - th4)*th3d)/2 - (l4*cos(th2)*sin(th1)*sin(th3)*cos(delta - th4)*th1d)/2 - (l4*cos(th1)*sin(th2)*sin(th3)*cos(delta - th4)*th2d)/2 + (l4*cos(th1)*cos(th2)*sin(th3)*sin(delta - th4)*th4d)/2 + (l5*cos(th1)*cos(th2)*cos(th5)*sin(th3)*cos(delta - th4)*th1d)/2 + (l5*cos(th2)*cos(th3)*cos(th5)*sin(th1)*cos(delta - th4)*th3d)/2 - (l5*cos(th5)*sin(th1)*sin(th2)*sin(th3)*cos(delta - th4)*th2d)/2 + (l5*cos(th2)*cos(th5)*sin(th1)*sin(th3)*sin(delta - th4)*th4d)/2 - (l5*cos(th2)*sin(th1)*sin(th3)*sin(th5)*cos(delta - th4)*th5d)/2)))/2 - beta3*th3d + (m4*(2*((l3*cos(th2 + th3)*(th2d + th3d))/2 + (l3*cos(th2)*cos(th3)*th3d)/2 - (l3*sin(th2)*sin(th3)*th2d)/2 + (l4*cos(delta - th4)*sin(th2 + th3)*th4d)/2 - (l4*sin(delta - th4)*cos(th2 + th3)*(th2d + th3d))/2)*((l3*sin(th2 + th3)*(th2d + th3d))/2 + 2*l2*cos(th2)*th2d + (l3*cos(th3)*sin(th2)*th2d)/2 + (l3*cos(th2)*sin(th3)*th3d)/2 - (l4*cos(delta - th4)*cos(th2 + th3)*th4d)/2 - (l4*sin(delta - th4)*sin(th2 + th3)*(th2d + th3d))/2) + 2*(l3*cos(th2)*cos(th3)*sin(th1)*th1d + l3*cos(th1)*cos(th3)*sin(th2)*th2d + l3*cos(th1)*cos(th2)*sin(th3)*th3d - (l4*cos(th2)*cos(th3)*sin(th1)*cos(delta - th4)*th1d)/2 - (l4*cos(th1)*cos(th3)*sin(th2)*cos(delta - th4)*th2d)/2 - (l4*cos(th1)*cos(th2)*sin(th3)*cos(delta - th4)*th3d)/2 + (l4*cos(th1)*cos(th2)*cos(th3)*sin(delta - th4)*th4d)/2)*(l2*cos(th2)*sin(th1)*th1d + l2*cos(th1)*sin(th2)*th2d - l3*cos(th1)*cos(th2)*cos(th3)*th3d + l3*cos(th2)*sin(th1)*sin(th3)*th1d + l3*cos(th1)*sin(th2)*sin(th3)*th2d + (l4*cos(th1)*cos(th2)*cos(th3)*cos(delta - th4)*th3d)/2 - (l4*cos(th2)*sin(th1)*sin(th3)*cos(delta - th4)*th1d)/2 - (l4*cos(th1)*sin(th2)*sin(th3)*cos(delta - th4)*th2d)/2 + (l4*cos(th1)*cos(th2)*sin(th3)*sin(delta - th4)*th4d)/2) - 2*(- l3*cos(th1)*cos(th2)*cos(th3)*th1d + l3*cos(th3)*sin(th1)*sin(th2)*th2d + l3*cos(th2)*sin(th1)*sin(th3)*th3d + (l4*cos(th2)*cos(th3)*sin(th1)*cos(delta - th4)*th1d)/2 + (l4*cos(th1)*cos(th3)*sin(th2)*cos(delta - th4)*th2d)/2 + (l4*cos(th1)*cos(th2)*sin(th3)*cos(delta - th4)*th3d)/2 - (l4*cos(th1)*cos(th2)*cos(th3)*sin(delta - th4)*th4d)/2)*(l2*cos(th1)*cos(th2)*th1d - l2*sin(th1)*sin(th2)*th2d + l3*cos(th1)*cos(th2)*sin(th3)*th1d + l3*cos(th2)*cos(th3)*sin(th1)*th3d - l3*sin(th1)*sin(th2)*sin(th3)*th2d + (l4*cos(th1)*cos(th2)*cos(th3)*cos(delta - th4)*th3d)/2 - (l4*cos(th2)*sin(th1)*sin(th3)*cos(delta - th4)*th1d)/2 - (l4*cos(th1)*sin(th2)*sin(th3)*cos(delta - th4)*th2d)/2 + (l4*cos(th1)*cos(th2)*sin(th3)*sin(delta - th4)*th4d)/2)))/2 - (m4*(2*((l3*cos(th2 + th3)*(th2d + th3d))/2 + (l3*cos(th2)*cos(th3)*th3d)/2 - (l3*sin(th2)*sin(th3)*th2d)/2 + (l4*cos(delta - th4)*sin(th2 + th3)*th4d)/2 - (l4*sin(delta - th4)*cos(th2 + th3)*(th2d + th3d))/2)*((l3*sin(th2 + th3)*(th2d + th3d))/2 + 2*l2*cos(th2)*th2d + (l3*cos(th3)*sin(th2)*th2d)/2 + (l3*cos(th2)*sin(th3)*th3d)/2 - (l4*cos(delta - th4)*cos(th2 + th3)*th4d)/2 - (l4*sin(delta - th4)*sin(th2 + th3)*(th2d + th3d))/2) - 2*(l3*cos(th2)*cos(th3)*sin(th1) + (l4*cos(th1)*cos(th2)*cos(th3)*cos(delta - th4))/2)*(l2*cos(th2)*sin(th1)*th1d^2 + l2*cos(th2)*sin(th1)*th2d^2 - l2*cos(th1)*cos(th2)*th1dd + l2*sin(th1)*sin(th2)*th2dd + l3*sin(th1)*sin(th2)*sin(th3)*th2dd + l3*cos(th2)*sin(th1)*sin(th3)*th1d^2 + l3*cos(th2)*sin(th1)*sin(th3)*th2d^2 + l3*cos(th2)*sin(th1)*sin(th3)*th3d^2 - l3*cos(th1)*cos(th2)*sin(th3)*th1dd + 2*l2*cos(th1)*sin(th2)*th2d*th1d - 2*l3*cos(th1)*cos(th2)*cos(th3)*th3d*th1d + (l4*cos(th1)*cos(th2)*sin(th3)*cos(delta - th4)*th1d^2)/2 + (l4*cos(th1)*cos(th2)*sin(th3)*cos(delta - th4)*th2d^2)/2 + (l4*cos(th1)*cos(th2)*sin(th3)*cos(delta - th4)*th3d^2)/2 + (l4*cos(th1)*cos(th2)*sin(th3)*cos(delta - th4)*th4d^2)/2 + 2*l3*cos(th1)*sin(th2)*sin(th3)*th2d*th1d + 2*l3*cos(th3)*sin(th1)*sin(th2)*th3d*th2d + (l4*cos(th2)*sin(th1)*sin(th3)*cos(delta - th4)*th1dd)/2 + (l4*cos(th1)*sin(th2)*sin(th3)*cos(delta - th4)*th2dd)/2 - (l4*cos(th1)*cos(th2)*sin(th3)*sin(delta - th4)*th4dd)/2 + l4*cos(th2)*cos(th3)*sin(th1)*cos(delta - th4)*th3d*th1d + l4*cos(th1)*cos(th3)*sin(th2)*cos(delta - th4)*th3d*th2d - l4*cos(th1)*cos(th2)*cos(th3)*sin(delta - th4)*th4d*th3d - l4*sin(th1)*sin(th2)*sin(th3)*cos(delta - th4)*th2d*th1d + l4*cos(th2)*sin(th1)*sin(th3)*sin(delta - th4)*th4d*th1d + l4*cos(th1)*sin(th2)*sin(th3)*sin(delta - th4)*th4d*th2d) + 2*(l3*cos(th2)*cos(th3)*sin(th1)*th1d + l3*cos(th1)*cos(th3)*sin(th2)*th2d + l3*cos(th1)*cos(th2)*sin(th3)*th3d - (l4*cos(th2)*cos(th3)*sin(th1)*cos(delta - th4)*th1d)/2 - (l4*cos(th1)*cos(th3)*sin(th2)*cos(delta - th4)*th2d)/2 - (l4*cos(th1)*cos(th2)*sin(th3)*cos(delta - th4)*th3d)/2 + (l4*cos(th1)*cos(th2)*cos(th3)*sin(delta - th4)*th4d)/2)*(l2*cos(th2)*sin(th1)*th1d + l2*cos(th1)*sin(th2)*th2d - l3*cos(th1)*cos(th2)*cos(th3)*th3d + l3*cos(th2)*sin(th1)*sin(th3)*th1d + l3*cos(th1)*sin(th2)*sin(th3)*th2d + (l4*cos(th1)*cos(th2)*cos(th3)*cos(delta - th4)*th3d)/2 - (l4*cos(th2)*sin(th1)*sin(th3)*cos(delta - th4)*th1d)/2 - (l4*cos(th1)*sin(th2)*sin(th3)*cos(delta - th4)*th2d)/2 + (l4*cos(th1)*cos(th2)*sin(th3)*sin(delta - th4)*th4d)/2) + 2*((l3*sin(th2 + th3))/2 + (l3*cos(th2)*sin(th3))/2 - (l4*sin(delta - th4)*sin(th2 + th3))/2)*(2*l2*cos(th2)*th2dd - 2*l2*sin(th2)*th2d^2 + (l3*cos(th2 + th3)*(th2d + th3d)^2)/2 + (l3*sin(th2 + th3)*th2dd)/2 - (l4*cos(delta - th4)*cos(th2 + th3)*th4dd)/2 - (l4*sin(delta - th4)*cos(th2 + th3)*(th2d + th3d)^2)/2 - (l4*sin(delta - th4)*sin(th2 + th3)*th2dd)/2 + (l3*cos(th2)*cos(th3)*th2d^2)/2 + (l3*cos(th2)*cos(th3)*th3d^2)/2 + (l3*cos(th3)*sin(th2)*th2dd)/2 - (l4*sin(delta - th4)*cos(th2 + th3)*th4d^2)/2 - l3*sin(th2)*sin(th3)*th3d*th2d + l4*cos(delta - th4)*sin(th2 + th3)*(th2d + th3d)*th4d) - 2*(l3*cos(th3)*sin(th1)*sin(th2)*th2d - l3*cos(th1)*cos(th2)*cos(th3)*th1d + l3*cos(th2)*sin(th1)*sin(th3)*th3d + (l4*cos(th2)*cos(th3)*sin(th1)*cos(delta - th4)*th1d)/2 + (l4*cos(th1)*cos(th3)*sin(th2)*cos(delta - th4)*th2d)/2 + (l4*cos(th1)*cos(th2)*sin(th3)*cos(delta - th4)*th3d)/2 - (l4*cos(th1)*cos(th2)*cos(th3)*sin(delta - th4)*th4d)/2)*(l2*cos(th1)*cos(th2)*th1d - l2*sin(th1)*sin(th2)*th2d + l3*cos(th1)*cos(th2)*sin(th3)*th1d + l3*cos(th2)*cos(th3)*sin(th1)*th3d - l3*sin(th1)*sin(th2)*sin(th3)*th2d + (l4*cos(th1)*cos(th2)*cos(th3)*cos(delta - th4)*th3d)/2 - (l4*cos(th2)*sin(th1)*sin(th3)*cos(delta - th4)*th1d)/2 - (l4*cos(th1)*sin(th2)*sin(th3)*cos(delta - th4)*th2d)/2 + (l4*cos(th1)*cos(th2)*sin(th3)*sin(delta - th4)*th4d)/2) - 2*(l3*cos(th1)*cos(th2)*cos(th3) - (l4*cos(th1)*cos(th2)*cos(th3)*cos(delta - th4))/2)*(l2*cos(th1)*cos(th2)*th1d^2 + l2*cos(th1)*cos(th2)*th2d^2 + l2*cos(th2)*sin(th1)*th1dd + l2*cos(th1)*sin(th2)*th2dd + l3*cos(th2)*sin(th1)*sin(th3)*th1dd + l3*cos(th1)*sin(th2)*sin(th3)*th2dd - 2*l2*sin(th1)*sin(th2)*th2d*th1d + l3*cos(th1)*cos(th2)*sin(th3)*th1d^2 + l3*cos(th1)*cos(th2)*sin(th3)*th2d^2 + l3*cos(th1)*cos(th2)*sin(th3)*th3d^2 + 2*l3*cos(th2)*cos(th3)*sin(th1)*th3d*th1d + 2*l3*cos(th1)*cos(th3)*sin(th2)*th3d*th2d - (l4*cos(th1)*cos(th2)*sin(th3)*cos(delta - th4)*th1d^2)/2 - (l4*cos(th1)*cos(th2)*sin(th3)*cos(delta - th4)*th2d^2)/2 - (l4*cos(th1)*cos(th2)*sin(th3)*cos(delta - th4)*th3d^2)/2 - (l4*cos(th1)*cos(th2)*sin(th3)*cos(delta - th4)*th4d^2)/2 - 2*l3*sin(th1)*sin(th2)*sin(th3)*th2d*th1d - (l4*cos(th2)*sin(th1)*sin(th3)*cos(delta - th4)*th1dd)/2 - (l4*cos(th1)*sin(th2)*sin(th3)*cos(delta - th4)*th2dd)/2 + (l4*cos(th1)*cos(th2)*sin(th3)*sin(delta - th4)*th4dd)/2 - l4*cos(th2)*cos(th3)*sin(th1)*cos(delta - th4)*th3d*th1d - l4*cos(th1)*cos(th3)*sin(th2)*cos(delta - th4)*th3d*th2d + l4*cos(th1)*cos(th2)*cos(th3)*sin(delta - th4)*th4d*th3d + l4*sin(th1)*sin(th2)*sin(th3)*cos(delta - th4)*th2d*th1d - l4*cos(th2)*sin(th1)*sin(th3)*sin(delta - th4)*th4d*th1d - l4*cos(th1)*sin(th2)*sin(th3)*sin(delta - th4)*th4d*th2d)))/2 - (m5*(2*((l3*cos(th2 + th3)*(th2d + th3d))/2 + (l3*cos(th2)*cos(th3)*th3d)/2 - (l3*sin(th2)*sin(th3)*th2d)/2 + (l4*cos(delta - th4)*sin(th2 + th3)*th4d)/2 - (l4*sin(delta - th4)*cos(th2 + th3)*(th2d + th3d))/2 - (l4*cos(th2)*cos(th3)*sin(delta - th4)*th3d)/2 + (l4*cos(th2)*sin(th3)*cos(delta - th4)*th4d)/2 + (l4*sin(th2)*sin(th3)*sin(delta - th4)*th2d)/2 + (l5*sin(th2)*sin(th3)*sin(th5)*sin(delta - th4)*th2d)/2 - (l5*cos(th2)*cos(th3)*sin(th5)*sin(delta - th4)*th3d)/2 + (l5*cos(th2)*sin(th3)*sin(th5)*cos(delta - th4)*th4d)/2 - (l5*cos(th2)*cos(th5)*sin(th3)*sin(delta - th4)*th5d)/2)*(- (l3*sin(th2 + th3)*(th2d + th3d))/2 - 2*l2*cos(th2)*th2d - (l3*cos(th3)*sin(th2)*th2d)/2 - (l3*cos(th2)*sin(th3)*th3d)/2 + (l4*cos(delta - th4)*cos(th2 + th3)*th4d)/2 + (l4*sin(delta - th4)*sin(th2 + th3)*(th2d + th3d))/2 + (l4*cos(th2)*cos(th3)*cos(delta - th4)*th4d)/2 + (l4*cos(th3)*sin(th2)*sin(delta - th4)*th2d)/2 + (l4*cos(th2)*sin(th3)*sin(delta - th4)*th3d)/2 + (l5*cos(th3)*sin(th2)*sin(th5)*sin(delta - th4)*th2d)/2 + (l5*cos(th2)*sin(th3)*sin(th5)*sin(delta - th4)*th3d)/2 + (l5*cos(th2)*cos(th3)*sin(th5)*cos(delta - th4)*th4d)/2 - (l5*cos(th2)*cos(th3)*cos(th5)*sin(delta - th4)*th5d)/2) + 2*(- l3*cos(th2)*cos(th3)*sin(th1)*th1d - l3*cos(th1)*cos(th3)*sin(th2)*th2d - l3*cos(th1)*cos(th2)*sin(th3)*th3d + l4*cos(th2)*cos(th3)*sin(th1)*cos(delta - th4)*th1d + l4*cos(th1)*cos(th3)*sin(th2)*cos(delta - th4)*th2d + l4*cos(th1)*cos(th2)*sin(th3)*cos(delta - th4)*th3d - l4*cos(th1)*cos(th2)*cos(th3)*sin(delta - th4)*th4d + (l5*cos(th2)*cos(th3)*cos(th5)*sin(th1)*cos(delta - th4)*th1d)/2 + (l5*cos(th1)*cos(th3)*cos(th5)*sin(th2)*cos(delta - th4)*th2d)/2 + (l5*cos(th1)*cos(th2)*cos(th5)*sin(th3)*cos(delta - th4)*th3d)/2 - (l5*cos(th1)*cos(th2)*cos(th3)*cos(th5)*sin(delta - th4)*th4d)/2 + (l5*cos(th1)*cos(th2)*cos(th3)*sin(th5)*cos(delta - th4)*th5d)/2)*(l2*cos(th2)*sin(th1)*th1d + l2*cos(th1)*sin(th2)*th2d - l3*cos(th1)*cos(th2)*cos(th3)*th3d + l3*cos(th2)*sin(th1)*sin(th3)*th1d + l3*cos(th1)*sin(th2)*sin(th3)*th2d + l4*cos(th1)*cos(th2)*cos(th3)*cos(delta - th4)*th3d - l4*cos(th2)*sin(th1)*sin(th3)*cos(delta - th4)*th1d - l4*cos(th1)*sin(th2)*sin(th3)*cos(delta - th4)*th2d + l4*cos(th1)*cos(th2)*sin(th3)*sin(delta - th4)*th4d + (l5*cos(th1)*cos(th2)*cos(th3)*cos(th5)*cos(delta - th4)*th3d)/2 - (l5*cos(th2)*cos(th5)*sin(th1)*sin(th3)*cos(delta - th4)*th1d)/2 - (l5*cos(th1)*cos(th5)*sin(th2)*sin(th3)*cos(delta - th4)*th2d)/2 + (l5*cos(th1)*cos(th2)*cos(th5)*sin(th3)*sin(delta - th4)*th4d)/2 - (l5*cos(th1)*cos(th2)*sin(th3)*sin(th5)*cos(delta - th4)*th5d)/2) + 2*(- l3*cos(th1)*cos(th2)*cos(th3)*th1d + l3*cos(th3)*sin(th1)*sin(th2)*th2d + l3*cos(th2)*sin(th1)*sin(th3)*th3d - (l4*cos(th1)*cos(th2)*cos(th3)*cos(delta - th4)*th1d)/2 + (l4*cos(th2)*cos(th3)*sin(th1)*cos(delta - th4)*th1d)/2 + (l4*cos(th1)*cos(th3)*sin(th2)*cos(delta - th4)*th2d)/2 + (l4*cos(th1)*cos(th2)*sin(th3)*cos(delta - th4)*th3d)/2 - (l4*cos(th1)*cos(th2)*cos(th3)*sin(delta - th4)*th4d)/2 + (l4*cos(th3)*sin(th1)*sin(th2)*cos(delta - th4)*th2d)/2 + (l4*cos(th2)*sin(th1)*sin(th3)*cos(delta - th4)*th3d)/2 - (l4*cos(th2)*cos(th3)*sin(th1)*sin(delta - th4)*th4d)/2 - (l5*cos(th1)*cos(th2)*cos(th3)*cos(th5)*cos(delta - th4)*th1d)/2 + (l5*cos(th3)*cos(th5)*sin(th1)*sin(th2)*cos(delta - th4)*th2d)/2 + (l5*cos(th2)*cos(th5)*sin(th1)*sin(th3)*cos(delta - th4)*th3d)/2 - (l5*cos(th2)*cos(th3)*cos(th5)*sin(th1)*sin(delta - th4)*th4d)/2 + (l5*cos(th2)*cos(th3)*sin(th1)*sin(th5)*cos(delta - th4)*th5d)/2)*(l2*cos(th1)*cos(th2)*th1d - l2*sin(th1)*sin(th2)*th2d + l3*cos(th1)*cos(th2)*sin(th3)*th1d + l3*cos(th2)*cos(th3)*sin(th1)*th3d - l3*sin(th1)*sin(th2)*sin(th3)*th2d - (l4*sin(th1)*sin(th2)*sin(th3)*cos(delta - th4)*th2d)/2 + (l4*cos(th2)*sin(th1)*sin(th3)*sin(delta - th4)*th4d)/2 + (l4*cos(th1)*cos(th2)*cos(th3)*cos(delta - th4)*th3d)/2 + (l4*cos(th1)*cos(th2)*sin(th3)*cos(delta - th4)*th1d)/2 + (l4*cos(th2)*cos(th3)*sin(th1)*cos(delta - th4)*th3d)/2 - (l4*cos(th2)*sin(th1)*sin(th3)*cos(delta - th4)*th1d)/2 - (l4*cos(th1)*sin(th2)*sin(th3)*cos(delta - th4)*th2d)/2 + (l4*cos(th1)*cos(th2)*sin(th3)*sin(delta - th4)*th4d)/2 + (l5*cos(th1)*cos(th2)*cos(th5)*sin(th3)*cos(delta - th4)*th1d)/2 + (l5*cos(th2)*cos(th3)*cos(th5)*sin(th1)*cos(delta - th4)*th3d)/2 - (l5*cos(th5)*sin(th1)*sin(th2)*sin(th3)*cos(delta - th4)*th2d)/2 + (l5*cos(th2)*cos(th5)*sin(th1)*sin(th3)*sin(delta - th4)*th4d)/2 - (l5*cos(th2)*sin(th1)*sin(th3)*sin(th5)*cos(delta - th4)*th5d)/2)))/2 - (m3*(l3*sin(th2 + th3)*(- 2*l2*sin(th2)*th2d^2 + 2*l2*cos(th2)*th2dd + (l3*cos(th2 + th3)*(th2d + th3d)^2)/2 + (l3*sin(th2 + th3)*th2dd)/2) + l3*cos(th2 + th3)*((l3*sin(th2 + th3)*(th2d + th3d))/2 + 2*l2*cos(th2)*th2d)*(th2d + th3d) - l3*cos(th2)*cos(th3)*sin(th1)*(l2*cos(th2)*sin(th1)*th1d^2 + l2*cos(th2)*sin(th1)*th2d^2 - l2*cos(th1)*cos(th2)*th1dd + l2*sin(th1)*sin(th2)*th2dd + (l3*sin(th1)*sin(th2)*sin(th3)*th2dd)/2 + (l3*cos(th2)*sin(th1)*sin(th3)*th1d^2)/2 + (l3*cos(th2)*sin(th1)*sin(th3)*th2d^2)/2 + (l3*cos(th2)*sin(th1)*sin(th3)*th3d^2)/2 - (l3*cos(th1)*cos(th2)*sin(th3)*th1dd)/2 + 2*l2*cos(th1)*sin(th2)*th2d*th1d - l3*cos(th1)*cos(th2)*cos(th3)*th3d*th1d + l3*cos(th1)*sin(th2)*sin(th3)*th2d*th1d + l3*cos(th3)*sin(th1)*sin(th2)*th3d*th2d) - l3*cos(th1)*cos(th2)*cos(th3)*(l2*cos(th1)*cos(th2)*th1d^2 + l2*cos(th1)*cos(th2)*th2d^2 + l2*cos(th2)*sin(th1)*th1dd + l2*cos(th1)*sin(th2)*th2dd + (l3*cos(th2)*sin(th1)*sin(th3)*th1dd)/2 + (l3*cos(th1)*sin(th2)*sin(th3)*th2dd)/2 - 2*l2*sin(th1)*sin(th2)*th2d*th1d + (l3*cos(th1)*cos(th2)*sin(th3)*th1d^2)/2 + (l3*cos(th1)*cos(th2)*sin(th3)*th2d^2)/2 + (l3*cos(th1)*cos(th2)*sin(th3)*th3d^2)/2 + l3*cos(th2)*cos(th3)*sin(th1)*th3d*th1d + l3*cos(th1)*cos(th3)*sin(th2)*th3d*th2d - l3*sin(th1)*sin(th2)*sin(th3)*th2d*th1d) + l3*cos(th2)*cos(th3)*sin(th1)*(l2*cos(th2)*sin(th1)*th1d + l2*cos(th1)*sin(th2)*th2d - (l3*cos(th1)*cos(th2)*cos(th3)*th3d)/2 + (l3*cos(th2)*sin(th1)*sin(th3)*th1d)/2 + (l3*cos(th1)*sin(th2)*sin(th3)*th2d)/2)*th1d + l3*cos(th1)*cos(th2)*cos(th3)*(l2*cos(th1)*cos(th2)*th1d - l2*sin(th1)*sin(th2)*th2d + (l3*cos(th1)*cos(th2)*sin(th3)*th1d)/2 + (l3*cos(th2)*cos(th3)*sin(th1)*th3d)/2 - (l3*sin(th1)*sin(th2)*sin(th3)*th2d)/2)*th1d + l3*cos(th1)*cos(th3)*sin(th2)*(l2*cos(th2)*sin(th1)*th1d + l2*cos(th1)*sin(th2)*th2d - (l3*cos(th1)*cos(th2)*cos(th3)*th3d)/2 + (l3*cos(th2)*sin(th1)*sin(th3)*th1d)/2 + (l3*cos(th1)*sin(th2)*sin(th3)*th2d)/2)*th2d + l3*cos(th1)*cos(th2)*sin(th3)*(l2*cos(th2)*sin(th1)*th1d + l2*cos(th1)*sin(th2)*th2d - (l3*cos(th1)*cos(th2)*cos(th3)*th3d)/2 + (l3*cos(th2)*sin(th1)*sin(th3)*th1d)/2 + (l3*cos(th1)*sin(th2)*sin(th3)*th2d)/2)*th3d - l3*cos(th3)*sin(th1)*sin(th2)*(l2*cos(th1)*cos(th2)*th1d - l2*sin(th1)*sin(th2)*th2d + (l3*cos(th1)*cos(th2)*sin(th3)*th1d)/2 + (l3*cos(th2)*cos(th3)*sin(th1)*th3d)/2 - (l3*sin(th1)*sin(th2)*sin(th3)*th2d)/2)*th2d - l3*cos(th2)*sin(th1)*sin(th3)*(l2*cos(th1)*cos(th2)*th1d - l2*sin(th1)*sin(th2)*th2d + (l3*cos(th1)*cos(th2)*sin(th3)*th1d)/2 + (l3*cos(th2)*cos(th3)*sin(th1)*th3d)/2 - (l3*sin(th1)*sin(th2)*sin(th3)*th2d)/2)*th3d))/2 - g*m5*(l4*cos(th2)*sin(th3)*sin(delta - th4) - l3*cos(th2)*sin(th3) + (l5*cos(th2)*sin(th3)*sin(delta - th4))/2) + g*m4*(l3*cos(th2)*sin(th3) - (l4*cos(th2)*sin(th3)*sin(delta - th4))/2) + (g*l3*m3*cos(th2)*sin(th3))/2)/(l3_Izz + l4_Izz + l5_Izz + (m4*(2*(l3*cos(th1)*cos(th2)*cos(th3) - (l4*cos(th1)*cos(th2)*cos(th3)*cos(delta - th4))/2)^2 + 2*((l3*sin(th2 + th3))/2 + (l3*cos(th2)*sin(th3))/2 - (l4*sin(delta - th4)*sin(th2 + th3))/2)^2 + 2*(l3*cos(th2)*cos(th3)*sin(th1) + (l4*cos(th1)*cos(th2)*cos(th3)*cos(delta - th4))/2)^2))/2 + (m5*(2*(l3*cos(th2)*cos(th3)*sin(th1) + (l4*cos(th1)*cos(th2)*cos(th3)*cos(delta - th4))/2 + (l4*cos(th2)*cos(th3)*sin(th1)*cos(delta - th4))/2 + (l5*cos(th2)*cos(th3)*cos(th5)*sin(th1)*cos(delta - th4))/2)^2 + 2*((l4*sin(delta - th4)*sin(th2 + th3))/2 - (l3*cos(th2)*sin(th3))/2 - (l3*sin(th2 + th3))/2 + (l4*cos(th2)*sin(th3)*sin(delta - th4))/2 + (l5*cos(th2)*sin(th3)*sin(th5)*sin(delta - th4))/2)^2 + 2*(l4*cos(th1)*cos(th2)*cos(th3)*cos(delta - th4) - l3*cos(th1)*cos(th2)*cos(th3) + (l5*cos(th1)*cos(th2)*cos(th3)*cos(th5)*cos(delta - th4))/2)^2))/2 + (m3*((l3^2*cos(th1)^2*cos(th2)^2*cos(th3)^2)/2 + (l3^2*cos(th2)^2*cos(th3)^2*sin(th1)^2)/2 + (l3^2*sin(th2 + th3)^2)/2))/2);
 
